simulink model "DynamicsAaa"  (R2017a)
settings: Solver=VariableStepAuto  StartTime=0.0  StopTime=200  RelTol=1e-3
(part 2 of 8)

== matlab function DynamicsAaa/torque ==
  data: q input; qd input; q_des input; torque output; q_des_dot input; q_des_ddot input
function torque = fcn(q,qd,q_des,q_des_dot,q_des_ddot)
%#codegen

%% Constant
% syms qd(1) qd(2) qd(3) qd(4) qd(5) qd(6)
% syms qdd(1) qdd(2) qdd(3) qdd(4) qdd(5) qdd(6)

g = 9.8;


m2=26.9797
m3=15.9204
m4=25.8524
m5=4.08846
m6=1.61544
m7=0.0160103

Kp = 20;
Kd = 10;
%% Triangle relative

c1 = cos(q(1));
c2 = cos(q(2));
c3 = cos(q(3));
c4 = cos(q(4));
c5 = cos(q(5));
c6 = cos(q(6));
s1 = sin(q(1));
s2 = sin(q(2));
s3 = sin(q(3));
s4 = sin(q(4));
s5 = sin(q(5));
s6 = sin(q(6));
c23 = cos(q(2)+q(3)); 
c12 = cos(q(1)+q(2)); 
s23 = sin(q(2)+q(3));
s123 = sin(q(1)+q(2)+q(3));
c123 = cos(q(1)+q(2)+q(3));
c1 = cos(q(1));
c2 = cos(q(2));
c3 = cos(q(3));
c23 = cos(q(2)+q(3)); 
c12 = cos(q(1)+q(2)); 
s1 = sin(q(1));
s2 = sin(q(2));
s3 = sin(q(3));
s23 = sin(q(2)+q(3));
s123 = sin(q(1)+q(2)+q(3));
c123 = cos(q(1)+q(2)+q(3));
%% tau
% tau0 = 0;
% 
% tau1 = -335*c2*(c3*(c4*(c5*m7*(80*c6*(-c5*(-qdd(3) + qdd(4)) - qd(5)*(c5*(-c3*s4*(qd(1) + qd(2)) + c4*s3*(qd(1) + qd(2))) - s5*(-qd(3) + qd(4))) - s5*(c4*(c3*qd(3)*(qd(1) + qd(2)) + s3*(qdd(1) + qdd(2))) + qd(4)*(-c3*c4*(qd(1) + qd(2)) - s3*s4*(qd(1) + qd(2))) - s4*(c3*(qdd(1) + qdd(2)) - qd(3)*s3*(qd(1) + qd(2))))) + c6*(80*c5*(-qdd(3) + qdd(4)) + c5*(c4*(-295*c3*(qdd(1) + qdd(2)) + c3*(c2*(-g*s1 - 270*qd(1)^2) + s2*(-c1*g + 270*qdd(1)) - (qd(1) + qd(2))*(90*qd(1) + 90*qd(2)))) - s4*(295*s3*(qdd(1) + qdd(2)) - s3*(c2*(-g*s1 - 270*qd(1)^2) + s2*(-c1*g + 270*qdd(1)) - (qd(1) + qd(2))*(90*qd(1) + 90*qd(2))))) + 80*qd(5)*(c5*(-c3*s4*(qd(1) + qd(2)) + c4*s3*(qd(1) + qd(2))) - s5*(-qd(3) + qd(4))) + 80*s5*(c4*(c3*qd(3)*(qd(1) + qd(2)) + s3*(qdd(1) + qdd(2))) + qd(4)*(-c3*c4*(qd(1) + qd(2)) - s3*s4*(qd(1) + qd(2))) - s4*(c3*(qdd(1) + qdd(2)) - qd(3)*s3*(qd(1) + qd(2)))) - s5*(-c2*(-c1*g + 270*qdd(1)) - 295*c3^2*(qd(1) + qd(2))^2 - 90*qdd(1) - 90*qdd(2) + s2*(-g*s1 - 270*qd(1)^2) - 295*s3^2*(qd(1) + qd(2))^2) - (80*c5*(-c3*s4*(qd(1) + qd(2)) + c4*s3*(qd(1) + qd(2))) - 80*s5*(-qd(3) + qd(4)))*(-c3*c4*(qd(1) + qd(2)) + qd(5) - s3*s4*(qd(1) + qd(2)))) + 80*qd(6)*(c6*(c5*(-c3*s4*(qd(1) + qd(2)) + c4*s3*(qd(1) + qd(2))) - s5*(-qd(3) + qd(4))) - s6*(-c5*(-qd(3) + qd(4)) - s5*(-c3*s4*(qd(1) + qd(2)) + c4*s3*(qd(1) + qd(2))))) + 80*s6*(c5*(c4*(c3*qd(3)*(qd(1) + qd(2)) + s3*(qdd(1) + qdd(2))) + qd(4)*(-c3*c4*(qd(1) + qd(2)) - s3*s4*(qd(1) + qd(2))) - s4*(c3*(qdd(1) + qdd(2)) - qd(3)*s3*(qd(1) + qd(2)))) + qd(5)*(-c5*(-qd(3) + qd(4)) - s5*(-c3*s4*(qd(1) + qd(2)) + c4*s3*(qd(1) + qd(2)))) - s5*(-qdd(3) + qdd(4))) - s6*(80*c5*(c4*(c3*qd(3)*(qd(1) + qd(2)) + s3*(qdd(1) + qdd(2))) + qd(4)*(-c3*c4*(qd(1) + qd(2)) - s3*s4*(qd(1) + qd(2))) - s4*(c3*(qdd(1) + qdd(2)) - qd(3)*s3*(qd(1) + qd(2)))) - c5*(-c2*(-c1*g + 270*qdd(1)) - 295*c3^2*(qd(1) + qd(2))^2 - 90*qdd(1) - 90*qdd(2) + s2*(-g*s1 - 270*qd(1)^2) - 295*s3^2*(qd(1) + qd(2))^2) + 80*qd(5)*(-c5*(-qd(3) + qd(4)) - s5*(-c3*s4*(qd(1) + qd(2)) + c4*s3*(qd(1) + qd(2)))) - 80*s5*(-qdd(3) + qdd(4)) - s5*(c4*(-295*c3*(qdd(1) + qdd(2)) + c3*(c2*(-g*s1 - 270*qd(1)^2) + s2*(-c1*g + 270*qdd(1)) - (qd(1) + qd(2))*(90*qd(1) + 90*qd(2)))) - s4*(295*s3*(qdd(1) + qdd(2)) - s3*(c2*(-g*s1 - 270*qd(1)^2) + s2*(-c1*g + 270*qdd(1)) - (qd(1) + qd(2))*(90*qd(1) + 90*qd(2))))) + (80*c5*(-qd(3) + qd(4)) + 80*s5*(-c3*s4*(qd(1) + qd(2)) + c4*s3*(qd(1) + qd(2))))*(-c3*c4*(qd(1) + qd(2)) + qd(5) - s3*s4*(qd(1) + qd(2)))) - (80*c6*(c5*(-c3*s4*(qd(1) + qd(2)) + c4*s3*(qd(1) + qd(2))) - s5*(-qd(3) + qd(4))) - 80*s6*(-c5*(-qd(3) + qd(4)) - s5*(-c3*s4*(qd(1) + qd(2)) + c4*s3*(qd(1) + qd(2)))))*(c3*c4*(qd(1) + qd(2)) - qd(5) + qd(6) + s3*s4*(qd(1) + qd(2)))) + m6*(c5*(c4*(-295*c3*(qdd(1) + qdd(2)) + c3*(c2*(-g*s1 - 270*qd(1)^2) + s2*(-c1*g + 270*qdd(1)) - (qd(1) + qd(2))*(90*qd(1) + 90*qd(2)))) - s4*(295*s3*(qdd(1) + qdd(2)) - s3*(c2*(-g*s1 - 270*qd(1)^2) + s2*(-c1*g + 270*qdd(1)) - (qd(1) + qd(2))*(90*qd(1) + 90*qd(2))))) - s5*(-c2*(-c1*g + 270*qdd(1)) - 295*c3^2*(qd(1) + qd(2))^2 - 90*qdd(1) - 90*qdd(2) + s2*(-g*s1 - 270*qd(1)^2) - 295*s3^2*(qd(1) + qd(2))^2)) - m7*s5*(80*c6*(c5*(c4*(c3*qd(3)*(qd(1) + qd(2)) + s3*(qdd(1) + qdd(2))) + qd(4)*(-c3*c4*(qd(1) + qd(2)) - s3*s4*(qd(1) + qd(2))) - s4*(c3*(qdd(1) + qdd(2)) - qd(3)*s3*(qd(1) + qd(2)))) + qd(5)*(-c5*(-qd(3) + qd(4)) - s5*(-c3*s4*(qd(1) + qd(2)) + c4*s3*(qd(1) + qd(2)))) - s5*(-qdd(3) + qdd(4))) - c6*(80*c5*(c4*(c3*qd(3)*(qd(1) + qd(2)) + s3*(qdd(1) + qdd(2))) + qd(4)*(-c3*c4*(qd(1) + qd(2)) - s3*s4*(qd(1) + qd(2))) - s4*(c3*(qdd(1) + qdd(2)) - qd(3)*s3*(qd(1) + qd(2)))) - c5*(-c2*(-c1*g + 270*qdd(1)) - 295*c3^2*(qd(1) + qd(2)) ^2 - 90*qdd(1) - 90*qdd(2) + s2*(-g*s1 - 270*qd(1)^2) - 295*s3^2*(qd(1) + qd(2)) ^2) + 80*qd(5)*(-c5*(-qd(3) + qd(4)) - s5*(-c3*s4*(qd(1) + qd(2)) + c4*s3*(qd(1) + qd(2)))) - 80*s5*(-qdd(3) + qdd(4)) - s5*(c4*(-295*c3*(qdd(1) + qdd(2)) + c3*(c2*(-g*s1 - 270*qd(1)^2) + s2*(-c1*g + 270*qdd(1)) - (qd(1) + qd(2))*(90*qd(1) + 90*qd(2)))) - s4*(295*s3*(qdd(1) + qdd(2)) - s3*(c2*(-g*s1 - 270*qd(1)^2) + s2*(-c1*g + 270*qdd(1)) - (qd(1) + qd(2))*(90*qd(1) + 90*qd(2))))) + (80*c5*(-qd(3) + qd(4)) + 80*s5*(-c3*s4*(qd(1) + qd(2)) + c4*s3*(qd(1) + qd(2))))*(-c3*c4*(qd(1) + qd(2)) + qd(5) - s3*s4*(qd(1) + qd(2)))) + 80*qd(6)*(-c6*(-c5*(-qd(3) + qd(4)) - s5*(-c3*s4*(qd(1) + qd(2)) + c4*s3*(qd(1) + qd(2)))) - s6*(c5*(-c3*s4*(qd(1) + qd(2)) + c4*s3*(qd(1) + qd(2))) - s5*(-qd(3) + qd(4)))) - 80*s6*(-c5*(-qdd(3) + qdd(4)) - qd(5)*(c5*(-c3*s4*(qd(1) + qd(2)) + c4*s3*(qd(1) + qd(2))) - s5*(-qd(3) + qd(4))) - s5*(c4*(c3*qd(3)*(qd(1) + qd(2)) + s3*(qdd(1) + qdd(2))) + qd(4)*(-c3*c4*(qd(1) + qd(2)) - s3*s4*(qd(1) + qd(2))) - s4*(c3*(qdd(1) + qdd(2)) - qd(3)*s3*(qd(1) + qd(2))))) - s6*(80*c5*(-qdd(3) + qdd(4)) + c5*(c4*(-295*c3*(qdd(1) + qdd(2)) + c3*(c2*(-g*s1 - 270*qd(1)^2) + s2*(-c1*g + 270*qdd(1)) - (qd(1) + qd(2))*(90*qd(1) + 90*qd(2)))) - s4*(295*s3*(qdd(1) + qdd(2)) - s3*(c2*(-g*s1 - 270*qd(1)^2) + s2*(-c1*g + 270*qdd(1)) - (qd(1) + qd(2))*(90*qd(1) + 90*qd(2))))) + 80*qd(5)*(c5*(-c3*s4*(qd(1) + qd(2)) + c4*s3*(qd(1) + qd(2))) - s5*(-qd(3) + qd(4))) + 80*s5*(c4*(c3*qd(3)*(qd(1) + qd(2)) + s3*(qdd(1) + qdd(2))) + qd(4)*(-c3*c4*(qd(1) + qd(2)) - s3*s4*(qd(1) + qd(2))) - s4*(c3*(qdd(1) + qdd(2)) - qd(3)*s3*(qd(1) + qd(2)))) - s5*(-c2*(-c1*g + 270*qdd(1)) - 295*c3^2*(qd(1) + qd(2)) ^2 - 90*qdd(1) - 90*qdd(2) + s2*(-g*s1 - 270*qd(1)^2) - 295*s3^2*(qd(1) + qd(2)) ^2) - (80*c5*(-c3*s4*(qd(1) + qd(2)) + c4*s3*(qd(1) + qd(2))) - 80*s5*(-qd(3) + qd(4)))*(-c3*c4*(qd(1) + qd(2)) + qd(5) - s3*s4*(qd(1) + qd(2)))) + (80*c6*(-c5*(-qd(3) + qd(4)) - s5*(-c3*s4*(qd(1) + qd(2)) + c4*s3*(qd(1) + qd(2)))) + 80*s6*(c5*(-c3*s4*(qd(1) + qd(2)) + c4*s3*(qd(1) + qd(2))) - s5*(-qd(3) + qd(4))))*(c3*c4*(qd(1) + qd(2)) - qd(5) + qd(6) + s3*s4*(qd(1) + qd(2))))) + m5*(c4*(-295*c3*(qdd(1) + qdd(2)) + c3*(c2*(-g*s1 - 270*qd(1)^2) + s2*(-c1*g + 270*qdd(1)) - (qd(1) + qd(2))*(90*qd(1) + 90*qd(2)))) + 295*c4*(c3*(qdd(1) + qdd(2)) - qd(3)*s3*(qd(1) + qd(2))) + 295*qd(4)*(-c3*s4*(qd(1) + qd(2)) + c4*s3*(qd(1) + qd(2))) - s4*(295*s3*(qdd(1) + qdd(2)) - s3*(c2*(-g*s1 - 270*qd(1)^2) + s2*(-c1*g + 270*qdd(1)) - (qd(1) + qd(2))*(90*qd(1) + 90*qd(2)))) + 295*s4*(c3*qd(3)*(qd(1) + qd(2)) + s3*(qdd(1) + qdd(2))) - (-qd(3) + qd(4))*(-295*c3*s4*(qd(1) + qd(2)) + 295*c4*s3*(qd(1) + qd(2)))) - s4*(m6*(-c5*(-c2*(-c1*g + 270*qdd(1)) - 295*c3^2*(qd(1) + qd(2)) ^2 - 90*qdd(1) - 90*qdd(2) + s2*(-g*s1 - 270*qd(1)^2) - 295*s3^2*(qd(1) + qd(2)) ^2) - s5*(c4*(-295*c3*(qdd(1) + qdd(2)) + c3*(c2*(-g*s1 - 270*qd(1)^2) + s2*(-c1*g + 270*qdd(1)) - (qd(1) + qd(2))*(90*qd(1) + 90*qd(2)))) - s4*(295*s3*(qdd(1) + qdd(2)) - s3*(c2*(-g*s1 - 270*qd(1)^2) + s2*(-c1*g + 270*qdd(1)) - (qd(1) + qd(2))*(90*qd(1) + 90*qd(2)))))) + m7*(c4*(295*s3*(qdd(1) + qdd(2)) - s3*(c2*(-g*s1 - 270*qd(1)^2) + s2*(-c1*g + 270*qdd(1)) - (qd(1) + qd(2))*(90*qd(1) + 90*qd(2)))) + s4*(-295*c3*(qdd(1) + qdd(2)) + c3*(c2*(-g*s1 - 270*qd(1)^2) + s2*(-c1*g + 270*qdd(1)) - (qd(1) + qd(2))*(90*qd(1) + 90*qd(2)))) + (-c5*(-qd(3) + qd(4)) - s5*(-c3*s4*(qd(1) + qd(2)) + c4*s3*(qd(1) + qd(2))))*(80*c5*(-qd(3) + qd(4)) + 80*s5*(-c3*s4*(qd(1) + qd(2)) + c4*s3*(qd(1) + qd(2)))) - (c5*(-c3*s4*(qd(1) + qd(2)) + c4*s3*(qd(1) + qd(2))) - s5*(-qd(3) + qd(4)))*(80*c5*(-c3*s4*(qd(1) + qd(2)) + c4*s3*(qd(1) + qd(2))) - 80*s5*(-qd(3) + qd(4))) - (-c6*(-c5*(-qd(3) + qd(4)) - s5*(-c3*s4*(qd(1) + qd(2)) + c4*s3*(qd(1) + qd(2)))) - s6*(c5*(-c3*s4*(qd(1) + qd(2)) + c4*s3*(qd(1) + qd(2))) - s5*(-qd(3) + qd(4))))*(80*c6*(-c5*(-qd(3) + qd(4)) - s5*(-c3*s4*(qd(1) + qd(2)) + c4*s3*(qd(1) + qd(2)))) + 80*s6*(c5*(-c3*s4*(qd(1) + qd(2)) + c4*s3*(qd(1) + qd(2))) - s5*(-qd(3) + qd(4)))) + (c6*(c5*(-c3*s4*(qd(1) + qd(2)) + c4*s3*(qd(1) + qd(2))) - s5*(-qd(3) + qd(4))) - s6*(-c5*(-qd(3) + qd(4)) - s5*(-c3*s4*(qd(1) + qd(2)) + c4*s3*(qd(1) + qd(2)))))*(80*c6*(c5*(-c3*s4*(qd(1) + qd(2)) + c4*s3*(qd(1) + qd(2))) - s5*(-qd(3) + qd(4))) - 80*s6*(-c5*(-qd(3) + qd(4)) - s5*(-c3*s4*(qd(1) + qd(2)) + c4*s3*(qd(1) + qd(2)))))))) + m4*(-90*c3^2*(qd(1) + qd(2)) ^2 + c3*(c2*(-g*s1 - 270*qd(1)^2) + s2*(-c1*g + 270*qdd(1)) - (qd(1) + qd(2))*(90*qd(1) + 90*qd(2))) - 90*qd(3)^2) - s3*(-c4*(m6*(-c5*(-c2*(-c1*g + 270*qdd(1)) - 295*c3^2*(qd(1) + qd(2)) ^2 - 90*qdd(1) - 90*qdd(2) + s2*(-g*s1 - 270*qd(1)^2) - 295*s3^2*(qd(1) + qd(2)) ^2) - s5*(c4*(-295*c3*(qdd(1) + qdd(2)) + c3*(c2*(-g*s1 - 270*qd(1)^2) + s2*(-c1*g + 270*qdd(1)) - (qd(1) + qd(2))*(90*qd(1) + 90*qd(2)))) - s4*(295*s3*(qdd(1) + qdd(2)) - s3*(c2*(-g*s1 - 270*qd(1)^2) + s2*(-c1*g + 270*qdd(1)) - (qd(1) + qd(2))*(90*qd(1) + 90*qd(2)))))) + m7*(c4*(295*s3*(qdd(1) + qdd(2)) - s3*(c2*(-g*s1 - 270*qd(1)^2) + s2*(-c1*g + 270*qdd(1)) - (qd(1) + qd(2))*(90*qd(1) + 90*qd(2)))) + s4*(-295*c3*(qdd(1) + qdd(2)) + c3*(c2*(-g*s1 - 270*qd(1)^2) + s2*(-c1*g + 270*qdd(1)) - (qd(1) + qd(2))*(90*qd(1) + 90*qd(2)))) + (-c5*(-qd(3) + qd(4)) - s5*(-c3*s4*(qd(1) + qd(2)) + c4*s3*(qd(1) + qd(2))))*(80*c5*(-qd(3) + qd(4)) + 80*s5*(-c3*s4*(qd(1) + qd(2)) + c4*s3*(qd(1) + qd(2)))) - (c5*(-c3*s4*(qd(1) + qd(2)) + c4*s3*(qd(1) + qd(2))) - s5*(-qd(3) + qd(4)))*(80*c5*(-c3*s4*(qd(1) + qd(2)) + c4*s3*(qd(1) + qd(2))) - 80*s5*(-qd(3) + qd(4))) - (-c6*(-c5*(-qd(3) + qd(4)) - s5*(-c3*s4*(qd(1) + qd(2)) + c4*s3*(qd(1) + qd(2)))) - s6*(c5*(-c3*s4*(qd(1) + qd(2)) + c4*s3*(qd(1) + qd(2))) - s5*(-qd(3) + qd(4))))*(80*c6*(-c5*(-qd(3) + qd(4)) - s5*(-c3*s4*(qd(1) + qd(2)) + c4*s3*(qd(1) + qd(2)))) + 80*s6*(c5*(-c3*s4*(qd(1) + qd(2)) + c4*s3*(qd(1) + qd(2))) - s5*(-qd(3) + qd(4)))) + (c6*(c5*(-c3*s4*(qd(1) + qd(2)) + c4*s3*(qd(1) + qd(2))) - s5*(-qd(3) + qd(4))) - s6*(-c5*(-qd(3) + qd(4)) - s5*(-c3*s4*(qd(1) + qd(2)) + c4*s3*(qd(1) + qd(2)))))*(80*c6*(c5*(-c3*s4*(qd(1) + qd(2)) + c4*s3*(qd(1) + qd(2))) - s5*(-qd(3) + qd(4))) - 80*s6*(-c5*(-qd(3) + qd(4)) - s5*(-c3*s4*(qd(1) + qd(2)) + c4*s3*(qd(1) + qd(2))))))) + m5*(-c4*(295*s3*(qdd(1) + qdd(2)) - s3*(c2*(-g*s1 - 270*qd(1)^2) + s2*(-c1*g + 270*qdd(1)) - (qd(1) + qd(2))*(90*qd(1) + 90*qd(2)))) + 295*c4*(c3*qd(3)*(qd(1) + qd(2)) + s3*(qdd(1) + qdd(2))) + 295*qd(4)*(-c3*c4*(qd(1) + qd(2)) - s3*s4*(qd(1) + qd(2))) - s4*(-295*c3*(qdd(1) + qdd(2)) + c3*(c2*(-g*s1 - 270*qd(1)^2) + s2*(-c1*g + 270*qdd(1)) - (qd(1) + qd(2))*(90*qd(1) + 90*qd(2)))) - 295*s4*(c3*(qdd(1) + qdd(2)) - qd(3)*s3*(qd(1) + qd(2))) + (-qd(3) + qd(4))*(295*c3*c4*(qd(1) + qd(2)) + 295*s3*s4*(qd(1) + qd(2)))) - s4*(c5*m7*(80*c6*(-c5*(-qdd(3) + qdd(4)) - qd(5)*(c5*(-c3*s4*(qd(1) + qd(2)) + c4*s3*(qd(1) + qd(2))) - s5*(-qd(3) + qd(4))) - s5*(c4*(c3*qd(3)*(qd(1) + qd(2)) + s3*(qdd(1) + qdd(2))) + qd(4)*(-c3*c4*(qd(1) + qd(2)) - s3*s4*(qd(1) + qd(2))) - s4*(c3*(qdd(1) + qdd(2)) - qd(3)*s3*(qd(1) + qd(2))))) + c6*(80*c5*(-qdd(3) + qdd(4)) + c5*(c4*(-295*c3*(qdd(1) + qdd(2)) + c3*(c2*(-g*s1 - 270*qd(1)^2) + s2*(-c1*g + 270*qdd(1)) - (qd(1) + qd(2))*(90*qd(1) + 90*qd(2)))) - s4*(295*s3*(qdd(1) + qdd(2)) - s3*(c2*(-g*s1 - 270*qd(1)^2) + s2*(-c1*g + 270*qdd(1)) - (qd(1) + qd(2))*(90*qd(1) + 90*qd(2))))) + 80*qd(5)*(c5*(-c3*s4*(qd(1) + qd(2)) + c4*s3*(qd(1) + qd(2))) - s5*(-qd(3) + qd(4))) + 80*s5*(c4*(c3*qd(3)*(qd(1) + qd(2)) + s3*(qdd(1) + qdd(2))) + qd(4)*(-c3*c4*(qd(1) + qd(2)) - s3*s4*(qd(1) + qd(2))) - s4*(c3*(qdd(1) + qdd(2)) - qd(3)*s3*(qd(1) + qd(2)))) - s5*(-c2*(-c1*g + 270*qdd(1)) - 295*c3^2*(qd(1) + qd(2)) ^2 - 90*qdd(1) - 90*qdd(2) + s2*(-g*s1 - 270*qd(1)^2) - 295*s3^2*(qd(1) + qd(2)) ^2) - (80*c5*(-c3*s4*(qd(1) + qd(2)) + c4*s3*(qd(1) + qd(2))) - 80*s5*(-qd(3) + qd(4)))*(-c3*c4*(qd(1) + qd(2)) + qd(5) - s3*s4*(qd(1) + qd(2)))) + 80*qd(6)*(c6*(c5*(-c3*s4*(qd(1) + qd(2)) + c4*s3*(qd(1) + qd(2))) - s5*(-qd(3) + qd(4))) - s6*(-c5*(-qd(3) + qd(4)) - s5*(-c3*s4*(qd(1) + qd(2)) + c4*s3*(qd(1) + qd(2))))) + 80*s6*(c5*(c4*(c3*qd(3)*(qd(1) + qd(2)) + s3*(qdd(1) + qdd(2))) + qd(4)*(-c3*c4*(qd(1) + qd(2)) - s3*s4*(qd(1) + qd(2))) - s4*(c3*(qdd(1) + qdd(2)) - qd(3)*s3*(qd(1) + qd(2)))) + qd(5)*(-c5*(-qd(3) + qd(4)) - s5*(-c3*s4*(qd(1) + qd(2)) + c4*s3*(qd(1) + qd(2)))) - s5*(-qdd(3) + qdd(4))) - s6*(80*c5*(c4*(c3*qd(3)*(qd(1) + qd(2)) + s3*(qdd(1) + qdd(2))) + qd(4)*(-c3*c4*(qd(1) + qd(2)) - s3*s4*(qd(1) + qd(2))) - s4*(c3*(qdd(1) + qdd(2)) - qd(3)*s3*(qd(1) + qd(2)))) - c5*(-c2*(-c1*g + 270*qdd(1)) - 295*c3^2*(qd(1) + qd(2)) ^2 - 90*qdd(1) - 90*qdd(2) + s2*(-g*s1 - 270*qd(1)^2) - 295*s3^2*(qd(1) + qd(2)) ^2) + 80*qd(5)*(-c5*(-qd(3) + qd(4)) - s5*(-c3*s4*(qd(1) + qd(2)) + c4*s3*(qd(1) + qd(2)))) - 80*s5*(-qdd(3) + qdd(4)) - s5*(c4*(-295*c3*(qdd(1) + qdd(2)) + c3*(c2*(-g*s1 - 270*qd(1)^2) + s2*(-c1*g + 270*qdd(1)) - (qd(1) + qd(2))*(90*qd(1) + 90*qd(2)))) - s4*(295*s3*(qdd(1) + qdd(2)) - s3*(c2*(-g*s1 - 270*qd(1)^2) + s2*(-c1*g + 270*qdd(1)) - (qd(1) + qd(2))*(90*qd(1) + 90*qd(2))))) + (80*c5*(-qd(3) + qd(4)) + 80*s5*(-c3*s4*(qd(1) + qd(2)) + c4*s3*(qd(1) + qd(2))))*(-c3*c4*(qd(1) + qd(2)) + qd(5) - s3*s4*(qd(1) + qd(2)))) - (80*c6*(c5*(-c3*s4*(qd(1) + qd(2)) + c4*s3*(qd(1) + qd(2))) - s5*(-qd(3) + qd(4))) - 80*s6*(-c5*(-qd(3) + qd(4)) - s5*(-c3*s4*(qd(1) + qd(2)) + c4*s3*(qd(1) + qd(2)))))*(c3*c4*(qd(1) + qd(2)) - qd(5) + qd(6) + s3*s4*(qd(1) + qd(2)))) + m6*(c5*(c4*(-295*c3*(qdd(1) + qdd(2)) + c3*(c2*(-g*s1 - 270*qd(1)^2) + s2*(-c1*g + 270*qdd(1)) - (qd(1) + qd(2))*(90*qd(1) + 90*qd(2)))) - s4*(295*s3*(qdd(1) + qdd(2)) - s3*(c2*(-g*s1 - 270*qd(1)^2) + s2*(-c1*g + 270*qdd(1)) - (qd(1) + qd(2))*(90*qd(1) + 90*qd(2))))) - s5*(-c2*(-c1*g + 270*qdd(1)) - 295*c3^2*(qd(1) + qd(2)) ^2 - 90*qdd(1) - 90*qdd(2) + s2*(-g*s1 - 270*qd(1)^2) - 295*s3^2*(qd(1) + qd(2)) ^2)) - m7*s5*(80*c6*(c5*(c4*(c3*qd(3)*(qd(1) + qd(2)) + s3*(qdd(1) + qdd(2))) + qd(4)*(-c3*c4*(qd(1) + qd(2)) - s3*s4*(qd(1) + qd(2))) - s4*(c3*(qdd(1) + qdd(2)) - qd(3)*s3*(qd(1) + qd(2)))) + qd(5)*(-c5*(-qd(3) + qd(4)) - s5*(-c3*s4*(qd(1) + qd(2)) + c4*s3*(qd(1) + qd(2)))) - s5*(-qdd(3) + qdd(4))) - c6*(80*c5*(c4*(c3*qd(3)*(qd(1) + qd(2)) + s3*(qdd(1) + qdd(2))) + qd(4)*(-c3*c4*(qd(1) + qd(2)) - s3*s4*(qd(1) + qd(2))) - s4*(c3*(qdd(1) + qdd(2)) - qd(3)*s3*(qd(1) + qd(2)))) - c5*(-c2*(-c1*g + 270*qdd(1)) - 295*c3^2*(qd(1) + qd(2)) ^2 - 90*qdd(1) - 90*qdd(2) + s2*(-g*s1 - 270*qd(1)^2) - 295*s3^2*(qd(1) + qd(2)) ^2) + 80*qd(5)*(-c5*(-qd(3) + qd(4)) - s5*(-c3*s4*(qd(1) + qd(2)) + c4*s3*(qd(1) + qd(2)))) - 80*s5*(-qdd(3) + qdd(4)) - s5*(c4*(-295*c3*(qdd(1) + qdd(2)) + c3*(c2*(-g*s1 - 270*qd(1)^2) + s2*(-c1*g + 270*qdd(1)) - (qd(1) + qd(2))*(90*qd(1) + 90*qd(2)))) - s4*(295*s3*(qdd(1) + qdd(2)) - s3*(c2*(-g*s1 - 270*qd(1)^2) + s2*(-c1*g + 270*qdd(1)) - (qd(1) + qd(2))*(90*qd(1) + 90*qd(2))))) + (80*c5*(-qd(3) + qd(4)) + 80*s5*(-c3*s4*(qd(1) + qd(2)) + c4*s3*(qd(1) + qd(2))))*(-c3*c4*(qd(1) + qd(2)) + qd(5) - s3*s4*(qd(1) + qd(2)))) + 80*qd(6)*(-c6*(-c5*(-qd(3) + qd(4)) - s5*(-c3*s4*(qd(1) + qd(2)) + c4*s3*(qd(1) + qd(2)))) - s6*(c5*(-c3*s4*(qd(1) + qd(2)) + c4*s3*(qd(1) + qd(2))) - s5*(-qd(3) + qd(4)))) - 80*s6*(-c5*(-qdd(3) + qdd(4)) - qd(5)*(c5*(-c3*s4*(qd(1) + qd(2)) + c4*s3*(qd(1) + qd(2))) - s5*(-qd(3) + qd(4))) - s5*(c4*(c3*qd(3)*(qd(1) + qd(2)) + s3*(qdd(1) + qdd(2))) + qd(4)*(-c3*c4*(qd(1) + qd(2)) - s3*s4*(qd(1) + qd(2))) - s4*(c3*(qdd(1) + qdd(2)) - qd(3)*s3*(qd(1) + qd(2))))) - s6*(80*c5*(-qdd(3) + qdd(4)) + c5*(c4*(-295*c3*(qdd(1) + qdd(2)) + c3*(c2*(-g*s1 - 270*qd(1)^2) + s2*(-c1*g + 270*qdd(1)) - (qd(1) + qd(2))*(90*qd(1) + 90*qd(2)))) - s4*(295*s3*(qdd(1) + qdd(2)) - s3*(c2*(-g*s1 - 270*qd(1)^2) + s2*(-c1*g + 270*qdd(1)) - (qd(1) + qd(2))*(90*qd(1) + 90*qd(2))))) + 80*qd(5)*(c5*(-c3*s4*(qd(1) + qd(2)) + c4*s3*(qd(1) + qd(2))) - s5*(-qd(3) + qd(4))) + 80*s5*(c4*(c3*qd(3)*(qd(1) + qd(2)) + s3*(qdd(1) + qdd(2))) + qd(4)*(-c3*c4*(qd(1) + qd(2)) - s3*s4*(qd(1) + qd(2))) - s4*(c3*(qdd(1) + qdd(2)) - qd(3)*s3*(qd(1) + qd(2)))) - s5*(-c2*(-c1*g + 270*qdd(1)) - 295*c3^2*(qd(1) + qd(2)) ^2 - 90*qdd(1) - 90*qdd(2) + s2*(-g*s1 - 270*qd(1)^2) - 295*s3^2*(qd(1) + qd(2)) ^2) - (80*c5*(-c3*s4*(qd(1) + qd(2)) + c4*s3*(qd(1) + qd(2))) - 80*s5*(-qd(3) + qd(4)))*(-c3*c4*(qd(1) + qd(2)) + qd(5) - s3*s4*(qd(1) + qd(2)))) + (80*c6*(-c5*(-qd(3) + qd(4)) - s5*(-c3*s4*(qd(1) + qd(2)) + c4*s3*(qd(1) + qd(2)))) + 80*s6*(c5*(-c3*s4*(qd(1) + qd(2)) + c4*s3*(qd(1) + qd(2))) - s5*(-qd(3) + qd(4))))*(c3*c4*(qd(1) + qd(2)) - qd(5) + qd(6) + s3*s4*(qd(1) + qd(2))))))) + 75*c2*(c5*m7*(80*c6*(c5*(c4*(c3*qd(3)*(qd(1) + qd(2)) + s3*(qdd(1) + qdd(2))) + qd(4)*(-c3*c4*(qd(1) + qd(2)) - s3*s4*(qd(1) + qd(2))) - s4*(c3*(qdd(1) + qdd(2)) - qd(3)*s3*(qd(1) + qd(2)))) + qd(5)*(-c5*(-qd(3) + qd(4)) - s5*(-c3*s4*(qd(1) + qd(2)) + c4*s3*(qd(1) + qd(2)))) - s5*(-qdd(3) + qdd(4))) - c6*(80*c5*(c4*(c3*qd(3)*(qd(1) + qd(2)) + s3*(qdd(1) + qdd(2))) + qd(4)*(-c3*c4*(qd(1) + qd(2)) - s3*s4*(qd(1) + qd(2))) - s4*(c3*(qdd(1) + qdd(2)) - qd(3)*s3*(qd(1) + qd(2)))) - c5*(-c2*(-c1*g + 270*qdd(1)) - 295*c3^2*(qd(1) + qd(2)) ^2 - 90*qdd(1) - 90*qdd(2) + s2*(-g*s1 - 270*qd(1)^2) - 295*s3^2*(qd(1) + qd(2)) ^2) + 80*qd(5)*(-c5*(-qd(3) + qd(4)) - s5*(-c3*s4*(qd(1) + qd(2)) + c4*s3*(qd(1) + qd(2)))) - 80*s5*(-qdd(3) + qdd(4)) - s5*(c4*(-295*c3*(qdd(1) + qdd(2)) + c3*(c2*(-g*s1 - 270*qd(1)^2) + s2*(-c1*g + 270*qdd(1)) - (qd(1) + qd(2))*(90*qd(1) + 90*qd(2)))) - s4*(295*s3*(qdd(1) + qdd(2)) - s3*(c2*(-g*s1 - 270*qd(1)^2) + s2*(-c1*g + 270*qdd(1)) - (qd(1) + qd(2))*(90*qd(1) + 90*qd(2))))) + (80*c5*(-qd(3) + qd(4)) + 80*s5*(-c3*s4*(qd(1) + qd(2)) + c4*s3*(qd(1) + qd(2))))*(-c3*c4*(qd(1) + qd(2)) + qd(5) - s3*s4*(qd(1) + qd(2)))) + 80*qd(6)*(-c6*(-c5*(-qd(3) + qd(4)) - s5*(-c3*s4*(qd(1) + qd(2)) + c4*s3*(qd(1) + qd(2)))) - s6*(c5*(-c3*s4*(qd(1) + qd(2)) + c4*s3*(qd(1) + qd(2))) - s5*(-qd(3) + qd(4)))) - 80*s6*(-c5*(-qdd(3) + qdd(4)) - qd(5)*(c5*(-c3*s4*(qd(1) + qd(2)) + c4*s3*(qd(1) + qd(2))) - s5*(-qd(3) + qd(4))) - s5*(c4*(c3*qd(3)*(qd(1) + qd(2)) + s3*(qdd(1) + qdd(2))) + qd(4)*(-c3*c4*(qd(1) + qd(2)) - s3*s4*(qd(1) + qd(2))) - s4*(c3*(qdd(1) + qdd(2)) - qd(3)*s3*(qd(1) + qd(2))))) - s6*(80*c5*(-qdd(3) + qdd(4)) + c5*(c4*(-295*c3*(qdd(1) + qdd(2)) + c3*(c2*(-g*s1 - 270*qd(1)^2) + s2*(-c1*g + 270*qdd(1)) - (qd(1) + qd(2))*(90*qd(1) + 90*qd(2)))) - s4*(295*s3*(qdd(1) + qdd(2)) - s3*(c2*(-g*s1 - 270*qd(1)^2) + s2*(-c1*g + 270*qdd(1)) - (qd(1) + qd(2))*(90*qd(1) + 90*qd(2))))) + 80*qd(5)*(c5*(-c3*s4*(qd(1) + qd(2)) + c4*s3*(qd(1) + qd(2))) - s5*(-qd(3) + qd(4))) + 80*s5*(c4*(c3*qd(3)*(qd(1) + qd(2)) + s3*(qdd(1) + qdd(2))) + qd(4)*(-c3*c4*(qd(1) + qd(2)) - s3*s4*(qd(1) + qd(2))) - s4*(c3*(qdd(1) + qdd(2)) - qd(3)*s3*(qd(1) + qd(2)))) - s5*(-c2*(-c1*g + 270*qdd(1)) - 295*c3^2*(qd(1) + qd(2)) ^2 - 90*qdd(1) - 90*qdd(2) + s2*(-g*s1 - 270*qd(1)^2) - 295*s3^2*(qd(1) + qd(2)) ^2) - (80*c5*(-c3*s4*(qd(1) + qd(2)) + c4*s3*(qd(1) + qd(2))) - 80*s5*(-qd(3) + qd(4)))*(-c3*c4*(qd(1) + qd(2)) + qd(5) - s3*s4*(qd(1) + qd(2)))) + (80*c6*(-c5*(-qd(3) + qd(4)) - s5*(-c3*s4*(qd(1) + qd(2)) + c4*s3*(qd(1) + qd(2)))) + 80*s6*(c5*(-c3*s4*(qd(1) + qd(2)) + c4*s3*(qd(1) + qd(2))) - s5*(-qd(3) + qd(4))))*(c3*c4*(qd(1) + qd(2)) - qd(5) + qd(6) + s3*s4*(qd(1) + qd(2)))) + m4*(90*c3*s3*(qd(1) + qd(2))^2 + 90*qdd(3) - s3*(c2*(-g*s1 - 270*qd(1)^2) + s2*(-c1*g + 270*qdd(1)) - (qd(1) + qd(2))*(90*qd(1) + 90*qd(2)))) + m5*(-c2*(-c1*g + 270*qdd(1)) - 295*c3^2*(qd(1) + qd(2))^2 - 90*qdd(1) - 90*qdd(2) + s2*(-g*s1 - 270*qd(1)^2) - 295*s3^2*(qd(1) + qd(2))^2 - (-c3*c4*(qd(1) + qd(2)) - s3*s4*(qd(1) + qd(2)))*(295*c3*c4*(qd(1) + qd(2)) + 295*s3*s4*(qd(1) + qd(2))) + (-295*c3*s4*(qd(1) + qd(2)) + 295*c4*s3*(qd(1) + qd(2)))*(-c3*s4*(qd(1) + qd(2)) + c4*s3*(qd(1) + qd(2)))) - m6*(-c4*(295*s3*(qdd(1) + qdd(2)) - s3*(c2*(-g*s1 - 270*qd(1)^2) + s2*(-c1*g + 270*qdd(1)) - (qd(1) + qd(2))*(90*qd(1) + 90*qd(2)))) - s4*(-295*c3*(qdd(1) + qdd(2)) + c3*(c2*(-g*s1 - 270*qd(1)^2) + s2*(-c1*g + 270*qdd(1)) - (qd(1) + qd(2))*(90*qd(1) + 90*qd(2))))) + m7*s5*(80*c6*(-c5*(-qdd(3) + qdd(4)) - qd(5)*(c5*(-c3*s4*(qd(1) + qd(2)) + c4*s3*(qd(1) + qd(2))) - s5*(-qd(3) + qd(4))) - s5*(c4*(c3*qd(3)*(qd(1) + qd(2)) + s3*(qdd(1) + qdd(2))) + qd(4)*(-c3*c4*(qd(1) + qd(2)) - s3*s4*(qd(1) + qd(2))) - s4*(c3*(qdd(1) + qdd(2)) - qd(3)*s3*(qd(1) + qd(2))))) + c6*(80*c5*(-qdd(3) + qdd(4)) + c5*(c4*(-295*c3*(qdd(1) + qdd(2)) + c3*(c2*(-g*s1 - 270*qd(1)^2) + s2*(-c1*g + 270*qdd(1)) - (qd(1) + qd(2))*(90*qd(1) + 90*qd(2)))) - s4*(295*s3*(qdd(1) + qdd(2)) - s3*(c2*(-g*s1 - 270*qd(1)^2) + s2*(-c1*g + 270*qdd(1)) - (qd(1) + qd(2))*(90*qd(1) + 90*qd(2))))) + 80*qd(5)*(c5*(-c3*s4*(qd(1) + qd(2)) + c4*s3*(qd(1) + qd(2))) - s5*(-qd(3) + qd(4))) + 80*s5*(c4*(c3*qd(3)*(qd(1) + qd(2)) + s3*(qdd(1) + qdd(2))) + qd(4)*(-c3*c4*(qd(1) + qd(2)) - s3*s4*(qd(1) + qd(2))) - s4*(c3*(qdd(1) + qdd(2)) - qd(3)*s3*(qd(1) + qd(2)))) - s5*(-c2*(-c1*g + 270*qdd(1)) - 295*c3^2*(qd(1) + qd(2)) ^2 - 90*qdd(1) - 90*qdd(2) + s2*(-g*s1 - 270*qd(1)^2) - 295*s3^2*(qd(1) + qd(2)) ^2) - (80*c5*(-c3*s4*(qd(1) + qd(2)) + c4*s3*(qd(1) + qd(2))) - 80*s5*(-qd(3) + qd(4)))*(-c3*c4*(qd(1) + qd(2)) + qd(5) - s3*s4*(qd(1) + qd(2)))) + 80*qd(6)*(c6*(c5*(-c3*s4*(qd(1) + qd(2)) + c4*s3*(qd(1) + qd(2))) - s5*(-qd(3) + qd(4))) - s6*(-c5*(-qd(3) + qd(4)) - s5*(-c3*s4*(qd(1) + qd(2)) + c4*s3*(qd(1) + qd(2))))) + 80*s6*(c5*(c4*(c3*qd(3)*(qd(1) + qd(2)) + s3*(qdd(1) + qdd(2))) + qd(4)*(-c3*c4*(qd(1) + qd(2)) - s3*s4*(qd(1) + qd(2))) - s4*(c3*(qdd(1) + qdd(2)) - qd(3)*s3*(qd(1) + qd(2)))) + qd(5)*(-c5*(-qd(3) + qd(4)) - s5*(-c3*s4*(qd(1) + qd(2)) + c4*s3*(qd(1) + qd(2)))) - s5*(-qdd(3) + qdd(4))) - s6*(80*c5*(c4*(c3*qd(3)*(qd(1) + qd(2)) + s3*(qdd(1) + qdd(2))) + qd(4)*(-c3*c4*(qd(1) + qd(2)) - s3*s4*(qd(1) + qd(2))) - s4*(c3*(qdd(1) + qdd(2)) - qd(3)*s3*(qd(1) + qd(2)))) - c5*(-c2*(-c1*g + 270*qdd(1)) - 295*c3^2*(qd(1) + qd(2)) ^2 - 90*qdd(1) - 90*qdd(2) + s2*(-g*s1 - 270*qd(1)^2) - 295*s3^2*(qd(1) + qd(2)) ^2) + 80*qd(5)*(-c5*(-qd(3) + qd(4)) - s5*(-c3*s4*(qd(1) + qd(2)) + c4*s3*(qd(1) + qd(2)))) - 80*s5*(-qdd(3) + qdd(4)) - s5*(c4*(-295*c3*(qdd(1) + qdd(2)) + c3*(c2*(-g*s1 - 270*qd(1)^2) + s2*(-c1*g + 270*qdd(1)) - (qd(1) + qd(2))*(90*qd(1) + 90*qd(2)))) - s4*(295*s3*(qdd(1) + qdd(2)) - s3*(c2*(-g*s1 - 270*qd(1)^2) + s2*(-c1*g + 270*qdd(1)) - (qd(1) + qd(2))*(90*qd(1) + 90*qd(2))))) + (80*c5*(-qd(3) + qd(4)) + 80*s5*(-c3*s4*(qd(1) + qd(2)) + c4*s3*(qd(1) + qd(2))))*(-c3*c4*(qd(1) + qd(2)) + qd(5) - s3*s4*(qd(1) + qd(2)))) - (80*c6*(c5*(-c3*s4*(qd(1) + qd(2)) + c4*s3*(qd(1) + qd(2))) - s5*(-qd(3) + qd(4))) - 80*s6*(-c5*(-qd(3) + qd(4)) - s5*(-c3*s4*(qd(1) + qd(2)) + c4*s3*(qd(1) + qd(2)))))*(c3*c4*(qd(1) + qd(2)) - qd(5) + qd(6) + s3*s4*(qd(1) + qd(2))))) - 0.0247925*c3*qd(3)*(qd(1) + qd(2)) - c3*(qd(1) + qd(2))*(-0.00947011*c3*(qd(1) + qd(2)) - 0.0247925*qd(3) + 0.775113*s3*(qd(1) + qd(2))) - 0.00744338*c3*(qdd(1) + qdd(2)) + c3*(-0.020170031*c4*(c3*(qdd(1) + qdd(2)) - qd(3)*s3*(qd(1) + qd(2))) - 0.00163355*c4*(c3*qd(3)*(qd(1) + qd(2)) + s3*(qdd(1) + qdd(2))) - c4*(3.29301e-6*c4*(c3*(qdd(1) + qdd(2)) - qd(3)*s3*(qd(1) + qd(2))) - 295*c5*m7*(80*c6*(-c5*(-qdd(3) + qdd(4)) - qd(5)*(c5*(-c3*s4*(qd(1) + qd(2)) + c4*s3*(qd(1) + qd(2))) - s5*(-qd(3) + qd(4))) - s5*(c4*(c3*qd(3)*(qd(1) + qd(2)) + s3*(qdd(1) + qdd(2))) + qd(4)*(-c3*c4*(qd(1) + qd(2)) - s3*s4*(qd(1) + qd(2))) - s4*(c3*(qdd(1) + qdd(2)) - qd(3)*s3*(qd(1) + qd(2))))) + c6*(80*c5*(-qdd(3) + qdd(4)) + c5*(c4*(-295*c3*(qdd(1) + qdd(2)) + c3*(c2*(-g*s1 - 270*qd(1)^2) + s2*(-c1*g + 270*qdd(1)) - (qd(1) + qd(2))*(90*qd(1) + 90*qd(2)))) - s4*(295*s3*(qdd(1) + qdd(2)) - s3*(c2*(-g*s1 - 270*qd(1)^2) + s2*(-c1*g + 270*qdd(1)) - (qd(1) + qd(2))*(90*qd(1) + 90*qd(2))))) + 80*qd(5)*(c5*(-c3*s4*(qd(1) + qd(2)) + c4*s3*(qd(1) + qd(2))) - s5*(-qd(3) + qd(4))) + 80*s5*(c4*(c3*qd(3)*(qd(1) + qd(2)) + s3*(qdd(1) + qdd(2))) + qd(4)*(-c3*c4*(qd(1) + qd(2)) - s3*s4*(qd(1) + qd(2))) - s4*(c3*(qdd(1) + qdd(2)) - qd(3)*s3*(qd(1) + qd(2)))) - s5*(-c2*(-c1*g + 270*qdd(1)) - 295*c3^2*(qd(1) + qd(2)) ^2 - 90*qdd(1) - 90*qdd(2) + s2*(-g*s1 - 270*qd(1)^2) - 295*s3^2*(qd(1) + qd(2)) ^2) - (80*c5*(-c3*s4*(qd(1) + qd(2)) + c4*s3*(qd(1) + qd(2))) - 80*s5*(-qd(3) + qd(4)))*(-c3*c4*(qd(1) + qd(2)) + qd(5) - s3*s4*(qd(1) + qd(2)))) + 80*qd(6)*(c6*(c5*(-c3*s4*(qd(1) + qd(2)) + c4*s3*(qd(1) + qd(2))) - s5*(-qd(3) + qd(4))) - s6*(-c5*(-qd(3) + qd(4)) - s5*(-c3*s4*(qd(1) + qd(2)) + c4*s3*(qd(1) + qd(2))))) + 80*s6*(c5*(c4*(c3*qd(3)*(qd(1) + qd(2)) + s3*(qdd(1) + qdd(2))) + qd(4)*(-c3*c4*(qd(1) + qd(2)) - s3*s4*(qd(1) + qd(2))) - s4*(c3*(qdd(1) + qdd(2)) - qd(3)*s3*(qd(1) + qd(2)))) + qd(5)*(-c5*(-qd(3) + qd(4)) - s5*(-c3*s4*(qd(1) + qd(2)) + c4*s3*(qd(1) + qd(2)))) - s5*(-qdd(3) + qdd(4))) - s6*(80*c5*(c4*(c3*qd(3)*(qd(1) + qd(2)) + s3*(qdd(1) + qdd(2))) + qd(4)*(-c3*c4*(qd(1) + qd(2)) - s3*s4*(qd(1) + qd(2))) - s4*(c3*(qdd(1) + qdd(2)) - qd(3)*s3*(qd(1) + qd(2)))) - c5*(-c2*(-c1*g + 270*qdd(1)) - 295*c3^2*(qd(1) + qd(2)) ^2- 90*qdd(1) - 90*qdd(2) + s2*(-g*s1 - 270*qd(1)^2) - 295*s3^2*(qd(1) + qd(2)) ^2) + 80*qd(5)*(-c5*(-qd(3) + qd(4)) - s5*(-c3*s4*(qd(1) + qd(2)) + c4*s3*(qd(1) + qd(2)))) - 80*s5*(-qdd(3) + qdd(4)) - s5*(c4*(-295*c3*(qdd(1) + qdd(2)) + c3*(c2*(-g*s1 - 270*qd(1)^2) + s2*(-c1*g + 270*qdd(1)) - (qd(1) + qd(2))*(90*qd(1) + 90*qd(2)))) - s4*(295*s3*(qdd(1) + qdd(2)) - s3*(c2*(-g*s1 - 270*qd(1)^2) + s2*(-c1*g + 270*qdd(1)) - (qd(1) + qd(2))*(90*qd(1) + 90*qd(2))))) + (80*c5*(-qd(3) + qd(4)) + 80*s5*(-c3*s4*(qd(1) + qd(2)) + c4*s3*(qd(1) + qd(2))))*(-c3*c4*(qd(1) + qd(2)) + qd(5) - s3*s4*(qd(1) + qd(2)))) - (80*c6*(c5*(-c3*s4*(qd(1) + qd(2)) + c4*s3*(qd(1) + qd(2))) - s5*(-qd(3) + qd(4))) - 80*s6*(-c5*(-qd(3) + qd(4)) - s5*(-c3*s4*(qd(1) + qd(2)) + c4*s3*(qd(1) + qd(2)))))*(c3*c4*(qd(1) + qd(2)) - qd(5) + qd(6) + s3*s4*(qd(1) + qd(2)))) - 0.00355535*c5*(-qdd(3) + qdd(4)) - 0.000409305*c5*(c4*(c3*qd(3)*(qd(1) + qd(2)) + s3*(qdd(1) + qdd(2))) + qd(4)*(-c3*c4*(qd(1) + qd(2)) - s3*s4*(qd(1) + qd(2))) - s4*(c3*(qdd(1) + qdd(2)) - qd(3)*s3*(qd(1) + qd(2)))) - 295*m6*(c5*(c4*(-295*c3*(qdd(1) + qdd(2)) + c3*(c2*(-g*s1 - 270*qd(1)^2) + s2*(-c1*g + 270*qdd(1)) - (qd(1) + qd(2))*(90*qd(1) + 90*qd(2)))) - s4*(295*s3*(qdd(1) + qdd(2)) - s3*(c2*(-g*s1 - 270*qd(1)^2) + s2*(-c1*g + 270*qdd(1)) - (qd(1) + qd(2))*(90*qd(1) + 90*qd(2))))) - s5*(-c2*(-c1*g + 270*qdd(1)) - 295*c3^2*(qd(1) + qd(2)) ^2 - 90*qdd(1) - 90*qdd(2) + s2*(-g*s1 - 270*qd(1)^2) - 295*s3^2*(qd(1) + qd(2)) ^2)) + 295*m7*s5*(80*c6*(c5*(c4*(c3*qd(3)*(qd(1) + qd(2)) + s3*(qdd(1) + qdd(2))) + qd(4)*(-c3*c4*(qd(1) + qd(2)) - s3*s4*(qd(1) + qd(2))) - s4*(c3*(qdd(1) + qdd(2)) - qd(3)*s3*(qd(1) + qd(2)))) + qd(5)*(-c5*(-qd(3) + qd(4)) - s5*(-c3*s4*(qd(1) + qd(2)) + c4*s3*(qd(1) + qd(2)))) - s5*(-qdd(3) + qdd(4))) - c6*(80*c5*(c4*(c3*qd(3)*(qd(1) + qd(2)) + s3*(qdd(1) + qdd(2))) + qd(4)*(-c3*c4*(qd(1) + qd(2)) - s3*s4*(qd(1) + qd(2))) - s4*(c3*(qdd(1) + qdd(2)) - qd(3)*s3*(qd(1) + qd(2)))) - c5*(-c2*(-c1*g + 270*qdd(1)) - 295*c3^2*(qd(1) + qd(2)) ^2 - 90*qdd(1) - 90*qdd(2) + s2*(-g*s1 - 270*qd(1)^2) - 295*s3^2*(qd(1) + qd(2)) ^2) + 80*qd(5)*(-c5*(-qd(3) + qd(4)) - s5*(-c3*s4*(qd(1) + qd(2)) + c4*s3*(qd(1) + qd(2)))) - 80*s5*(-qdd(3) + qdd(4)) - s5*(c4*(-295*c3*(qdd(1) + qdd(2)) + c3*(c2*(-g*s1 - 270*qd(1)^2) + s2*(-c1*g + 270*qdd(1)) - (qd(1) + qd(2))*(90*qd(1) + 90*qd(2)))) - s4*(295*s3*(qdd(1) + qdd(2)) - s3*(c2*(-g*s1 - 270*qd(1)^2) + s2*(-c1*g + 270*qdd(1)) - (qd(1) + qd(2))*(90*qd(1) + 90*qd(2))))) + (80*c5*(-qd(3) + qd(4)) + 80*s5*(-c3*s4*(qd(1) + qd(2)) + c4*s3*(qd(1) + qd(2))))*(-c3*c4*(qd(1) + qd(2)) + qd(5) - s3*s4*(qd(1) + qd(2)))) + 80*qd(6)*(-c6*(-c5*(-qd(3) + qd(4)) - s5*(-c3*s4*(qd(1) + qd(2)) + c4*s3*(qd(1) + qd(2)))) - s6*(c5*(-c3*s4*(qd(1) + qd(2)) + c4*s3*(qd(1) + qd(2))) - s5*(-qd(3) + qd(4)))) - 80*s6*(-c5*(-qdd(3) + qdd(4)) - qd(5)*(c5*(-c3*s4*(qd(1) + qd(2)) + c4*s3*(qd(1) + qd(2))) - s5*(-qd(3) + qd(4))) - s5*(c4*(c3*qd(3)*(qd(1) + qd(2)) + s3*(qdd(1) + qdd(2))) + qd(4)*(-c3*c4*(qd(1) + qd(2)) - s3*s4*(qd(1) + qd(2))) - s4*(c3*(qdd(1) + qdd(2)) - qd(3)*s3*(qd(1) + qd(2))))) - s6*(80*c5*(-qdd(3) + qdd(4)) + c5*(c4*(-295*c3*(qdd(1) + qdd(2)) + c3*(c2*(-g*s1 - 270*qd(1)^2) + s2*(-c1*g + 270*qdd(1)) - (qd(1) + qd(2))*(90*qd(1) + 90*qd(2)))) - s4*(295*s3*(qdd(1) + qdd(2)) - s3*(c2*(-g*s1 - 270*qd(1)^2) + s2*(-c1*g + 270*qdd(1)) - (qd(1) + qd(2))*(90*qd(1) + 90*qd(2))))) + 80*qd(5)*(c5*(-c3*s4*(qd(1) + qd(2)) + c4*s3*(qd(1) + qd(2))) - s5*(-qd(3) + qd(4))) + 80*s5*(c4*(c3*qd(3)*(qd(1) + qd(2)) + s3*(qdd(1) + qdd(2))) + qd(4)*(-c3*c4*(qd(1) + qd(2)) - s3*s4*(qd(1) + qd(2))) - s4*(c3*(qdd(1) + qdd(2)) - qd(3)*s3*(qd(1) + qd(2)))) - s5*(-c2*(-c1*g + 270*qdd(1)) - 295*c3^2*(qd(1) + qd(2)) ^2 - 90*qdd(1) - 90*qdd(2) + s2*(-g*s1 - 270*qd(1)^2) - 295*s3^2*(qd(1) + qd(2)) ^2) - (80*c5*(-c3*s4*(qd(1) + qd(2)) + c4*s3*(qd(1) + qd(2))) - 80*s5*(-qd(3) + qd(4)))*(-c3*c4*(qd(1) + qd(2)) + qd(5) - s3*s4*(qd(1) + qd(2)))) + (80*c6*(-c5*(-qd(3) + qd(4)) - s5*(-c3*s4*(qd(1) + qd(2)) + c4*s3*(qd(1) + qd(2)))) + 80*s6*(c5*(-c3*s4*(qd(1) + qd(2)) + c4*s3*(qd(1) + qd(2))) - s5*(-qd(3) + qd(4))))*(c3*c4*(qd(1) + qd(2)) - qd(5) + qd(6) + s3*s4*(qd(1) + qd(2)))) + 3.29301e-6*qd(4)*(-c3*s4*(qd(1) + qd(2)) + c4*s3*(qd(1) + qd(2))) - 0.000409305*qd(5)*(-c5*(-qd(3) + qd(4)) - s5*(-c3*s4*(qd(1) + qd(2)) + c4*s3*(qd(1) + qd(2)))) - 0.00355535*qd(5)*(c5*(-c3*s4*(qd(1) + qd(2)) + c4*s3*(qd(1) + qd(2))) - s5*(-qd(3) + qd(4))) - 3.29301e-6*qdd(5) + 3.29301e-6*qdd(6) + 3.29301e-6*s4*(c3*qd(3)*(qd(1) + qd(2)) + s3*(qdd(1) + qdd(2))) + 0.000409305*s5*(-qdd(3) + qdd(4)) - 0.00355535*s5*(c4*(c3*qd(3)*(qd(1) + qd(2)) + s3*(qdd(1) + qdd(2))) + qd(4)*(-c3*c4*(qd(1) + qd(2)) - s3*s4*(qd(1) + qd(2))) - s4*(c3*(qdd(1) + qdd(2)) - qd(3)*s3*(qd(1) + qd(2)))) - (c5*(-c3*s4*(qd(1) + qd(2)) + c4*s3*(qd(1) + qd(2))) - s5*(-qd(3) + qd(4)))*(-0.00358942*c3*c4*(qd(1) + qd(2)) + 0.00358942*qd(5) - 0.00358942*s3*s4*(qd(1) + qd(2))) - (-c6*(-c5*(-qd(3) + qd(4)) - s5*(-c3*s4*(qd(1) + qd(2)) + c4*s3*(qd(1) + qd(2)))) - s6*(c5*(-c3*s4*(qd(1) + qd(2)) + c4*s3*(qd(1) + qd(2))) - s5*(-qd(3) + qd(4))))*(6.20477e-6*c6*(c5*(-c3*s4*(qd(1) + qd(2)) + c4*s3*(qd(1) + qd(2))) - s5*(-qd(3) + qd(4))) - 6.20477e-6*s6*(-c5*(-qd(3) + qd(4)) - s5*(-c3*s4*(qd(1) + qd(2)) + c4*s3*(qd(1) + qd(2))))) + (-3.01352e-6*c6*(-c5*(-qd(3) + qd(4)) - s5*(-c3*s4*(qd(1) + qd(2)) + c4*s3*(qd(1) + qd(2)))) - 3.01352e-6*s6*(c5*(-c3*s4*(qd(1) + qd(2)) + c4*s3*(qd(1) + qd(2))) - s5*(-qd(3) + qd(4))))*(c6*(c5*(-c3*s4*(qd(1) + qd(2)) + c4*s3*(qd(1) + qd(2))) - s5*(-qd(3) + qd(4))) - s6*(-c5*(-qd(3) + qd(4)) - s5*(-c3*s4*(qd(1) + qd(2)) + c4*s3*(qd(1) + qd(2))))) + (-c3*c4*(qd(1) + qd(2)) + qd(5) - s3*s4*(qd(1) + qd(2)))*(0.000409305*c5*(-qd(3) + qd(4)) + 0.00151607*c5*(-c3*s4*(qd(1) + qd(2)) + c4*s3*(qd(1) + qd(2))) - 0.00151607*s5*(-qd(3) + qd(4)) + 0.000409305*s5*(-c3*s4*(qd(1) + qd(2)) + c4*s3*(qd(1) + qd(2))))) - 90*c5*m7*(80*c6*(c5*(c4*(c3*qd(3)*(qd(1) + qd(2)) + s3*(qdd(1) + qdd(2))) + qd(4)*(-c3*c4*(qd(1) + qd(2)) - s3*s4*(qd(1) + qd(2))) - s4*(c3*(qdd(1) + qdd(2)) - qd(3)*s3*(qd(1) + qd(2)))) + qd(5)*(-c5*(-qd(3) + qd(4)) - s5*(-c3*s4*(qd(1) + qd(2)) + c4*s3*(qd(1) + qd(2)))) - s5*(-qdd(3) + qdd(4))) - c6*(80*c5*(c4*(c3*qd(3)*(qd(1) + qd(2)) + s3*(qdd(1) + qdd(2))) + qd(4)*(-c3*c4*(qd(1) + qd(2)) - s3*s4*(qd(1) + qd(2))) - s4*(c3*(qdd(1) + qdd(2)) - qd(3)*s3*(qd(1) + qd(2)))) - c5*(-c2*(-c1*g + 270*qdd(1)) - 295*c3^2*(qd(1) + qd(2)) ^2 - 90*qdd(1) - 90*qdd(2) + s2*(-g*s1 - 270*qd(1)^2) - 295*s3^2*(qd(1) + qd(2))^2) + 80*qd(5)*(-c5*(-qd(3) + qd(4)) - s5*(-c3*s4*(qd(1) + qd(2)) + c4*s3*(qd(1) + qd(2)))) - 80*s5*(-qdd(3) + qdd(4)) - s5*(c4*(-295*c3*(qdd(1) + qdd(2)) + c3*(c2*(-g*s1 - 270*qd(1)^2) + s2*(-c1*g + 270*qdd(1)) - (qd(1) + qd(2))*(90*qd(1) + 90*qd(2)))) - s4*(295*s3*(qdd(1) + qdd(2)) - s3*(c2*(-g*s1 - 270*qd(1)^2) + s2*(-c1*g + 270*qdd(1)) - (qd(1) + qd(2))*(90*qd(1) + 90*qd(2))))) + (80*c5*(-qd(3) + qd(4)) + 80*s5*(-c3*s4*(qd(1) + qd(2)) + c4*s3*(qd(1) + qd(2))))*(-c3*c4*(qd(1) + qd(2)) + qd(5) - s3*s4*(qd(1) + qd(2)))) + 80*qd(6)*(-c6*(-c5*(-qd(3) + qd(4)) - s5*(-c3*s4*(qd(1) + qd(2)) + c4*s3*(qd(1) + qd(2)))) - s6*(c5*(-c3*s4*(qd(1) + qd(2)) + c4*s3*(qd(1) + qd(2))) - s5*(-qd(3) + qd(4)))) - 80*s6*(-c5*(-qdd(3) + qdd(4)) - qd(5)*(c5*(-c3*s4*(qd(1) + qd(2)) + c4*s3*(qd(1) + qd(2))) - s5*(-qd(3) + qd(4))) - s5*(c4*(c3*qd(3)*(qd(1) + qd(2)) + s3*(qdd(1) + qdd(2))) + qd(4)*(-c3*c4*(qd(1) + qd(2)) - s3*s4*(qd(1) + qd(2))) - s4*(c3*(qdd(1) + qdd(2)) - qd(3)*s3*(qd(1) + qd(2))))) - s6*(80*c5*(-qdd(3) + qdd(4)) + c5*(c4*(-295*c3*(qdd(1) + qdd(2)) + c3*(c2*(-g*s1 - 270*qd(1)^2) + s2*(-c1*g + 270*qdd(1)) - (qd(1) + qd(2))*(90*qd(1) + 90*qd(2)))) - s4*(295*s3*(qdd(1) + qdd(2)) - s3*(c2*(-g*s1 - 270*qd(1)^2) + s2*(-c1*g + 270*qdd(1)) - (qd(1) + qd(2))*(90*qd(1) + 90*qd(2))))) + 80*qd(5)*(c5*(-c3*s4*(qd(1) + qd(2)) + c4*s3*(qd(1) + qd(2))) - s5*(-qd(3) + qd(4))) + 80*s5*(c4*(c3*qd(3)*(qd(1) + qd(2)) + s3*(qdd(1) + qdd(2))) + qd(4)*(-c3*c4*(qd(1) + qd(2)) - s3*s4*(qd(1) + qd(2))) - s4*(c3*(qdd(1) + qdd(2)) - qd(3)*s3*(qd(1) + qd(2)))) - s5*(-c2*(-c1*g + 270*qdd(1)) - 295*c3^2*(qd(1) + qd(2)) ^2 - 90*qdd(1) - 90*qdd(2) + s2*(-g*s1 - 270*qd(1)^2) - 295*s3^2*(qd(1) + qd(2)) ^2) - (80*c5*(-c3*s4*(qd(1) + qd(2)) + c4*s3*(qd(1) + qd(2))) - 80*s5*(-qd(3) + qd(4)))*(-c3*c4*(qd(1) + qd(2)) + qd(5) - s3*s4*(qd(1) + qd(2)))) + (80*c6*(-c5*(-qd(3) + qd(4)) - s5*(-c3*s4*(qd(1) + qd(2)) + c4*s3*(qd(1) + qd(2)))) + 80*s6*(c5*(-c3*s4*(qd(1) + qd(2)) + c4*s3*(qd(1) + qd(2))) - s5*(-qd(3) + qd(4))))*(c3*c4*(qd(1) + qd(2)) - qd(5) + qd(6) + s3*s4*(qd(1) + qd(2)))) - 90*m5*(-c2*(-c1*g + 270*qdd(1)) - 295*c3^2*(qd(1) + qd(2)) ^2 - 90*qdd(1) - 90*qdd(2) + s2*(-g*s1 - 270*qd(1)^2) - 295*s3^2*(qd(1) + qd(2)) ^2 - (-c3*c4*(qd(1) + qd(2)) - s3*s4*(qd(1) + qd(2)))*(295*c3*c4*(qd(1) + qd(2)) + 295*s3*s4*(qd(1) + qd(2))) + (-295*c3*s4*(qd(1) + qd(2)) + 295*c4*s3*(qd(1) + qd(2)))*(-c3*s4*(qd(1) + qd(2)) + c4*s3*(qd(1) + qd(2)))) + 90*m6*(-c4*(295*s3*(qdd(1) + qdd(2)) - s3*(c2*(-g*s1 - 270*qd(1)^2) + s2*(-c1*g + 270*qdd(1)) - (qd(1) + qd(2))*(90*qd(1) + 90*qd(2)))) - s4*(-295*c3*(qdd(1) + qdd(2)) + c3*(c2*(-g*s1 - 270*qd(1)^2) + s2*(-c1*g + 270*qdd(1)) - (qd(1) + qd(2))*(90*qd(1) + 90*qd(2))))) - 90*m7*s5*(80*c6*(-c5*(-qdd(3) + qdd(4)) - qd(5)*(c5*(-c3*s4*(qd(1) + qd(2)) + c4*s3*(qd(1) + qd(2))) - s5*(-qd(3) + qd(4))) - s5*(c4*(c3*qd(3)*(qd(1) + qd(2)) + s3*(qdd(1) + qdd(2))) + qd(4)*(-c3*c4*(qd(1) + qd(2)) - s3*s4*(qd(1) + qd(2))) - s4*(c3*(qdd(1) + qdd(2)) - qd(3)*s3*(qd(1) + qd(2))))) + c6*(80*c5*(-qdd(3) + qdd(4)) + c5*(c4*(-295*c3*(qdd(1) + qdd(2)) + c3*(c2*(-g*s1 - 270*qd(1)^2) + s2*(-c1*g + 270*qdd(1)) - (qd(1) + qd(2))*(90*qd(1) + 90*qd(2)))) - s4*(295*s3*(qdd(1) + qdd(2)) - s3*(c2*(-g*s1 - 270*qd(1)^2) + s2*(-c1*g + 270*qdd(1)) - (qd(1) + qd(2))*(90*qd(1) + 90*qd(2))))) + 80*qd(5)*(c5*(-c3*s4*(qd(1) + qd(2)) + c4*s3*(qd(1) + qd(2))) - s5*(-qd(3) + qd(4))) + 80*s5*(c4*(c3*qd(3)*(qd(1) + qd(2)) + s3*(qdd(1) + qdd(2))) + qd(4)*(-c3*c4*(qd(1) + qd(2)) - s3*s4*(qd(1) + qd(2))) - s4*(c3*(qdd(1) + qdd(2)) - qd(3)*s3*(qd(1) + qd(2)))) - s5*(-c2*(-c1*g + 270*qdd(1)) - 295*c3^2*(qd(1) + qd(2))^2 - 90*qdd(1) - 90*qdd(2) + s2*(-g*s1 - 270*qd(1)^2) - 295*s3^2*(qd(1) + qd(2)) ^2) - (80*c5*(-c3*s4*(qd(1) + qd(2)) + c4*s3*(qd(1) + qd(2))) - 80*s5*(-qd(3) + qd(4)))*(-c3*c4*(qd(1) + qd(2)) + qd(5) - s3*s4*(qd(1) + qd(2)))) + 80*qd(6)*(c6*(c5*(-c3*s4*(qd(1) + qd(2)) + c4*s3*(qd(1) + qd(2))) - s5*(-qd(3) + qd(4))) - s6*(-c5*(-qd(3) + qd(4)) - s5*(-c3*s4*(qd(1) + qd(2)) + c4*s3*(qd(1) + qd(2))))) + 80*s6*(c5*(c4*(c3*qd(3)*(qd(1) + qd(2)) + s3*(qdd(1) + qdd(2))) + qd(4)*(-c3*c4*(qd(1) + qd(2)) - s3*s4*(qd(1) + qd(2))) - s4*(c3*(qdd(1) + qdd(2)) - qd(3)*s3*(qd(1) + qd(2)))) + qd(5)*(-c5*(-qd(3) + qd(4)) - s5*(-c3*s4*(qd(1) + qd(2)) + c4*s3*(qd(1) + qd(2)))) - s5*(-qdd(3) + qdd(4))) - s6*(80*c5*(c4*(c3*qd(3)*(qd(1) + qd(2)) + s3*(qdd(1) + qdd(2))) + qd(4)*(-c3*c4*(qd(1) + qd(2)) - s3*s4*(qd(1) + qd(2))) - s4*(c3*(qdd(1) + qdd(2)) - qd(3)*s3*(qd(1) + qd(2)))) - c5*(-c2*(-c1*g + 270*qdd(1)) - 295*c3^2*(qd(1) + qd(2)) ^2 - 90*qdd(1) - 90*qdd(2) + s2*(-g*s1 - 270*qd(1)^2) - 295*s3^2*(qd(1) + qd(2)) ^2) + 80*qd(5)*(-c5*(-qd(3) + qd(4)) - s5*(-c3*s4*(qd(1) + qd(2)) + c4*s3*(qd(1) + qd(2)))) - 80*s5*(-qdd(3) + qdd(4)) - s5*(c4*(-295*c3*(qdd(1) + qdd(2)) + c3*(c2*(-g*s1 - 270*qd(1)^2) + s2*(-c1*g + 270*qdd(1)) - (qd(1) + qd(2))*(90*qd(1) + 90*qd(2)))) - s4*(295*s3*(qdd(1) + qdd(2)) - s3*(c2*(-g*s1 - 270*qd(1)^2) + s2*(-c1*g + 270*qdd(1)) - (qd(1) + qd(2))*(90*qd(1) + 90*qd(2))))) + (80*c5*(-qd(3) + qd(4)) + 80*s5*(-c3*s4*(qd(1) + qd(2)) + c4*s3*(qd(1) + qd(2))))*(-c3*c4*(qd(1) + qd(2)) + qd(5) - s3*s4*(qd(1) + qd(2)))) - (80*c6*(c5*(-c3*s4*(qd(1) + qd(2)) + c4*s3*(qd(1) + qd(2))) - s5*(-qd(3) + qd(4))) - 80*s6*(-c5*(-qd(3) + qd(4)) - s5*(-c3*s4*(qd(1) + qd(2)) + c4*s3*(qd(1) + qd(2)))))*(c3*c4*(qd(1) + qd(2)) - qd(5) + qd(6) + s3*s4*(qd(1) + qd(2)))) - 0.00163355*qd(4)*(-c3*c4*(qd(1) + qd(2)) - s3*s4*(qd(1) + qd(2))) - 0.020170031*qd(4)*(-c3*s4*(qd(1) + qd(2)) + c4*s3*(qd(1) + qd(2))) + 2.69102e-6*qdd(3) - 2.69102e-6*qdd(4) + 0.00163355*s4*(c3*(qdd(1) + qdd(2)) - qd(3)*s3*(qd(1) + qd(2))) - 0.020170031*s4*(c3*qd(3)*(qd(1) + qd(2)) + s3*(qdd(1) + qdd(2))) - s4*(0.000409305*c5*(-qdd(3) + qdd(4)) + 0.00151607*c5*(c4*(c3*qd(3)*(qd(1) + qd(2)) + s3*(qdd(1) + qdd(2))) + qd(4)*(-c3*c4*(qd(1) + qd(2)) - s3*s4*(qd(1) + qd(2))) - s4*(c3*(qdd(1) + qdd(2)) - qd(3)*s3*(qd(1) + qd(2)))) + c5*(6.20477e-6*c6*(c5*(c4*(c3*qd(3)*(qd(1) + qd(2)) + s3*(qdd(1) + qdd(2))) + qd(4)*(-c3*c4*(qd(1) + qd(2)) - s3*s4*(qd(1) + qd(2))) - s4*(c3*(qdd(1) + qdd(2)) - qd(3)*s3*(qd(1) + qd(2)))) + qd(5)*(-c5*(-qd(3) + qd(4)) - s5*(-c3*s4*(qd(1) + qd(2)) + c4*s3*(qd(1) + qd(2)))) - s5*(-qdd(3) + qdd(4))) + 6.20477e-6*qd(6)*(-c6*(-c5*(-qd(3) + qd(4)) - s5*(-c3*s4*(qd(1) + qd(2)) + c4*s3*(qd(1) + qd(2)))) - s6*(c5*(-c3*s4*(qd(1) + qd(2)) + c4*s3*(qd(1) + qd(2))) - s5*(-qd(3) + qd(4)))) - 6.20477e-6*s6*(-c5*(-qdd(3) + qdd(4)) - qd(5)*(c5*(-c3*s4*(qd(1) + qd(2)) + c4*s3*(qd(1) + qd(2))) - s5*(-qd(3) + qd(4))) - s5*(c4*(c3*qd(3)*(qd(1) + qd(2)) + s3*(qdd(1) + qdd(2))) + qd(4)*(-c3*c4*(qd(1) + qd(2)) - s3*s4*(qd(1) + qd(2))) - s4*(c3*(qdd(1) + qdd(2)) - qd(3)*s3*(qd(1) + qd(2))))) + (-c6*(-c5*(-qd(3) + qd(4)) - s5*(-c3*s4*(qd(1) + qd(2)) + c4*s3*(qd(1) + qd(2)))) - s6*(c5*(-c3*s4*(qd(1) + qd(2)) + c4*s3*(qd(1) + qd(2))) - s5*(-qd(3) + qd(4))))*(3.29301e-6*c3*c4*(qd(1) + qd(2)) - 3.29301e-6*qd(5) + 3.29301e-6*qd(6) + 3.29301e-6*s3*s4*(qd(1) + qd(2))) - (-3.01352e-6*c6*(-c5*(-qd(3) + qd(4)) - s5*(-c3*s4*(qd(1) + qd(2)) + c4*s3*(qd(1) + qd(2)))) - 3.01352e-6*s6*(c5*(-c3*s4*(qd(1) + qd(2)) + c4*s3*(qd(1) + qd(2))) - s5*(-qd(3) + qd(4))))*(c3*c4*(qd(1) + qd(2)) - qd(5) + qd(6) + s3*s4*(qd(1) + qd(2)))) + 295*m6*(-c5*(-c2*(-c1*g + 270*qdd(1)) - 295*c3^2*(qd(1) + qd(2)) ^2 - 90*qdd(1) - 90*qdd(2) + s2*(-g*s1 - 270*qd(1)^2) - 295*s3^2*(qd(1) + qd(2))^2) - s5*(c4*(-295*c3*(qdd(1) + qdd(2)) + c3*(c2*(-g*s1 - 270*qd(1)^2) + s2*(-c1*g + 270*qdd(1)) - (qd(1) + qd(2))*(90*qd(1) + 90*qd(2)))) - s4*(295*s3*(qdd(1) + qdd(2)) - s3*(c2*(-g*s1 - 270*qd(1)^2) + s2*(-c1*g + 270*qdd(1)) - (qd(1) + qd(2))*(90*qd(1) + 90*qd(2)))))) + 295*m7*(c4*(295*s3*(qdd(1) + qdd(2)) - s3*(c2*(-g*s1 - 270*qd(1)^2) + s2*(-c1*g + 270*qdd(1)) - (qd(1) + qd(2))*(90*qd(1) + 90*qd(2)))) + s4*(-295*c3*(qdd(1) + qdd(2)) + c3*(c2*(-g*s1 - 270*qd(1)^2) + s2*(-c1*g + 270*qdd(1)) - (qd(1) + qd(2))*(90*qd(1) + 90*qd(2)))) + (-c5*(-qd(3) + qd(4)) - s5*(-c3*s4*(qd(1) + qd(2)) + c4*s3*(qd(1) + qd(2))))*(80*c5*(-qd(3) + qd(4)) + 80*s5*(-c3*s4*(qd(1) + qd(2)) + c4*s3*(qd(1) + qd(2)))) - (c5*(-c3*s4*(qd(1) + qd(2)) + c4*s3*(qd(1) + qd(2))) - s5*(-qd(3) + qd(4)))*(80*c5*(-c3*s4*(qd(1) + qd(2)) + c4*s3*(qd(1) + qd(2))) - 80*s5*(-qd(3) + qd(4))) - (-c6*(-c5*(-qd(3) + qd(4)) - s5*(-c3*s4*(qd(1) + qd(2)) + c4*s3*(qd(1) + qd(2)))) - s6*(c5*(-c3*s4*(qd(1) + qd(2)) + c4*s3*(qd(1) + qd(2))) - s5*(-qd(3) + qd(4))))*(80*c6*(-c5*(-qd(3) + qd(4)) - s5*(-c3*s4*(qd(1) + qd(2)) + c4*s3*(qd(1) + qd(2)))) + 80*s6*(c5*(-c3*s4*(qd(1) + qd(2)) + c4*s3*(qd(1) + qd(2))) - s5*(-qd(3) + qd(4)))) + (c6*(c5*(-c3*s4*(qd(1) + qd(2)) + c4*s3*(qd(1) + qd(2))) - s5*(-qd(3) + qd(4))) - s6*(-c5*(-qd(3) + qd(4)) - s5*(-c3*s4*(qd(1) + qd(2)) + c4*s3*(qd(1) + qd(2)))))*(80*c6*(c5*(-c3*s4*(qd(1) + qd(2)) + c4*s3*(qd(1) + qd(2))) - s5*(-qd(3) + qd(4))) - 80*s6*(-c5*(-qd(3) + qd(4)) - s5*(-c3*s4*(qd(1) + qd(2)) + c4*s3*(qd(1) + qd(2)))))) + 0.00151607*qd(5)*(-c5*(-qd(3) + qd(4)) - s5*(-c3*s4*(qd(1) + qd(2)) + c4*s3*(qd(1) + qd(2)))) + 0.000409305*qd(5)*(c5*(-c3*s4*(qd(1) + qd(2)) + c4*s3*(qd(1) + qd(2))) - s5*(-qd(3) + qd(4))) - 0.00151607*s5*(-qdd(3) + qdd(4)) + 0.000409305*s5*(c4*(c3*qd(3)*(qd(1) + qd(2)) + s3*(qdd(1) + qdd(2))) + qd(4)*(-c3*c4*(qd(1) + qd(2)) - s3*s4*(qd(1) + qd(2))) - s4*(c3*(qdd(1) + qdd(2)) - qd(3)*s3*(qd(1) + qd(2)))) - s5*(-3.01352e-6*c6*(-c5*(-qdd(3) + qdd(4)) - qd(5)*(c5*(-c3*s4*(qd(1) + qd(2)) + c4*s3*(qd(1) + qd(2))) - s5*(-qd(3) + qd(4))) - s5*(c4*(c3*qd(3)*(qd(1) + qd(2)) + s3*(qdd(1) + qdd(2))) + qd(4)*(-c3*c4*(qd(1) + qd(2)) - s3*s4*(qd(1) + qd(2))) - s4*(c3*(qdd(1) + qdd(2)) - qd(3)*s3*(qd(1) + qd(2))))) - 3.01352e-6*qd(6)*(c6*(c5*(-c3*s4*(qd(1) + qd(2)) + c4*s3*(qd(1) + qd(2))) - s5*(-qd(3) + qd(4))) - s6*(-c5*(-qd(3) + qd(4)) - s5*(-c3*s4*(qd(1) + qd(2)) + c4*s3*(qd(1) + qd(2))))) - 3.01352e-6*s6*(c5*(c4*(c3*qd(3)*(qd(1) + qd(2)) + s3*(qdd(1) + qdd(2))) + qd(4)*(-c3*c4*(qd(1) + qd(2)) - s3*s4*(qd(1) + qd(2))) - s4*(c3*(qdd(1) + qdd(2)) - qd(3)*s3*(qd(1) + qd(2)))) + qd(5)*(-c5*(-qd(3) + qd(4)) - s5*(-c3*s4*(qd(1) + qd(2)) + c4*s3*(qd(1) + qd(2)))) - s5*(-qdd(3) + qdd(4))) + (6.20477e-6*c6*(c5*(-c3*s4*(qd(1) + qd(2)) + c4*s3*(qd(1) + qd(2))) - s5*(-qd(3) + qd(4))) - 6.20477e-6*s6*(-c5*(-qd(3) + qd(4)) - s5*(-c3*s4*(qd(1) + qd(2)) + c4*s3*(qd(1) + qd(2)))))*(c3*c4*(qd(1) + qd(2)) - qd(5) + qd(6) + s3*s4*(qd(1) + qd(2))) - (c6*(c5*(-c3*s4*(qd(1) + qd(2)) + c4*s3*(qd(1) + qd(2))) - s5*(-qd(3) + qd(4))) - s6*(-c5*(-qd(3) + qd(4)) - s5*(-c3*s4*(qd(1) + qd(2)) + c4*s3*(qd(1) + qd(2)))))*(3.29301e-6*c3*c4*(qd(1) + qd(2)) - 3.29301e-6*qd(5) + 3.29301e-6*qd(6) + 3.29301e-6*s3*s4*(qd(1) + qd(2)))) + (-c5*(-qd(3) + qd(4)) - s5*(-c3*s4*(qd(1) + qd(2)) + c4*s3*(qd(1) + qd(2))))*(-0.00358942*c3*c4*(qd(1) + qd(2)) + 0.00358942*qd(5) - 0.00358942*s3*s4*(qd(1) + qd(2))) - (-c3*c4*(qd(1) + qd(2)) + qd(5) - s3*s4*(qd(1) + qd(2)))*(-0.00355535*c5*(-qd(3) + qd(4)) - 0.000409305*c5*(-c3*s4*(qd(1) + qd(2)) + c4*s3*(qd(1) + qd(2))) + 0.000409305*s5*(-qd(3) + qd(4)) - 0.00355535*s5*(-c3*s4*(qd(1) + qd(2)) + c4*s3*(qd(1) + qd(2))))) + (-qd(3) + qd(4))*(0.00163355*c3*c4*(qd(1) + qd(2)) - 0.00950111*c3*s4*(qd(1) + qd(2)) + 0.00950111*c4*s3*(qd(1) + qd(2)) + 8.41256e-6*qd(3) - 8.41256e-6*qd(4) + 0.00163355*s3*s4*(qd(1) + qd(2))) - (-c3*s4*(qd(1) + qd(2)) + c4*s3*(qd(1) + qd(2)))*(2.69102e-6*c3*c4*(qd(1) + qd(2)) + 8.41256e-6*c3*s4*(qd(1) + qd(2)) - 8.41256e-6*c4*s3*(qd(1) + qd(2)) - 0.024130024*qd(3) + 0.024130024*qd(4) + 2.69102e-6*s3*s4*(qd(1) + qd(2)))) + 270*c5*m7*(80*c6*(c5*(c4*(c3*qd(3)*(qd(1) + qd(2)) + s3*(qdd(1) + qdd(2))) + qd(4)*(-c3*c4*(qd(1) + qd(2)) - s3*s4*(qd(1) + qd(2))) - s4*(c3*(qdd(1) + qdd(2)) - qd(3)*s3*(qd(1) + qd(2)))) + qd(5)*(-c5*(-qd(3) + qd(4)) - s5*(-c3*s4*(qd(1) + qd(2)) + c4*s3*(qd(1) + qd(2)))) - s5*(-qdd(3) + qdd(4))) - c6*(80*c5*(c4*(c3*qd(3)*(qd(1) + qd(2)) + s3*(qdd(1) + qdd(2))) + qd(4)*(-c3*c4*(qd(1) + qd(2)) - s3*s4*(qd(1) + qd(2))) - s4*(c3*(qdd(1) + qdd(2)) - qd(3)*s3*(qd(1) + qd(2)))) - c5*(-c2*(-c1*g + 270*qdd(1)) - 295*c3^2*(qd(1) + qd(2)^2- 90*qdd(1) - 90*qdd(2) + s2*(-g*s1 - 270*qd(1)^2) - 295*s3^2*(qd(1) + qd(2)) ^2) + 80*qd(5)*(-c5*(-qd(3) + qd(4)) - s5*(-c3*s4*(qd(1) + qd(2)) + c4*s3*(qd(1) + qd(2)))) - 80*s5*(-qdd(3) + qdd(4)) - s5*(c4*(-295*c3*(qdd(1) + qdd(2)) + c3*(c2*(-g*s1 - 270*qd(1)^2) + s2*(-c1*g + 270*qdd(1)) - (qd(1) + qd(2))*(90*qd(1) + 90*qd(2)))) - s4*(295*s3*(qdd(1) + qdd(2)) - s3*(c2*(-g*s1 - 270*qd(1)^2) + s2*(-c1*g + 270*qdd(1)) - (qd(1) + qd(2))*(90*qd(1) + 90*qd(2))))) + (80*c5*(-qd(3) + qd(4)) + 80*s5*(-c3*s4*(qd(1) + qd(2)) + c4*s3*(qd(1) + qd(2))))*(-c3*c4*(qd(1) + qd(2)) + qd(5) - s3*s4*(qd(1) + qd(2)))) + 80*qd(6)*(-c6*(-c5*(-qd(3) + qd(4)) - s5*(-c3*s4*(qd(1) + qd(2)) + c4*s3*(qd(1) + qd(2)))) - s6*(c5*(-c3*s4*(qd(1) + qd(2)) + c4*s3*(qd(1) + qd(2))) - s5*(-qd(3) + qd(4)))) - 80*s6*(-c5*(-qdd(3) + qdd(4)) - qd(5)*(c5*(-c3*s4*(qd(1) + qd(2)) + c4*s3*(qd(1) + qd(2))) - s5*(-qd(3) + qd(4))) - s5*(c4*(c3*qd(3)*(qd(1) + qd(2)) + s3*(qdd(1) + qdd(2))) + qd(4)*(-c3*c4*(qd(1) + qd(2)) - s3*s4*(qd(1) + qd(2))) - s4*(c3*(qdd(1) + qdd(2)) - qd(3)*s3*(qd(1) + qd(2))))) - s6*(80*c5*(-qdd(3) + qdd(4)) + c5*(c4*(-295*c3*(qdd(1) + qdd(2)) + c3*(c2*(-g*s1 - 270*qd(1)^2) + s2*(-c1*g + 270*qdd(1)) - (qd(1) + qd(2))*(90*qd(1) + 90*qd(2)))) - s4*(295*s3*(qdd(1) + qdd(2)) - s3*(c2*(-g*s1 - 270*qd(1)^2) + s2*(-c1*g + 270*qdd(1)) - (qd(1) + qd(2))*(90*qd(1) + 90*qd(2))))) + 80*qd(5)*(c5*(-c3*s4*(qd(1) + qd(2)) + c4*s3*(qd(1) + qd(2))) - s5*(-qd(3) + qd(4))) + 80*s5*(c4*(c3*qd(3)*(qd(1) + qd(2)) + s3*(qdd(1) + qdd(2))) + qd(4)*(-c3*c4*(qd(1) + qd(2)) - s3*s4*(qd(1) + qd(2))) - s4*(c3*(qdd(1) + qdd(2)) - qd(3)*s3*(qd(1) + qd(2)))) - s5*(-c2*(-c1*g + 270*qdd(1)) - 295*c3^2*(qd(1) + qd(2)) ^2- 90*qdd(1) - 90*qdd(2) + s2*(-g*s1 - 270*qd(1)^2) - 295*s3^2*(qd(1) + qd(2)) ^2) - (80*c5*(-c3*s4*(qd(1) + qd(2)) + c4*s3*(qd(1) + qd(2))) - 80*s5*(-qd(3) + qd(4)))*(-c3*c4*(qd(1) + qd(2)) + qd(5) - s3*s4*(qd(1) + qd(2)))) + (80*c6*(-c5*(-qd(3) + qd(4)) - s5*(-c3*s4*(qd(1) + qd(2)) + c4*s3*(qd(1) + qd(2)))) + 80*s6*(c5*(-c3*s4*(qd(1) + qd(2)) + c4*s3*(qd(1) + qd(2))) - s5*(-qd(3) + qd(4))))*(c3*c4*(qd(1) + qd(2)) - qd(5) + qd(6) + s3*s4*(qd(1) + qd(2)))) - 335*m3*(c2*(-g*s1 - 270*qd(1)^2) + s2*(-c1*g + 270*qdd(1)) - (qd(1) + qd(2))*(270*qd(1) + 270*qd(2))) + 75*m3*(c2*(-c1*g + 270*qdd(1)) + 270*qdd(1) + 270*qdd(2) - s2*(-g*s1 - 270*qd(1)^2)) + 270*m4*(90*c3*s3*(qd(1) + qd(2)) ^2 + 90*qdd(3) - s3*(c2*(-g*s1 - 270*qd(1)^2) + s2*(-c1*g + 270*qdd(1)) - (qd(1) + qd(2))*(90*qd(1) + 90*qd(2)))) + 270*m5*(-c2*(-c1*g + 270*qdd(1)) - 295*c3^2*(qd(1) + qd(2)) ^2 - 90*qdd(1) - 90*qdd(2) + s2*(-g*s1 - 270*qd(1)^2) - 295*s3^2*(qd(1) + qd(2)) ^2 - (-c3*c4*(qd(1) + qd(2)) - s3*s4*(qd(1) + qd(2)))*(295*c3*c4*(qd(1) + qd(2)) + 295*s3*s4*(qd(1) + qd(2))) + (-295*c3*s4*(qd(1) + qd(2)) + 295*c4*s3*(qd(1) + qd(2)))*(-c3*s4*(qd(1) + qd(2)) + c4*s3*(qd(1) + qd(2)))) - 270*m6*(-c4*(295*s3*(qdd(1) + qdd(2)) - s3*(c2*(-g*s1 - 270*qd(1)^2) + s2*(-c1*g + 270*qdd(1)) - (qd(1) + qd(2))*(90*qd(1) + 90*qd(2)))) - s4*(-295*c3*(qdd(1) + qdd(2)) + c3*(c2*(-g*s1 - 270*qd(1)^2) + s2*(-c1*g + 270*qdd(1)) - (qd(1) + qd(2))*(90*qd(1) + 90*qd(2))))) + 270*m7*s5*(80*c6*(-c5*(-qdd(3) + qdd(4)) - qd(5)*(c5*(-c3*s4*(qd(1) + qd(2)) + c4*s3*(qd(1) + qd(2))) - s5*(-qd(3) + qd(4))) - s5*(c4*(c3*qd(3)*(qd(1) + qd(2)) + s3*(qdd(1) + qdd(2))) + qd(4)*(-c3*c4*(qd(1) + qd(2)) - s3*s4*(qd(1) + qd(2))) - s4*(c3*(qdd(1) + qdd(2)) - qd(3)*s3*(qd(1) + qd(2))))) + c6*(80*c5*(-qdd(3) + qdd(4)) + c5*(c4*(-295*c3*(qdd(1) + qdd(2)) + c3*(c2*(-g*s1 - 270*qd(1)^2) + s2*(-c1*g + 270*qdd(1)) - (qd(1) + qd(2))*(90*qd(1) + 90*qd(2)))) - s4*(295*s3*(qdd(1) + qdd(2)) - s3*(c2*(-g*s1 - 270*qd(1)^2) + s2*(-c1*g + 270*qdd(1)) - (qd(1) + qd(2))*(90*qd(1) + 90*qd(2))))) + 80*qd(5)*(c5*(-c3*s4*(qd(1) + qd(2)) + c4*s3*(qd(1) + qd(2))) - s5*(-qd(3) + qd(4))) + 80*s5*(c4*(c3*qd(3)*(qd(1) + qd(2)) + s3*(qdd(1) + qdd(2))) + qd(4)*(-c3*c4*(qd(1) + qd(2)) - s3*s4*(qd(1) + qd(2))) - s4*(c3*(qdd(1) + qdd(2)) - qd(3)*s3*(qd(1) + qd(2)))) - s5*(-c2*(-c1*g + 270*qdd(1)) - 295*c3^2*(qd(1) + qd(2)) ^2 - 90*qdd(1) - 90*qdd(2) + s2*(-g*s1 - 270*qd(1)^2) - 295*s3^2*(qd(1) + qd(2)) ^2) - (80*c5*(-c3*s4*(qd(1) + qd(2)) + c4*s3*(qd(1) + qd(2))) - 80*s5*(-qd(3) + qd(4)))*(-c3*c4*(qd(1) + qd(2)) + qd(5) - s3*s4*(qd(1) + qd(2)))) + 80*qd(6)*(c6*(c5*(-c3*s4*(qd(1) + qd(2)) + c4*s3*(qd(1) + qd(2))) - s5*(-qd(3) + qd(4))) - s6*(-c5*(-qd(3) + qd(4)) - s5*(-c3*s4*(qd(1) + qd(2)) + c4*s3*(qd(1) + qd(2))))) + 80*s6*(c5*(c4*(c3*qd(3)*(qd(1) + qd(2)) + s3*(qdd(1) + qdd(2))) + qd(4)*(-c3*c4*(qd(1) + qd(2)) - s3*s4*(qd(1) + qd(2))) - s4*(c3*(qdd(1) + qdd(2)) - qd(3)*s3*(qd(1) + qd(2)))) + qd(5)*(-c5*(-qd(3) + qd(4)) - s5*(-c3*s4*(qd(1) + qd(2)) + c4*s3*(qd(1) + qd(2)))) - s5*(-qdd(3) + qdd(4))) - s6*(80*c5*(c4*(c3*qd(3)*(qd(1) + qd(2)) + s3*(qdd(1) + qdd(2))) + qd(4)*(-c3*c4*(qd(1) + qd(2)) - s3*s4*(qd(1) + qd(2))) - s4*(c3*(qdd(1) + qdd(2)) - qd(3)*s3*(qd(1) + qd(2)))) - c5*(-c2*(-c1*g + 270*qdd(1)) - 295*c3^2*(qd(1) + qd(2)) ^2 - 90*qdd(1) - 90*qdd(2) + s2*(-g*s1 - 270*qd(1)^2) - 295*s3^2*(qd(1) + qd(2)) ^2) + 80*qd(5)*(-c5*(-qd(3) + qd(4)) - s5*(-c3*s4*(qd(1) + qd(2)) + c4*s3*(qd(1) + qd(2)))) - 80*s5*(-qdd(3) + qdd(4)) - s5*(c4*(-295*c3*(qdd(1) + qdd(2)) + c3*(c2*(-g*s1 - 270*qd(1)^2) + s2*(-c1*g + 270*qdd(1)) - (qd(1) + qd(2))*(90*qd(1) + 90*qd(2)))) - s4*(295*s3*(qdd(1) + qdd(2)) - s3*(c2*(-g*s1 - 270*qd(1)^2) + s2*(-c1*g + 270*qdd(1)) - (qd(1) + qd(2))*(90*qd(1) + 90*qd(2))))) + (80*c5*(-qd(3) + qd(4)) + 80*s5*(-c3*s4*(qd(1) + qd(2)) + c4*s3*(qd(1) + qd(2))))*(-c3*c4*(qd(1) + qd(2)) + qd(5) - s3*s4*(qd(1) + qd(2)))) - (80*c6*(c5*(-c3*s4*(qd(1) + qd(2)) + c4*s3*(qd(1) + qd(2))) - s5*(-qd(3) + qd(4))) - 80*s6*(-c5*(-qd(3) + qd(4)) - s5*(-c3*s4*(qd(1) + qd(2)) + c4*s3*(qd(1) + qd(2)))))*(c3*c4*(qd(1) + qd(2)) - qd(5) + qd(6) + s3*s4*(qd(1) + qd(2)))) + 0.00744338*qd(3)*s3*(qd(1) + qd(2)) + 0.0436346*qdd(1) + 0.0436346*qdd(2) + 0.207558*qdd(3) + 75*s2*(c3*(c4*(c5*m7*(80*c6*(-c5*(-qdd(3) + qdd(4)) - qd(5)*(c5*(-c3*s4*(qd(1) + qd(2)) + c4*s3*(qd(1) + qd(2))) - s5*(-qd(3) + qd(4))) - s5*(c4*(c3*qd(3)*(qd(1) + qd(2)) + s3*(qdd(1) + qdd(2))) + qd(4)*(-c3*c4*(qd(1) + qd(2)) - s3*s4*(qd(1) + qd(2))) - s4*(c3*(qdd(1) + qdd(2)) - qd(3)*s3*(qd(1) + qd(2))))) + c6*(80*c5*(-qdd(3) + qdd(4)) + c5*(c4*(-295*c3*(qdd(1) + qdd(2)) + c3*(c2*(-g*s1 - 270*qd(1)^2) + s2*(-c1*g + 270*qdd(1)) - (qd(1) + qd(2))*(90*qd(1) + 90*qd(2)))) - s4*(295*s3*(qdd(1) + qdd(2)) - s3*(c2*(-g*s1 - 270*qd(1)^2) + s2*(-c1*g + 270*qdd(1)) - (qd(1) + qd(2))*(90*qd(1) + 90*qd(2))))) + 80*qd(5)*(c5*(-c3*s4*(qd(1) + qd(2)) + c4*s3*(qd(1) + qd(2))) - s5*(-qd(3) + qd(4))) + 80*s5*(c4*(c3*qd(3)*(qd(1) + qd(2)) + s3*(qdd(1) + qdd(2))) + qd(4)*(-c3*c4*(qd(1) + qd(2)) - s3*s4*(qd(1) + qd(2))) - s4*(c3*(qdd(1) + qdd(2)) - qd(3)*s3*(qd(1) + qd(2)))) - s5*(-c2*(-c1*g + 270*qdd(1)) - 295*c3^2*(qd(1) + qd(2)) ^2 - 90*qdd(1) - 90*qdd(2) + s2*(-g*s1 - 270*qd(1)^2) - 295*s3^2*(qd(1) + qd(2)) ^2) - (80*c5*(-c3*s4*(qd(1) + qd(2)) + c4*s3*(qd(1) + qd(2))) - 80*s5*(-qd(3) + qd(4)))*(-c3*c4*(qd(1) + qd(2)) + qd(5) - s3*s4*(qd(1) + qd(2)))) + 80*qd(6)*(c6*(c5*(-c3*s4*(qd(1) + qd(2)) + c4*s3*(qd(1) + qd(2))) - s5*(-qd(3) + qd(4))) - s6*(-c5*(-qd(3) + qd(4)) - s5*(-c3*s4*(qd(1) + qd(2)) + c4*s3*(qd(1) + qd(2))))) + 80*s6*(c5*(c4*(c3*qd(3)*(qd(1) + qd(2)) + s3*(qdd(1) + qdd(2))) + qd(4)*(-c3*c4*(qd(1) + qd(2)) - s3*s4*(qd(1) + qd(2))) - s4*(c3*(qdd(1) + qdd(2)) - qd(3)*s3*(qd(1) + qd(2)))) + qd(5)*(-c5*(-qd(3) + qd(4)) - s5*(-c3*s4*(qd(1) + qd(2)) + c4*s3*(qd(1) + qd(2)))) - s5*(-qdd(3) + qdd(4))) - s6*(80*c5*(c4*(c3*qd(3)*(qd(1) + qd(2)) + s3*(qdd(1) + qdd(2))) + qd(4)*(-c3*c4*(qd(1) + qd(2)) - s3*s4*(qd(1) + qd(2))) - s4*(c3*(qdd(1) + qdd(2)) - qd(3)*s3*(qd(1) + qd(2)))) - c5*(-c2*(-c1*g + 270*qdd(1)) - 295*c3^2*(qd(1) + qd(2)) ^2 - 90*qdd(1) - 90*qdd(2) + s2*(-g*s1 - 270*qd(1)^2) - 295*s3^2*(qd(1) + qd(2)) ^2) + 80*qd(5)*(-c5*(-qd(3) + qd(4)) - s5*(-c3*s4*(qd(1) + qd(2)) + c4*s3*(qd(1) + qd(2)))) - 80*s5*(-qdd(3) + qdd(4)) - s5*(c4*(-295*c3*(qdd(1) + qdd(2)) + c3*(c2*(-g*s1 - 270*qd(1)^2) + s2*(-c1*g + 270*qdd(1)) - (qd(1) + qd(2))*(90*qd(1) + 90*qd(2)))) - s4*(295*s3*(qdd(1) + qdd(2)) - s3*(c2*(-g*s1 - 270*qd(1)^2) + s2*(-c1*g + 270*qdd(1)) - (qd(1) + qd(2))*(90*qd(1) + 90*qd(2))))) + (80*c5*(-qd(3) + qd(4)) + 80*s5*(-c3*s4*(qd(1) + qd(2)) + c4*s3*(qd(1) + qd(2))))*(-c3*c4*(qd(1) + qd(2)) + qd(5) - s3*s4*(qd(1) + qd(2)))) - (80*c6*(c5*(-c3*s4*(qd(1) + qd(2)) + c4*s3*(qd(1) + qd(2))) - s5*(-qd(3) + qd(4))) - 80*s6*(-c5*(-qd(3) + qd(4)) - s5*(-c3*s4*(qd(1) + qd(2)) + c4*s3*(qd(1) + qd(2)))))*(c3*c4*(qd(1) + qd(2)) - qd(5) + qd(6) + s3*s4*(qd(1) + qd(2)))) + m6*(c5*(c4*(-295*c3*(qdd(1) + qdd(2)) + c3*(c2*(-g*s1 - 270*qd(1)^2) + s2*(-c1*g + 270*qdd(1)) - (qd(1) + qd(2))*(90*qd(1) + 90*qd(2)))) - s4*(295*s3*(qdd(1) + qdd(2)) - s3*(c2*(-g*s1 - 270*qd(1)^2) + s2*(-c1*g + 270*qdd(1)) - (qd(1) + qd(2))*(90*qd(1) + 90*qd(2))))) - s5*(-c2*(-c1*g + 270*qdd(1)) - 295*c3^2*(qd(1) + qd(2)) ^2 - 90*qdd(1) - 90*qdd(2) + s2*(-g*s1 - 270*qd(1)^2) - 295*s3^2*(qd(1) + qd(2)) ^2)) - m7*s5*(80*c6*(c5*(c4*(c3*qd(3)*(qd(1) + qd(2)) + s3*(qdd(1) + qdd(2))) + qd(4)*(-c3*c4*(qd(1) + qd(2)) - s3*s4*(qd(1) + qd(2))) - s4*(c3*(qdd(1) + qdd(2)) - qd(3)*s3*(qd(1) + qd(2)))) + qd(5)*(-c5*(-qd(3) + qd(4)) - s5*(-c3*s4*(qd(1) + qd(2)) + c4*s3*(qd(1) + qd(2)))) - s5*(-qdd(3) + qdd(4))) - c6*(80*c5*(c4*(c3*qd(3)*(qd(1) + qd(2)) + s3*(qdd(1) + qdd(2))) + qd(4)*(-c3*c4*(qd(1) + qd(2)) - s3*s4*(qd(1) + qd(2))) - s4*(c3*(qdd(1) + qdd(2)) - qd(3)*s3*(qd(1) + qd(2)))) - c5*(-c2*(-c1*g + 270*qdd(1)) - 295*c3^2*(qd(1) + qd(2)) ^2 - 90*qdd(1) - 90*qdd(2) + s2*(-g*s1 - 270*qd(1)^2) - 295*s3^2*(qd(1) + qd(2)) ^2) + 80*qd(5)*(-c5*(-qd(3) + qd(4)) - s5*(-c3*s4*(qd(1) + qd(2)) + c4*s3*(qd(1) + qd(2)))) - 80*s5*(-qdd(3) + qdd(4)) - s5*(c4*(-295*c3*(qdd(1) + qdd(2)) + c3*(c2*(-g*s1 - 270*qd(1)^2) + s2*(-c1*g + 270*qdd(1)) - (qd(1) + qd(2))*(90*qd(1) + 90*qd(2)))) - s4*(295*s3*(qdd(1) + qdd(2)) - s3*(c2*(-g*s1 - 270*qd(1)^2) + s2*(-c1*g + 270*qdd(1)) - (qd(1) + qd(2))*(90*qd(1) + 90*qd(2))))) + (80*c5*(-qd(3) + qd(4)) + 80*s5*(-c3*s4*(qd(1) + qd(2)) + c4*s3*(qd(1) + qd(2))))*(-c3*c4*(qd(1) + qd(2)) + qd(5) - s3*s4*(qd(1) + qd(2)))) + 80*qd(6)*(-c6*(-c5*(-qd(3) + qd(4)) - s5*(-c3*s4*(qd(1) + qd(2)) + c4*s3*(qd(1) + qd(2)))) - s6*(c5*(-c3*s4*(qd(1) + qd(2)) + c4*s3*(qd(1) + qd(2))) - s5*(-qd(3) + qd(4)))) - 80*s6*(-c5*(-qdd(3) + qdd(4)) - qd(5)*(c5*(-c3*s4*(qd(1) + qd(2)) + c4*s3*(qd(1) + qd(2))) - s5*(-qd(3) + qd(4))) - s5*(c4*(c3*qd(3)*(qd(1) + qd(2)) + s3*(qdd(1) + qdd(2))) + qd(4)*(-c3*c4*(qd(1) + qd(2)) - s3*s4*(qd(1) + qd(2))) - s4*(c3*(qdd(1) + qdd(2)) - qd(3)*s3*(qd(1) + qd(2))))) - s6*(80*c5*(-qdd(3) + qdd(4)) + c5*(c4*(-295*c3*(qdd(1) + qdd(2)) + c3*(c2*(-g*s1 - 270*qd(1)^2) + s2*(-c1*g + 270*qdd(1)) - (qd(1) + qd(2))*(90*qd(1) + 90*qd(2)))) - s4*(295*s3*(qdd(1) + qdd(2)) - s3*(c2*(-g*s1 - 270*qd(1)^2) + s2*(-c1*g + 270*qdd(1)) - (qd(1) + qd(2))*(90*qd(1) + 90*qd(2))))) + 80*qd(5)*(c5*(-c3*s4*(qd(1) + qd(2)) + c4*s3*(qd(1) + qd(2))) - s5*(-qd(3) + qd(4))) + 80*s5*(c4*(c3*qd(3)*(qd(1) + qd(2)) + s3*(qdd(1) + qdd(2))) + qd(4)*(-c3*c4*(qd(1) + qd(2)) - s3*s4*(qd(1) + qd(2))) - s4*(c3*(qdd(1) + qdd(2)) - qd(3)*s3*(qd(1) + qd(2)))) - s5*(-c2*(-c1*g + 270*qdd(1)) - 295*c3^2*(qd(1) + qd(2)) ^2 - 90*qdd(1) - 90*qdd(2) + s2*(-g*s1 - 270*qd(1)^2) - 295*s3^2*(qd(1) + qd(2)) ^2) - (80*c5*(-c3*s4*(qd(1) + qd(2)) + c4*s3*(qd(1) + qd(2))) - 80*s5*(-qd(3) + qd(4)))*(-c3*c4*(qd(1) + qd(2)) + qd(5) - s3*s4*(qd(1) + qd(2)))) + (80*c6*(-c5*(-qd(3) + qd(4)) - s5*(-c3*s4*(qd(1) + qd(2)) + c4*s3*(qd(1) + qd(2)))) + 80*s6*(c5*(-c3*s4*(qd(1) + qd(2)) + c4*s3*(qd(1) + qd(2))) - s5*(-qd(3) + qd(4))))*(c3*c4*(qd(1) + qd(2)) - qd(5) + qd(6) + s3*s4*(qd(1) + qd(2))))) + m5*(c4*(-295*c3*(qdd(1) + qdd(2)) + c3*(c2*(-g*s1 - 270*qd(1)^2) + s2*(-c1*g + 270*qdd(1)) - (qd(1) + qd(2))*(90*qd(1) + 90*qd(2)))) + 295*c4*(c3*(qdd(1) + qdd(2)) - qd(3)*s3*(qd(1) + qd(2))) + 295*qd(4)*(-c3*s4*(qd(1) + qd(2)) + c4*s3*(qd(1) + qd(2))) - s4*(295*s3*(qdd(1) + qdd(2)) - s3*(c2*(-g*s1 - 270*qd(1)^2) + s2*(-c1*g + 270*qdd(1)) - (qd(1) + qd(2))*(90*qd(1) + 90*qd(2)))) + 295*s4*(c3*qd(3)*(qd(1) + qd(2)) + s3*(qdd(1) + qdd(2))) - (-qd(3) + qd(4))*(-295*c3*s4*(qd(1) + qd(2)) + 295*c4*s3*(qd(1) + qd(2)))) - s4*(m6*(-c5*(-c2*(-c1*g + 270*qdd(1)) - 295*c3^2*(qd(1) + qd(2)) ^2 - 90*qdd(1) - 90*qdd(2) + s2*(-g*s1 - 270*qd(1)^2) - 295*s3^2*(qd(1) + qd(2)) ^2) - s5*(c4*(-295*c3*(qdd(1) + qdd(2)) + c3*(c2*(-g*s1 - 270*qd(1)^2) + s2*(-c1*g + 270*qdd(1)) - (qd(1) + qd(2))*(90*qd(1) + 90*qd(2)))) - s4*(295*s3*(qdd(1) + qdd(2)) - s3*(c2*(-g*s1 - 270*qd(1)^2) + s2*(-c1*g + 270*qdd(1)) - (qd(1) + qd(2))*(90*qd(1) + 90*qd(2)))))) + m7*(c4*(295*s3*(qdd(1) + qdd(2)) - s3*(c2*(-g*s1 - 270*qd(1)^2) + s2*(-c1*g + 270*qdd(1)) - (qd(1) + qd(2))*(90*qd(1) + 90*qd(2)))) + s4*(-295*c3*(qdd(1) + qdd(2)) + c3*(c2*(-g*s1 - 270*qd(1)^2) + s2*(-c1*g + 270*qdd(1)) - (qd(1) + qd(2))*(90*qd(1) + 90*qd(2)))) + (-c5*(-qd(3) + qd(4)) - s5*(-c3*s4*(qd(1) + qd(2)) + c4*s3*(qd(1) + qd(2))))*(80*c5*(-qd(3) + qd(4)) + 80*s5*(-c3*s4*(qd(1) + qd(2)) + c4*s3*(qd(1) + qd(2)))) - (c5*(-c3*s4*(qd(1) + qd(2)) + c4*s3*(qd(1) + qd(2))) - s5*(-qd(3) + qd(4)))*(80*c5*(-c3*s4*(qd(1) + qd(2)) + c4*s3*(qd(1) + qd(2))) - 80*s5*(-qd(3) + qd(4))) - (-c6*(-c5*(-qd(3) + qd(4)) - s5*(-c3*s4*(qd(1) + qd(2)) + c4*s3*(qd(1) + qd(2)))) - s6*(c5*(-c3*s4*(qd(1) + qd(2)) + c4*s3*(qd(1) + qd(2))) - s5*(-qd(3) + qd(4))))*(80*c6*(-c5*(-qd(3) + qd(4)) - s5*(-c3*s4*(qd(1) + qd(2)) + c4*s3*(qd(1) + qd(2)))) + 80*s6*(c5*(-c3*s4*(qd(1) + qd(2)) + c4*s3*(qd(1) + qd(2))) - s5*(-qd(3) + qd(4)))) + (c6*(c5*(-c3*s4*(qd(1) + qd(2)) + c4*s3*(qd(1) + qd(2))) - s5*(-qd(3) + qd(4))) - s6*(-c5*(-qd(3) + qd(4)) - s5*(-c3*s4*(qd(1) + qd(2)) + c4*s3*(qd(1) + qd(2)))))*(80*c6*(c5*(-c3*s4*(qd(1) + qd(2)) + c4*s3*(qd(1) + qd(2))) - s5*(-qd(3) + qd(4))) - 80*s6*(-c5*(-qd(3) + qd(4)) - s5*(-c3*s4*(qd(1) + qd(2)) + c4*s3*(qd(1) + qd(2)))))))) + m4*(-90*c3^2*(qd(1) + qd(2)) ^2 + c3*(c2*(-g*s1 - 270*qd(1)^2) + s2*(-c1*g + 270*qdd(1)) - (qd(1) + qd(2))*(90*qd(1) + 90*qd(2))) - 90*qd(3)^2) - s3*(-c4*(m6*(-c5*(-c2*(-c1*g + 270*qdd(1)) - 295*c3^2*(qd(1) + qd(2)) ^2 - 90*qdd(1) - 90*qdd(2) + s2*(-g*s1 - 270*qd(1)^2) - 295*s3^2*(qd(1) + qd(2)) ^2) - s5*(c4*(-295*c3*(qdd(1) + qdd(2)) + c3*(c2*(-g*s1 - 270*qd(1)^2) + s2*(-c1*g + 270*qdd(1)) - (qd(1) + qd(2))*(90*qd(1) + 90*qd(2)))) - s4*(295*s3*(qdd(1) + qdd(2)) - s3*(c2*(-g*s1 - 270*qd(1)^2) + s2*(-c1*g + 270*qdd(1)) - (qd(1) + qd(2))*(90*qd(1) + 90*qd(2)))))) + m7*(c4*(295*s3*(qdd(1) + qdd(2)) - s3*(c2*(-g*s1 - 270*qd(1)^2) + s2*(-c1*g + 270*qdd(1)) - (qd(1) + qd(2))*(90*qd(1) + 90*qd(2)))) + s4*(-295*c3*(qdd(1) + qdd(2)) + c3*(c2*(-g*s1 - 270*qd(1)^2) + s2*(-c1*g + 270*qdd(1)) - (qd(1) + qd(2))*(90*qd(1) + 90*qd(2)))) + (-c5*(-qd(3) + qd(4)) - s5*(-c3*s4*(qd(1) + qd(2)) + c4*s3*(qd(1) + qd(2))))*(80*c5*(-qd(3) + qd(4)) + 80*s5*(-c3*s4*(qd(1) + qd(2)) + c4*s3*(qd(1) + qd(2)))) - (c5*(-c3*s4*(qd(1) + qd(2)) + c4*s3*(qd(1) + qd(2))) - s5*(-qd(3) + qd(4)))*(80*c5*(-c3*s4*(qd(1) + qd(2)) + c4*s3*(qd(1) + qd(2))) - 80*s5*(-qd(3) + qd(4))) - (-c6*(-c5*(-qd(3) + qd(4)) - s5*(-c3*s4*(qd(1) + qd(2)) + c4*s3*(qd(1) + qd(2)))) - s6*(c5*(-c3*s4*(qd(1) + qd(2)) + c4*s3*(qd(1) + qd(2))) - s5*(-qd(3) + qd(4))))*(80*c6*(-c5*(-qd(3) + qd(4)) - s5*(-c3*s4*(qd(1) + qd(2)) + c4*s3*(qd(1) + qd(2)))) + 80*s6*(c5*(-c3*s4*(qd(1) + qd(2)) + c4*s3*(qd(1) + qd(2))) - s5*(-qd(3) + qd(4)))) + (c6*(c5*(-c3*s4*(qd(1) + qd(2)) + c4*s3*(qd(1) + qd(2))) - s5*(-qd(3) + qd(4))) - s6*(-c5*(-qd(3) + qd(4)) - s5*(-c3*s4*(qd(1) + qd(2)) + c4*s3*(qd(1) + qd(2)))))*(80*c6*(c5*(-c3*s4*(qd(1) + qd(2)) + c4*s3*(qd(1) + qd(2))) - s5*(-qd(3) + qd(4))) - 80*s6*(-c5*(-qd(3) + qd(4)) - s5*(-c3*s4*(qd(1) + qd(2)) + c4*s3*(qd(1) + qd(2))))))) + m5*(-c4*(295*s3*(qdd(1) + qdd(2)) - s3*(c2*(-g*s1 - 270*qd(1)^2) + s2*(-c1*g + 270*qdd(1)) - (qd(1) + qd(2))*(90*qd(1) + 90*qd(2)))) + 295*c4*(c3*qd(3)*(qd(1) + qd(2)) + s3*(qdd(1) + qdd(2))) + 295*qd(4)*(-c3*c4*(qd(1) + qd(2)) - s3*s4*(qd(1) + qd(2))) - s4*(-295*c3*(qdd(1) + qdd(2)) + c3*(c2*(-g*s1 - 270*qd(1)^2) + s2*(-c1*g + 270*qdd(1)) - (qd(1) + qd(2))*(90*qd(1) + 90*qd(2)))) - 295*s4*(c3*(qdd(1) + qdd(2)) - qd(3)*s3*(qd(1) + qd(2))) + (-qd(3) + qd(4))*(295*c3*c4*(qd(1) + qd(2)) + 295*s3*s4*(qd(1) + qd(2)))) - s4*(c5*m7*(80*c6*(-c5*(-qdd(3) + qdd(4)) - qd(5)*(c5*(-c3*s4*(qd(1) + qd(2)) + c4*s3*(qd(1) + qd(2))) - s5*(-qd(3) + qd(4))) - s5*(c4*(c3*qd(3)*(qd(1) + qd(2)) + s3*(qdd(1) + qdd(2))) + qd(4)*(-c3*c4*(qd(1) + qd(2)) - s3*s4*(qd(1) + qd(2))) - s4*(c3*(qdd(1) + qdd(2)) - qd(3)*s3*(qd(1) + qd(2))))) + c6*(80*c5*(-qdd(3) + qdd(4)) + c5*(c4*(-295*c3*(qdd(1) + qdd(2)) + c3*(c2*(-g*s1 - 270*qd(1)^2) + s2*(-c1*g + 270*qdd(1)) - (qd(1) + qd(2))*(90*qd(1) + 90*qd(2)))) - s4*(295*s3*(qdd(1) + qdd(2)) - s3*(c2*(-g*s1 - 270*qd(1)^2) + s2*(-c1*g + 270*qdd(1)) - (qd(1) + qd(2))*(90*qd(1) + 90*qd(2))))) + 80*qd(5)*(c5*(-c3*s4*(qd(1) + qd(2)) + c4*s3*(qd(1) + qd(2))) - s5*(-qd(3) + qd(4))) + 80*s5*(c4*(c3*qd(3)*(qd(1) + qd(2)) + s3*(qdd(1) + qdd(2))) + qd(4)*(-c3*c4*(qd(1) + qd(2)) - s3*s4*(qd(1) + qd(2))) - s4*(c3*(qdd(1) + qdd(2)) - qd(3)*s3*(qd(1) + qd(2)))) - s5*(-c2*(-c1*g + 270*qdd(1)) - 295*c3^2*(qd(1) + qd(2)) ^2 - 90*qdd(1) - 90*qdd(2) + s2*(-g*s1 - 270*qd(1)^2) - 295*s3^2*(qd(1) + qd(2)) ^2) - (80*c5*(-c3*s4*(qd(1) + qd(2)) + c4*s3*(qd(1) + qd(2))) - 80*s5*(-qd(3) + qd(4)))*(-c3*c4*(qd(1) + qd(2)) + qd(5) - s3*s4*(qd(1) + qd(2)))) + 80*qd(6)*(c6*(c5*(-c3*s4*(qd(1) + qd(2)) + c4*s3*(qd(1) + qd(2))) - s5*(-qd(3) + qd(4))) - s6*(-c5*(-qd(3) + qd(4)) - s5*(-c3*s4*(qd(1) + qd(2)) + c4*s3*(qd(1) + qd(2))))) + 80*s6*(c5*(c4*(c3*qd(3)*(qd(1) + qd(2)) + s3*(qdd(1) + qdd(2))) + qd(4)*(-c3*c4*(qd(1) + qd(2)) - s3*s4*(qd(1) + qd(2))) - s4*(c3*(qdd(1) + qdd(2)) - qd(3)*s3*(qd(1) + qd(2)))) + qd(5)*(-c5*(-qd(3) + qd(4)) - s5*(-c3*s4*(qd(1) + qd(2)) + c4*s3*(qd(1) + qd(2)))) - s5*(-qdd(3) + qdd(4))) - s6*(80*c5*(c4*(c3*qd(3)*(qd(1) + qd(2)) + s3*(qdd(1) + qdd(2))) + qd(4)*(-c3*c4*(qd(1) + qd(2)) - s3*s4*(qd(1) + qd(2))) - s4*(c3*(qdd(1) + qdd(2)) - qd(3)*s3*(qd(1) + qd(2)))) - c5*(-c2*(-c1*g + 270*qdd(1)) - 295*c3^2*(qd(1) + qd(2)) ^2 - 90*qdd(1) - 90*qdd(2) + s2*(-g*s1 - 270*qd(1)^2) - 295*s3^2*(qd(1) + qd(2)) ^2) + 80*qd(5)*(-c5*(-qd(3) + qd(4)) - s5*(-c3*s4*(qd(1) + qd(2)) + c4*s3*(qd(1) + qd(2)))) - 80*s5*(-qdd(3) + qdd(4)) - s5*(c4*(-295*c3*(qdd(1) + qdd(2)) + c3*(c2*(-g*s1 - 270*qd(1)^2) + s2*(-c1*g + 270*qdd(1)) - (qd(1) + qd(2))*(90*qd(1) + 90*qd(2)))) - s4*(295*s3*(qdd(1) + qdd(2)) - s3*(c2*(-g*s1 - 270*qd(1)^2) + s2*(-c1*g + 270*qdd(1)) - (qd(1) + qd(2))*(90*qd(1) + 90*qd(2))))) + (80*c5*(-qd(3) + qd(4)) + 80*s5*(-c3*s4*(qd(1) + qd(2)) + c4*s3*(qd(1) + qd(2))))*(-c3*c4*(qd(1) + qd(2)) + qd(5) - s3*s4*(qd(1) + qd(2)))) - (80*c6*(c5*(-c3*s4*(qd(1) + qd(2)) + c4*s3*(qd(1) + qd(2))) - s5*(-qd(3) + qd(4))) - 80*s6*(-c5*(-qd(3) + qd(4)) - s5*(-c3*s4*(qd(1) + qd(2)) + c4*s3*(qd(1) + qd(2)))))*(c3*c4*(qd(1) + qd(2)) - qd(5) + qd(6) + s3*s4*(qd(1) + qd(2)))) + m6*(c5*(c4*(-295*c3*(qdd(1) + qdd(2)) + c3*(c2*(-g*s1 - 270*qd(1)^2) + s2*(-c1*g + 270*qdd(1)) - (qd(1) + qd(2))*(90*qd(1) + 90*qd(2)))) - s4*(295*s3*(qdd(1) + qdd(2)) - s3*(c2*(-g*s1 - 270*qd(1)^2) + s2*(-c1*g + 270*qdd(1)) - (qd(1) + qd(2))*(90*qd(1) + 90*qd(2))))) - s5*(-c2*(-c1*g + 270*qdd(1)) - 295*c3^2*(qd(1) + qd(2)) ^2 - 90*qdd(1) - 90*qdd(2) + s2*(-g*s1 - 270*qd(1)^2) - 295*s3^2*(qd(1) + qd(2)) ^2)) - m7*s5*(80*c6*(c5*(c4*(c3*qd(3)*(qd(1) + qd(2)) + s3*(qdd(1) + qdd(2))) + qd(4)*(-c3*c4*(qd(1) + qd(2)) - s3*s4*(qd(1) + qd(2))) - s4*(c3*(qdd(1) + qdd(2)) - qd(3)*s3*(qd(1) + qd(2)))) + qd(5)*(-c5*(-qd(3) + qd(4)) - s5*(-c3*s4*(qd(1) + qd(2)) + c4*s3*(qd(1) + qd(2)))) - s5*(-qdd(3) + qdd(4))) - c6*(80*c5*(c4*(c3*qd(3)*(qd(1) + qd(2)) + s3*(qdd(1) + qdd(2))) + qd(4)*(-c3*c4*(qd(1) + qd(2)) - s3*s4*(qd(1) + qd(2))) - s4*(c3*(qdd(1) + qdd(2)) - qd(3)*s3*(qd(1) + qd(2)))) - c5*(-c2*(-c1*g + 270*qdd(1)) - 295*c3^2*(qd(1) + qd(2)) ^2 - 90*qdd(1) - 90*qdd(2) + s2*(-g*s1 - 270*qd(1)^2) - 295*s3^2*(qd(1) + qd(2)) ^2) + 80*qd(5)*(-c5*(-qd(3) + qd(4)) - s5*(-c3*s4*(qd(1) + qd(2)) + c4*s3*(qd(1) + qd(2)))) - 80*s5*(-qdd(3) + qdd(4)) - s5*(c4*(-295*c3*(qdd(1) + qdd(2)) + c3*(c2*(-g*s1 - 270*qd(1)^2) + s2*(-c1*g + 270*qdd(1)) - (qd(1) + qd(2))*(90*qd(1) + 90*qd(2)))) - s4*(295*s3*(qdd(1) + qdd(2)) - s3*(c2*(-g*s1 - 270*qd(1)^2) + s2*(-c1*g + 270*qdd(1)) - (qd(1) + qd(2))*(90*qd(1) + 90*qd(2))))) + (80*c5*(-qd(3) + qd(4)) + 80*s5*(-c3*s4*(qd(1) + qd(2)) + c4*s3*(qd(1) + qd(2))))*(-c3*c4*(qd(1) + qd(2)) + qd(5) - s3*s4*(qd(1) + qd(2)))) + 80*qd(6)*(-c6*(-c5*(-qd(3) + qd(4)) - s5*(-c3*s4*(qd(1) + qd(2)) + c4*s3*(qd(1) + qd(2)))) - s6*(c5*(-c3*s4*(qd(1) + qd(2)) + c4*s3*(qd(1) + qd(2))) - s5*(-qd(3) + qd(4)))) - 80*s6*(-c5*(-qdd(3) + qdd(4)) - qd(5)*(c5*(-c3*s4*(qd(1) + qd(2)) + c4*s3*(qd(1) + qd(2))) - s5*(-qd(3) + qd(4))) - s5*(c4*(c3*qd(3)*(qd(1) + qd(2)) + s3*(qdd(1) + qdd(2))) + qd(4)*(-c3*c4*(qd(1) + qd(2)) - s3*s4*(qd(1) + qd(2))) - s4*(c3*(qdd(1) + qdd(2)) - qd(3)*s3*(qd(1) + qd(2))))) - s6*(80*c5*(-qdd(3) + qdd(4)) + c5*(c4*(-295*c3*(qdd(1) + qdd(2)) + c3*(c2*(-g*s1 - 270*qd(1)^2) + s2*(-c1*g + 270*qdd(1)) - (qd(1) + qd(2))*(90*qd(1) + 90*qd(2)))) - s4*(295*s3*(qdd(1) + qdd(2)) - s3*(c2*(-g*s1 - 270*qd(1)^2) + s2*(-c1*g + 270*qdd(1)) - (qd(1) + qd(2))*(90*qd(1) + 90*qd(2))))) + 80*qd(5)*(c5*(-c3*s4*(qd(1) + qd(2)) + c4*s3*(qd(1) + qd(2))) - s5*(-qd(3) + qd(4))) + 80*s5*(c4*(c3*qd(3)*(qd(1) + qd(2)) + s3*(qdd(1) + qdd(2))) + qd(4)*(-c3*c4*(qd(1) + qd(2)) - s3*s4*(qd(1) + qd(2))) - s4*(c3*(qdd(1) + qdd(2)) - qd(3)*s3*(qd(1) + qd(2)))) - s5*(-c2*(-c1*g + 270*qdd(1)) - 295*c3^2*(qd(1) + qd(2)) ^2 - 90*qdd(1) - 90*qdd(2) + s2*(-g*s1 - 270*qd(1)^2) - 295*s3^2*(qd(1) + qd(2)) ^2) - (80*c5*(-c3*s4*(qd(1) + qd(2)) + c4*s3*(qd(1) + qd(2))) - 80*s5*(-qd(3) + qd(4)))*(-c3*c4*(qd(1) + qd(2)) + qd(5) - s3*s4*(qd(1) + qd(2)))) + (80*c6*(-c5*(-qd(3) + qd(4)) - s5*(-c3*s4*(qd(1) + qd(2)) + c4*s3*(qd(1) + qd(2)))) + 80*s6*(c5*(-c3*s4*(qd(1) + qd(2)) + c4*s3*(qd(1) + qd(2))) - s5*(-qd(3) + qd(4))))*(c3*c4*(qd(1) + qd(2)) - qd(5) + qd(6) + s3*s4*(qd(1) + qd(2))))))) + 335*s2*(c5*m7*(80*c6*(c5*(c4*(c3*qd(3)*(qd(1) + qd(2)) + s3*(qdd(1) + qdd(2))) + qd(4)*(-c3*c4*(qd(1) + qd(2)) - s3*s4*(qd(1) + qd(2))) - s4*(c3*(qdd(1) + qdd(2)) - qd(3)*s3*(qd(1) + qd(2)))) + qd(5)*(-c5*(-qd(3) + qd(4)) - s5*(-c3*s4*(qd(1) + qd(2)) + c4*s3*(qd(1) + qd(2)))) - s5*(-qdd(3) + qdd(4))) - c6*(80*c5*(c4*(c3*qd(3)*(qd(1) + qd(2)) + s3*(qdd(1) + qdd(2))) + qd(4)*(-c3*c4*(qd(1) + qd(2)) - s3*s4*(qd(1) + qd(2))) - s4*(c3*(qdd(1) + qdd(2)) - qd(3)*s3*(qd(1) + qd(2)))) - c5*(-c2*(-c1*g + 270*qdd(1)) - 295*c3^2*(qd(1) + qd(2)) ^2 - 90*qdd(1) - 90*qdd(2) + s2*(-g*s1 - 270*qd(1)^2) - 295*s3^2*(qd(1) + qd(2)) ^2) + 80*qd(5)*(-c5*(-qd(3) + qd(4)) - s5*(-c3*s4*(qd(1) + qd(2)) + c4*s3*(qd(1) + qd(2)))) - 80*s5*(-qdd(3) + qdd(4)) - s5*(c4*(-295*c3*(qdd(1) + qdd(2)) + c3*(c2*(-g*s1 - 270*qd(1)^2) + s2*(-c1*g + 270*qdd(1)) - (qd(1) + qd(2))*(90*qd(1) + 90*qd(2)))) - s4*(295*s3*(qdd(1) + qdd(2)) - s3*(c2*(-g*s1 - 270*qd(1)^2) + s2*(-c1*g + 270*qdd(1)) - (qd(1) + qd(2))*(90*qd(1) + 90*qd(2))))) + (80*c5*(-qd(3) + qd(4)) + 80*s5*(-c3*s4*(qd(1) + qd(2)) + c4*s3*(qd(1) + qd(2))))*(-c3*c4*(qd(1) + qd(2)) + qd(5) - s3*s4*(qd(1) + qd(2)))) + 80*qd(6)*(-c6*(-c5*(-qd(3) + qd(4)) - s5*(-c3*s4*(qd(1) + qd(2)) + c4*s3*(qd(1) + qd(2)))) - s6*(c5*(-c3*s4*(qd(1) + qd(2)) + c4*s3*(qd(1) + qd(2))) - s5*(-qd(3) + qd(4)))) - 80*s6*(-c5*(-qdd(3) + qdd(4)) - qd(5)*(c5*(-c3*s4*(qd(1) + qd(2)) + c4*s3*(qd(1) + qd(2))) - s5*(-qd(3) + qd(4))) - s5*(c4*(c3*qd(3)*(qd(1) + qd(2)) + s3*(qdd(1) + qdd(2))) + qd(4)*(-c3*c4*(qd(1) + qd(2)) - s3*s4*(qd(1) + qd(2))) - s4*(c3*(qdd(1) + qdd(2)) - qd(3)*s3*(qd(1) + qd(2))))) - s6*(80*c5*(-qdd(3) + qdd(4)) + c5*(c4*(-295*c3*(qdd(1) + qdd(2)) + c3*(c2*(-g*s1 - 270*qd(1)^2) + s2*(-c1*g + 270*qdd(1)) - (qd(1) + qd(2))*(90*qd(1) + 90*qd(2)))) - s4*(295*s3*(qdd(1) + qdd(2)) - s3*(c2*(-g*s1 - 270*qd(1)^2) + s2*(-c1*g + 270*qdd(1)) - (qd(1) + qd(2))*(90*qd(1) + 90*qd(2))))) + 80*qd(5)*(c5*(-c3*s4*(qd(1) + qd(2)) + c4*s3*(qd(1) + qd(2))) - s5*(-qd(3) + qd(4))) + 80*s5*(c4*(c3*qd(3)*(qd(1) + qd(2)) + s3*(qdd(1) + qdd(2))) + qd(4)*(-c3*c4*(qd(1) + qd(2)) - s3*s4*(qd(1) + qd(2))) - s4*(c3*(qdd(1) + qdd(2)) - qd(3)*s3*(qd(1) + qd(2)))) - s5*(-c2*(-c1*g + 270*qdd(1)) - 295*c3^2*(qd(1) + qd(2)) ^2 - 90*qdd(1) - 90*qdd(2) + s2*(-g*s1 - 270*qd(1)^2) - 295*s3^2*(qd(1) + qd(2)) ^2) - (80*c5*(-c3*s4*(qd(1) + qd(2)) + c4*s3*(qd(1) + qd(2))) - 80*s5*(-qd(3) + qd(4)))*(-c3*c4*(qd(1) + qd(2)) + qd(5) - s3*s4*(qd(1) + qd(2)))) + (80*c6*(-c5*(-qd(3) + qd(4)) - s5*(-c3*s4*(qd(1) + qd(2)) + c4*s3*(qd(1) + qd(2)))) + 80*s6*(c5*(-c3*s4*(qd(1) + qd(2)) + c4*s3*(qd(1) + qd(2))) - s5*(-qd(3) + qd(4))))*(c3*c4*(qd(1) + qd(2)) - qd(5) + qd(6) + s3*s4*(qd(1) + qd(2)))) + m4*(90*c3*s3*(qd(1) + qd(2)) ^2 + 90*qdd(3) - s3*(c2*(-g*s1 - 270*qd(1)^2) + s2*(-c1*g + 270*qdd(1)) - (qd(1) + qd(2))*(90*qd(1) + 90*qd(2)))) + m5*(-c2*(-c1*g + 270*qdd(1)) - 295*c3^2*(qd(1) + qd(2)) ^2 - 90*qdd(1) - 90*qdd(2) + s2*(-g*s1 - 270*qd(1)^2) - 295*s3^2*(qd(1) + qd(2)) ^2 - (-c3*c4*(qd(1) + qd(2)) - s3*s4*(qd(1) + qd(2)))*(295*c3*c4*(qd(1) + qd(2)) + 295*s3*s4*(qd(1) + qd(2))) + (-295*c3*s4*(qd(1) + qd(2)) + 295*c4*s3*(qd(1) + qd(2)))*(-c3*s4*(qd(1) + qd(2)) + c4*s3*(qd(1) + qd(2)))) - m6*(-c4*(295*s3*(qdd(1) + qdd(2)) - s3*(c2*(-g*s1 - 270*qd(1)^2) + s2*(-c1*g + 270*qdd(1)) - (qd(1) + qd(2))*(90*qd(1) + 90*qd(2)))) - s4*(-295*c3*(qdd(1) + qdd(2)) + c3*(c2*(-g*s1 - 270*qd(1)^2) + s2*(-c1*g + 270*qdd(1)) - (qd(1) + qd(2))*(90*qd(1) + 90*qd(2))))) + m7*s5*(80*c6*(-c5*(-qdd(3) + qdd(4)) - qd(5)*(c5*(-c3*s4*(qd(1) + qd(2)) + c4*s3*(qd(1) + qd(2))) - s5*(-qd(3) + qd(4))) - s5*(c4*(c3*qd(3)*(qd(1) + qd(2)) + s3*(qdd(1) + qdd(2))) + qd(4)*(-c3*c4*(qd(1) + qd(2)) - s3*s4*(qd(1) + qd(2))) - s4*(c3*(qdd(1) + qdd(2)) - qd(3)*s3*(qd(1) + qd(2))))) + c6*(80*c5*(-qdd(3) + qdd(4)) + c5*(c4*(-295*c3*(qdd(1) + qdd(2)) + c3*(c2*(-g*s1 - 270*qd(1)^2) + s2*(-c1*g + 270*qdd(1)) - (qd(1) + qd(2))*(90*qd(1) + 90*qd(2)))) - s4*(295*s3*(qdd(1) + qdd(2)) - s3*(c2*(-g*s1 - 270*qd(1)^2) + s2*(-c1*g + 270*qdd(1)) - (qd(1) + qd(2))*(90*qd(1) + 90*qd(2))))) + 80*qd(5)*(c5*(-c3*s4*(qd(1) + qd(2)) + c4*s3*(qd(1) + qd(2))) - s5*(-qd(3) + qd(4))) + 80*s5*(c4*(c3*qd(3)*(qd(1) + qd(2)) + s3*(qdd(1) + qdd(2))) + qd(4)*(-c3*c4*(qd(1) + qd(2)) - s3*s4*(qd(1) + qd(2))) - s4*(c3*(qdd(1) + qdd(2)) - qd(3)*s3*(qd(1) + qd(2)))) - s5*(-c2*(-c1*g + 270*qdd(1)) - 295*c3^2*(qd(1) + qd(2)) ^2- 90*qdd(1) - 90*qdd(2) + s2*(-g*s1 - 270*qd(1)^2) - 295*s3^2*(qd(1) + qd(2)) ^2) - (80*c5*(-c3*s4*(qd(1) + qd(2)) + c4*s3*(qd(1) + qd(2))) - 80*s5*(-qd(3) + qd(4)))*(-c3*c4*(qd(1) + qd(2)) + qd(5) - s3*s4*(qd(1) + qd(2)))) + 80*qd(6)*(c6*(c5*(-c3*s4*(qd(1) + qd(2)) + c4*s3*(qd(1) + qd(2))) - s5*(-qd(3) + qd(4))) - s6*(-c5*(-qd(3) + qd(4)) - s5*(-c3*s4*(qd(1) + qd(2)) + c4*s3*(qd(1) + qd(2))))) + 80*s6*(c5*(c4*(c3*qd(3)*(qd(1) + qd(2)) + s3*(qdd(1) + qdd(2))) + qd(4)*(-c3*c4*(qd(1) + qd(2)) - s3*s4*(qd(1) + qd(2))) - s4*(c3*(qdd(1) + qdd(2)) - qd(3)*s3*(qd(1) + qd(2)))) + qd(5)*(-c5*(-qd(3) + qd(4)) - s5*(-c3*s4*(qd(1) + qd(2)) + c4*s3*(qd(1) + qd(2)))) - s5*(-qdd(3) + qdd(4))) - s6*(80*c5*(c4*(c3*qd(3)*(qd(1) + qd(2)) + s3*(qdd(1) + qdd(2))) + qd(4)*(-c3*c4*(qd(1) + qd(2)) - s3*s4*(qd(1) + qd(2))) - s4*(c3*(qdd(1) + qdd(2)) - qd(3)*s3*(qd(1) + qd(2)))) - c5*(-c2*(-c1*g + 270*qdd(1)) - 295*c3^2*(qd(1) + qd(2)) ^2 - 90*qdd(1) - 90*qdd(2) + s2*(-g*s1 - 270*qd(1)^2) - 295*s3^2*(qd(1) + qd(2)) ^2) + 80*qd(5)*(-c5*(-qd(3) + qd(4)) - s5*(-c3*s4*(qd(1) + qd(2)) + c4*s3*(qd(1) + qd(2)))) - 80*s5*(-qdd(3) + qdd(4)) - s5*(c4*(-295*c3*(qdd(1) + qdd(2)) + c3*(c2*(-g*s1 - 270*qd(1)^2) + s2*(-c1*g + 270*qdd(1)) - (qd(1) + qd(2))*(90*qd(1) + 90*qd(2)))) - s4*(295*s3*(qdd(1) + qdd(2)) - s3*(c2*(-g*s1 - 270*qd(1)^2) + s2*(-c1*g + 270*qdd(1)) - (qd(1) + qd(2))*(90*qd(1) + 90*qd(2))))) + (80*c5*(-qd(3) + qd(4)) + 80*s5*(-c3*s4*(qd(1) + qd(2)) + c4*s3*(qd(1) + qd(2))))*(-c3*c4*(qd(1) + qd(2)) + qd(5) - s3*s4*(qd(1) + qd(2)))) - (80*c6*(c5*(-c3*s4*(qd(1) + qd(2)) + c4*s3*(qd(1) + qd(2))) - s5*(-qd(3) + qd(4))) - 80*s6*(-c5*(-qd(3) + qd(4)) - s5*(-c3*s4*(qd(1) + qd(2)) + c4*s3*(qd(1) + qd(2)))))*(c3*c4*(qd(1) + qd(2)) - qd(5) + qd(6) + s3*s4*(qd(1) + qd(2))))) + s3*(qd(1) + qd(2))*(0.750399*c3*(qd(1) + qd(2)) - 0.00744338*qd(3) - 0.00947011*s3*(qd(1) + qd(2))) - 0.0247925*s3*(qdd(1) + qdd(2)) + s3*(0.00163355*c4*(c3*(qdd(1) + qdd(2)) - qd(3)*s3*(qd(1) + qd(2))) + 0.00950111*c4*(c3*qd(3)*(qd(1) + qd(2)) + s3*(qdd(1) + qdd(2))) + c4*(0.000409305*c5*(-qdd(3) + qdd(4)) + 0.00151607*c5*(c4*(c3*qd(3)*(qd(1) + qd(2)) + s3*(qdd(1) + qdd(2))) + qd(4)*(-c3*c4*(qd(1) + qd(2)) - s3*s4*(qd(1) + qd(2))) - s4*(c3*(qdd(1) + qdd(2)) - qd(3)*s3*(qd(1) + qd(2)))) + c5*(6.20477e-6*c6*(c5*(c4*(c3*qd(3)*(qd(1) + qd(2)) + s3*(qdd(1) + qdd(2))) + qd(4)*(-c3*c4*(qd(1) + qd(2)) - s3*s4*(qd(1) + qd(2))) - s4*(c3*(qdd(1) + qdd(2)) - qd(3)*s3*(qd(1) + qd(2)))) + qd(5)*(-c5*(-qd(3) + qd(4)) - s5*(-c3*s4*(qd(1) + qd(2)) + c4*s3*(qd(1) + qd(2)))) - s5*(-qdd(3) + qdd(4))) + 6.20477e-6*qd(6)*(-c6*(-c5*(-qd(3) + qd(4)) - s5*(-c3*s4*(qd(1) + qd(2)) + c4*s3*(qd(1) + qd(2)))) - s6*(c5*(-c3*s4*(qd(1) + qd(2)) + c4*s3*(qd(1) + qd(2))) - s5*(-qd(3) + qd(4)))) - 6.20477e-6*s6*(-c5*(-qdd(3) + qdd(4)) - qd(5)*(c5*(-c3*s4*(qd(1) + qd(2)) + c4*s3*(qd(1) + qd(2))) - s5*(-qd(3) + qd(4))) - s5*(c4*(c3*qd(3)*(qd(1) + qd(2)) + s3*(qdd(1) + qdd(2))) + qd(4)*(-c3*c4*(qd(1) + qd(2)) - s3*s4*(qd(1) + qd(2))) - s4*(c3*(qdd(1) + qdd(2)) - qd(3)*s3*(qd(1) + qd(2))))) + (-c6*(-c5*(-qd(3) + qd(4)) - s5*(-c3*s4*(qd(1) + qd(2)) + c4*s3*(qd(1) + qd(2)))) - s6*(c5*(-c3*s4*(qd(1) + qd(2)) + c4*s3*(qd(1) + qd(2))) - s5*(-qd(3) + qd(4))))*(3.29301e-6*c3*c4*(qd(1) + qd(2)) - 3.29301e-6*qd(5) + 3.29301e-6*qd(6) + 3.29301e-6*s3*s4*(qd(1) + qd(2))) - (-3.01352e-6*c6*(-c5*(-qd(3) + qd(4)) - s5*(-c3*s4*(qd(1) + qd(2)) + c4*s3*(qd(1) + qd(2)))) - 3.01352e-6*s6*(c5*(-c3*s4*(qd(1) + qd(2)) + c4*s3*(qd(1) + qd(2))) - s5*(-qd(3) + qd(4))))*(c3*c4*(qd(1) + qd(2)) - qd(5) + qd(6) + s3*s4*(qd(1) + qd(2)))) + 295*m6*(-c5*(-c2*(-c1*g + 270*qdd(1)) - 295*c3^2*(qd(1) + qd(2))^2 - 90*qdd(1) - 90*qdd(2) + s2*(-g*s1 - 270*qd(1)^2) - 295*s3^2*(qd(1) + qd(2)) ^2) - s5*(c4*(-295*c3*(qdd(1) + qdd(2)) + c3*(c2*(-g*s1 - 270*qd(1)^2) + s2*(-c1*g + 270*qdd(1)) - (qd(1) + qd(2))*(90*qd(1) + 90*qd(2)))) - s4*(295*s3*(qdd(1) + qdd(2)) - s3*(c2*(-g*s1 - 270*qd(1)^2) + s2*(-c1*g + 270*qdd(1)) - (qd(1) + qd(2))*(90*qd(1) + 90*qd(2)))))) + 295*m7*(c4*(295*s3*(qdd(1) + qdd(2)) - s3*(c2*(-g*s1 - 270*qd(1)^2) + s2*(-c1*g + 270*qdd(1)) - (qd(1) + qd(2))*(90*qd(1) + 90*qd(2)))) + s4*(-295*c3*(qdd(1) + qdd(2)) + c3*(c2*(-g*s1 - 270*qd(1)^2) + s2*(-c1*g + 270*qdd(1)) - (qd(1) + qd(2))*(90*qd(1) + 90*qd(2)))) + (-c5*(-qd(3) + qd(4)) - s5*(-c3*s4*(qd(1) + qd(2)) + c4*s3*(qd(1) + qd(2))))*(80*c5*(-qd(3) + qd(4)) + 80*s5*(-c3*s4*(qd(1) + qd(2)) + c4*s3*(qd(1) + qd(2)))) - (c5*(-c3*s4*(qd(1) + qd(2)) + c4*s3*(qd(1) + qd(2))) - s5*(-qd(3) + qd(4)))*(80*c5*(-c3*s4*(qd(1) + qd(2)) + c4*s3*(qd(1) + qd(2))) - 80*s5*(-qd(3) + qd(4))) - (-c6*(-c5*(-qd(3) + qd(4)) - s5*(-c3*s4*(qd(1) + qd(2)) + c4*s3*(qd(1) + qd(2)))) - s6*(c5*(-c3*s4*(qd(1) + qd(2)) + c4*s3*(qd(1) + qd(2))) - s5*(-qd(3) + qd(4))))*(80*c6*(-c5*(-qd(3) + qd(4)) - s5*(-c3*s4*(qd(1) + qd(2)) + c4*s3*(qd(1) + qd(2)))) + 80*s6*(c5*(-c3*s4*(qd(1) + qd(2)) + c4*s3*(qd(1) + qd(2))) - s5*(-qd(3) + qd(4)))) + (c6*(c5*(-c3*s4*(qd(1) + qd(2)) + c4*s3*(qd(1) + qd(2))) - s5*(-qd(3) + qd(4))) - s6*(-c5*(-qd(3) + qd(4)) - s5*(-c3*s4*(qd(1) + qd(2)) + c4*s3*(qd(1) + qd(2)))))*(80*c6*(c5*(-c3*s4*(qd(1) + qd(2)) + c4*s3*(qd(1) + qd(2))) - s5*(-qd(3) + qd(4))) - 80*s6*(-c5*(-qd(3) + qd(4)) - s5*(-c3*s4*(qd(1) + qd(2)) + c4*s3*(qd(1) + qd(2)))))) + 0.00151607*qd(5)*(-c5*(-qd(3) + qd(4)) - s5*(-c3*s4*(qd(1) + qd(2)) + c4*s3*(qd(1) + qd(2)))) + 0.000409305*qd(5)*(c5*(-c3*s4*(qd(1) + qd(2)) + c4*s3*(qd(1) + qd(2))) - s5*(-qd(3) + qd(4))) - 0.00151607*s5*(-qdd(3) + qdd(4)) + 0.000409305*s5*(c4*(c3*qd(3)*(qd(1) + qd(2)) + s3*(qdd(1) + qdd(2))) + qd(4)*(-c3*c4*(qd(1) + qd(2)) - s3*s4*(qd(1) + qd(2))) - s4*(c3*(qdd(1) + qdd(2)) - qd(3)*s3*(qd(1) + qd(2)))) - s5*(-3.01352e-6*c6*(-c5*(-qdd(3) + qdd(4)) - qd(5)*(c5*(-c3*s4*(qd(1) + qd(2)) + c4*s3*(qd(1) + qd(2))) - s5*(-qd(3) + qd(4))) - s5*(c4*(c3*qd(3)*(qd(1) + qd(2)) + s3*(qdd(1) + qdd(2))) + qd(4)*(-c3*c4*(qd(1) + qd(2)) - s3*s4*(qd(1) + qd(2))) - s4*(c3*(qdd(1) + qdd(2)) - qd(3)*s3*(qd(1) + qd(2))))) - 3.01352e-6*qd(6)*(c6*(c5*(-c3*s4*(qd(1) + qd(2)) + c4*s3*(qd(1) + qd(2))) - s5*(-qd(3) + qd(4))) - s6*(-c5*(-qd(3) + qd(4)) - s5*(-c3*s4*(qd(1) + qd(2)) + c4*s3*(qd(1) + qd(2))))) - 3.01352e-6*s6*(c5*(c4*(c3*qd(3)*(qd(1) + qd(2)) + s3*(qdd(1) + qdd(2))) + qd(4)*(-c3*c4*(qd(1) + qd(2)) - s3*s4*(qd(1) + qd(2))) - s4*(c3*(qdd(1) + qdd(2)) - qd(3)*s3*(qd(1) + qd(2)))) + qd(5)*(-c5*(-qd(3) + qd(4)) - s5*(-c3*s4*(qd(1) + qd(2)) + c4*s3*(qd(1) + qd(2)))) - s5*(-qdd(3) + qdd(4))) + (6.20477e-6*c6*(c5*(-c3*s4*(qd(1) + qd(2)) + c4*s3*(qd(1) + qd(2))) - s5*(-qd(3) + qd(4))) - 6.20477e-6*s6*(-c5*(-qd(3) + qd(4)) - s5*(-c3*s4*(qd(1) + qd(2)) + c4*s3*(qd(1) + qd(2)))))*(c3*c4*(qd(1) + qd(2)) - qd(5) + qd(6) + s3*s4*(qd(1) + qd(2))) - (c6*(c5*(-c3*s4*(qd(1) + qd(2)) + c4*s3*(qd(1) + qd(2))) - s5*(-qd(3) + qd(4))) - s6*(-c5*(-qd(3) + qd(4)) - s5*(-c3*s4*(qd(1) + qd(2)) + c4*s3*(qd(1) + qd(2)))))*(3.29301e-6*c3*c4*(qd(1) + qd(2)) - 3.29301e-6*qd(5) + 3.29301e-6*qd(6) + 3.29301e-6*s3*s4*(qd(1) + qd(2)))) + (-c5*(-qd(3) + qd(4)) - s5*(-c3*s4*(qd(1) + qd(2)) + c4*s3*(qd(1) + qd(2))))*(-0.00358942*c3*c4*(qd(1) + qd(2)) + 0.00358942*qd(5) - 0.00358942*s3*s4*(qd(1) + qd(2))) - (-c3*c4*(qd(1) + qd(2)) + qd(5) - s3*s4*(qd(1) + qd(2)))*(-0.00355535*c5*(-qd(3) + qd(4)) - 0.000409305*c5*(-c3*s4*(qd(1) + qd(2)) + c4*s3*(qd(1) + qd(2))) + 0.000409305*s5*(-qd(3) + qd(4)) - 0.00355535*s5*(-c3*s4*(qd(1) + qd(2)) + c4*s3*(qd(1) + qd(2))))) + 0.00950111*qd(4)*(-c3*c4*(qd(1) + qd(2)) - s3*s4*(qd(1) + qd(2))) + 0.00163355*qd(4)*(-c3*s4*(qd(1) + qd(2)) + c4*s3*(qd(1) + qd(2))) + 8.41256e-6*qdd(3) - 8.41256e-6*qdd(4) - 0.00950111*s4*(c3*(qdd(1) + qdd(2)) - qd(3)*s3*(qd(1) + qd(2))) + 0.00163355*s4*(c3*qd(3)*(qd(1) + qd(2)) + s3*(qdd(1) + qdd(2))) - s4*(3.29301e-6*c4*(c3*(qdd(1) + qdd(2)) - qd(3)*s3*(qd(1) + qd(2))) - 295*c5*m7*(80*c6*(-c5*(-qdd(3) + qdd(4)) - qd(5)*(c5*(-c3*s4*(qd(1) + qd(2)) + c4*s3*(qd(1) + qd(2))) - s5*(-qd(3) + qd(4))) - s5*(c4*(c3*qd(3)*(qd(1) + qd(2)) + s3*(qdd(1) + qdd(2))) + qd(4)*(-c3*c4*(qd(1) + qd(2)) - s3*s4*(qd(1) + qd(2))) - s4*(c3*(qdd(1) + qdd(2)) - qd(3)*s3*(qd(1) + qd(2))))) + c6*(80*c5*(-qdd(3) + qdd(4)) + c5*(c4*(-295*c3*(qdd(1) + qdd(2)) + c3*(c2*(-g*s1 - 270*qd(1)^2) + s2*(-c1*g + 270*qdd(1)) - (qd(1) + qd(2))*(90*qd(1) + 90*qd(2)))) - s4*(295*s3*(qdd(1) + qdd(2)) - s3*(c2*(-g*s1 - 270*qd(1)^2) + s2*(-c1*g + 270*qdd(1)) - (qd(1) + qd(2))*(90*qd(1) + 90*qd(2))))) + 80*qd(5)*(c5*(-c3*s4*(qd(1) + qd(2)) + c4*s3*(qd(1) + qd(2))) - s5*(-qd(3) + qd(4))) + 80*s5*(c4*(c3*qd(3)*(qd(1) + qd(2)) + s3*(qdd(1) + qdd(2))) + qd(4)*(-c3*c4*(qd(1) + qd(2)) - s3*s4*(qd(1) + qd(2))) - s4*(c3*(qdd(1) + qdd(2)) - qd(3)*s3*(qd(1) + qd(2)))) - s5*(-c2*(-c1*g + 270*qdd(1)) - 295*c3^2*(qd(1) + qd(2)) ^2 - 90*qdd(1) - 90*qdd(2) + s2*(-g*s1 - 270*qd(1)^2) - 295*s3^2*(qd(1) + qd(2)) ^2) - (80*c5*(-c3*s4*(qd(1) + qd(2)) + c4*s3*(qd(1) + qd(2))) - 80*s5*(-qd(3) + qd(4)))*(-c3*c4*(qd(1) + qd(2)) + qd(5) - s3*s4*(qd(1) + qd(2)))) + 80*qd(6)*(c6*(c5*(-c3*s4*(qd(1) + qd(2)) + c4*s3*(qd(1) + qd(2))) - s5*(-qd(3) + qd(4))) - s6*(-c5*(-qd(3) + qd(4)) - s5*(-c3*s4*(qd(1) + qd(2)) + c4*s3*(qd(1) + qd(2))))) + 80*s6*(c5*(c4*(c3*qd(3)*(qd(1) + qd(2)) + s3*(qdd(1) + qdd(2))) + qd(4)*(-c3*c4*(qd(1) + qd(2)) - s3*s4*(qd(1) + qd(2))) - s4*(c3*(qdd(1) + qdd(2)) - qd(3)*s3*(qd(1) + qd(2)))) + qd(5)*(-c5*(-qd(3) + qd(4)) - s5*(-c3*s4*(qd(1) + qd(2)) + c4*s3*(qd(1) + qd(2)))) - s5*(-qdd(3) + qdd(4))) - s6*(80*c5*(c4*(c3*qd(3)*(qd(1) + qd(2)) + s3*(qdd(1) + qdd(2))) + qd(4)*(-c3*c4*(qd(1) + qd(2)) - s3*s4*(qd(1) + qd(2))) - s4*(c3*(qdd(1) + qdd(2)) - qd(3)*s3*(qd(1) + qd(2)))) - c5*(-c2*(-c1*g + 270*qdd(1)) - 295*c3^2*(qd(1) + qd(2)) ^2 - 90*qdd(1) - 90*qdd(2) + s2*(-g*s1 - 270*qd(1)^2) - 295*s3^2*(qd(1) + qd(2)) ^2) + 80*qd(5)*(-c5*(-qd(3) + qd(4)) - s5*(-c3*s4*(qd(1) + qd(2)) + c4*s3*(qd(1) + qd(2)))) - 80*s5*(-qdd(3) + qdd(4)) - s5*(c4*(-295*c3*(qdd(1) + qdd(2)) + c3*(c2*(-g*s1 - 270*qd(1)^2) + s2*(-c1*g + 270*qdd(1)) - (qd(1) + qd(2))*(90*qd(1) + 90*qd(2)))) - s4*(295*s3*(qdd(1) + qdd(2)) - s3*(c2*(-g*s1 - 270*qd(1)^2) + s2*(-c1*g + 270*qdd(1)) - (qd(1) + qd(2))*(90*qd(1) + 90*qd(2))))) + (80*c5*(-qd(3) + qd(4)) + 80*s5*(-c3*s4*(qd(1) + qd(2)) + c4*s3*(qd(1) + qd(2))))*(-c3*c4*(qd(1) + qd(2)) + qd(5) - s3*s4*(qd(1) + qd(2)))) - (80*c6*(c5*(-c3*s4*(qd(1) + qd(2)) + c4*s3*(qd(1) + qd(2))) - s5*(-qd(3) + qd(4))) - 80*s6*(-c5*(-qd(3) + qd(4)) - s5*(-c3*s4*(qd(1) + qd(2)) + c4*s3*(qd(1) + qd(2)))))*(c3*c4*(qd(1) + qd(2)) - qd(5) + qd(6) + s3*s4*(qd(1) + qd(2)))) - 0.00355535*c5*(-qdd(3) + qdd(4)) - 0.000409305*c5*(c4*(c3*qd(3)*(qd(1) + qd(2)) + s3*(qdd(1) + qdd(2))) + qd(4)*(-c3*c4*(qd(1) + qd(2)) - s3*s4*(qd(1) + qd(2))) - s4*(c3*(qdd(1) + qdd(2)) - qd(3)*s3*(qd(1) + qd(2)))) - 295*m6*(c5*(c4*(-295*c3*(qdd(1) + qdd(2)) + c3*(c2*(-g*s1 - 270*qd(1)^2) + s2*(-c1*g + 270*qdd(1)) - (qd(1) + qd(2))*(90*qd(1) + 90*qd(2)))) - s4*(295*s3*(qdd(1) + qdd(2)) - s3*(c2*(-g*s1 - 270*qd(1)^2) + s2*(-c1*g + 270*qdd(1)) - (qd(1) + qd(2))*(90*qd(1) + 90*qd(2))))) - s5*(-c2*(-c1*g + 270*qdd(1)) - 295*c3^2*(qd(1) + qd(2)) ^2 - 90*qdd(1) - 90*qdd(2) + s2*(-g*s1 - 270*qd(1)^2) - 295*s3^2*(qd(1) + qd(2)) ^2)) + 295*m7*s5*(80*c6*(c5*(c4*(c3*qd(3)*(qd(1) + qd(2)) + s3*(qdd(1) + qdd(2))) + qd(4)*(-c3*c4*(qd(1) + qd(2)) - s3*s4*(qd(1) + qd(2))) - s4*(c3*(qdd(1) + qdd(2)) - qd(3)*s3*(qd(1) + qd(2)))) + qd(5)*(-c5*(-qd(3) + qd(4)) - s5*(-c3*s4*(qd(1) + qd(2)) + c4*s3*(qd(1) + qd(2)))) - s5*(-qdd(3) + qdd(4))) - c6*(80*c5*(c4*(c3*qd(3)*(qd(1) + qd(2)) + s3*(qdd(1) + qdd(2))) + qd(4)*(-c3*c4*(qd(1) + qd(2)) - s3*s4*(qd(1) + qd(2))) - s4*(c3*(qdd(1) + qdd(2)) - qd(3)*s3*(qd(1) + qd(2)))) - c5*(-c2*(-c1*g + 270*qdd(1)) - 295*c3^2*(qd(1) + qd(2)) ^2 - 90*qdd(1) - 90*qdd(2) + s2*(-g*s1 - 270*qd(1)^2) - 295*s3^2*(qd(1) + qd(2)) ^2) + 80*qd(5)*(-c5*(-qd(3) + qd(4)) - s5*(-c3*s4*(qd(1) + qd(2)) + c4*s3*(qd(1) + qd(2)))) - 80*s5*(-qdd(3) + qdd(4)) - s5*(c4*(-295*c3*(qdd(1) + qdd(2)) + c3*(c2*(-g*s1 - 270*qd(1)^2) + s2*(-c1*g + 270*qdd(1)) - (qd(1) + qd(2))*(90*qd(1) + 90*qd(2)))) - s4*(295*s3*(qdd(1) + qdd(2)) - s3*(c2*(-g*s1 - 270*qd(1)^2) + s2*(-c1*g + 270*qdd(1)) - (qd(1) + qd(2))*(90*qd(1) + 90*qd(2))))) + (80*c5*(-qd(3) + qd(4)) + 80*s5*(-c3*s4*(qd(1) + qd(2)) + c4*s3*(qd(1) + qd(2))))*(-c3*c4*(qd(1) + qd(2)) + qd(5) - s3*s4*(qd(1) + qd(2)))) + 80*qd(6)*(-c6*(-c5*(-qd(3) + qd(4)) - s5*(-c3*s4*(qd(1) + qd(2)) + c4*s3*(qd(1) + qd(2)))) - s6*(c5*(-c3*s4*(qd(1) + qd(2)) + c4*s3*(qd(1) + qd(2))) - s5*(-qd(3) + qd(4)))) - 80*s6*(-c5*(-qdd(3) + qdd(4)) - qd(5)*(c5*(-c3*s4*(qd(1) + qd(2)) + c4*s3*(qd(1) + qd(2))) - s5*(-qd(3) + qd(4))) - s5*(c4*(c3*qd(3)*(qd(1) + qd(2)) + s3*(qdd(1) + qdd(2))) + qd(4)*(-c3*c4*(qd(1) + qd(2)) - s3*s4*(qd(1) + qd(2))) - s4*(c3*(qdd(1) + qdd(2)) - qd(3)*s3*(qd(1) + qd(2))))) - s6*(80*c5*(-qdd(3) + qdd(4)) + c5*(c4*(-295*c3*(qdd(1) + qdd(2)) + c3*(c2*(-g*s1 - 270*qd(1)^2) + s2*(-c1*g + 270*qdd(1)) - (qd(1) + qd(2))*(90*qd(1) + 90*qd(2)))) - s4*(295*s3*(qdd(1) + qdd(2)) - s3*(c2*(-g*s1 - 270*qd(1)^2) + s2*(-c1*g + 270*qdd(1)) - (qd(1) + qd(2))*(90*qd(1) + 90*qd(2))))) + 80*qd(5)*(c5*(-c3*s4*(qd(1) + qd(2)) + c4*s3*(qd(1) + qd(2))) - s5*(-qd(3) + qd(4))) + 80*s5*(c4*(c3*qd(3)*(qd(1) + qd(2)) + s3*(qdd(1) + qdd(2))) + qd(4)*(-c3*c4*(qd(1) + qd(2)) - s3*s4*(qd(1) + qd(2))) - s4*(c3*(qdd(1) + qdd(2)) - qd(3)*s3*(qd(1) + qd(2)))) - s5*(-c2*(-c1*g + 270*qdd(1)) - 295*c3^2*(qd(1) + qd(2)) ^2 - 90*qdd(1) - 90*qdd(2) + s2*(-g*s1 - 270*qd(1)^2) - 295*s3^2*(qd(1) + qd(2)) ^2) - (80*c5*(-c3*s4*(qd(1) + qd(2)) + c4*s3*(qd(1) + qd(2))) - 80*s5*(-qd(3) + qd(4)))*(-c3*c4*(qd(1) + qd(2)) + qd(5) - s3*s4*(qd(1) + qd(2)))) + (80*c6*(-c5*(-qd(3) + qd(4)) - s5*(-c3*s4*(qd(1) + qd(2)) + c4*s3*(qd(1) + qd(2)))) + 80*s6*(c5*(-c3*s4*(qd(1) + qd(2)) + c4*s3*(qd(1) + qd(2))) - s5*(-qd(3) + qd(4))))*(c3*c4*(qd(1) + qd(2)) - qd(5) + qd(6) + s3*s4*(qd(1) + qd(2)))) + 3.29301e-6*qd(4)*(-c3*s4*(qd(1) + qd(2)) + c4*s3*(qd(1) + qd(2))) - 0.000409305*qd(5)*(-c5*(-qd(3) + qd(4)) - s5*(-c3*s4*(qd(1) + qd(2)) + c4*s3*(qd(1) + qd(2)))) - 0.00355535*qd(5)*(c5*(-c3*s4*(qd(1) + qd(2)) + c4*s3*(qd(1) + qd(2))) - s5*(-qd(3) + qd(4))) - 3.29301e-6*qdd(5) + 3.29301e-6*qdd(6) + 3.29301e-6*s4*(c3*qd(3)*(qd(1) + qd(2)) + s3*(qdd(1) + qdd(2))) + 0.000409305*s5*(-qdd(3) + qdd(4)) - 0.00355535*s5*(c4*(c3*qd(3)*(qd(1) + qd(2)) + s3*(qdd(1) + qdd(2))) + qd(4)*(-c3*c4*(qd(1) + qd(2)) - s3*s4*(qd(1) + qd(2))) - s4*(c3*(qdd(1) + qdd(2)) - qd(3)*s3*(qd(1) + qd(2)))) - (c5*(-c3*s4*(qd(1) + qd(2)) + c4*s3*(qd(1) + qd(2))) - s5*(-qd(3) + qd(4)))*(-0.00358942*c3*c4*(qd(1) + qd(2)) + 0.00358942*qd(5) - 0.00358942*s3*s4*(qd(1) + qd(2))) - (-c6*(-c5*(-qd(3) + qd(4)) - s5*(-c3*s4*(qd(1) + qd(2)) + c4*s3*(qd(1) + qd(2)))) - s6*(c5*(-c3*s4*(qd(1) + qd(2)) + c4*s3*(qd(1) + qd(2))) - s5*(-qd(3) + qd(4))))*(6.20477e-6*c6*(c5*(-c3*s4*(qd(1) + qd(2)) + c4*s3*(qd(1) + qd(2))) - s5*(-qd(3) + qd(4))) - 6.20477e-6*s6*(-c5*(-qd(3) + qd(4)) - s5*(-c3*s4*(qd(1) + qd(2)) + c4*s3*(qd(1) + qd(2))))) + (-3.01352e-6*c6*(-c5*(-qd(3) + qd(4)) - s5*(-c3*s4*(qd(1) + qd(2)) + c4*s3*(qd(1) + qd(2)))) - 3.01352e-6*s6*(c5*(-c3*s4*(qd(1) + qd(2)) + c4*s3*(qd(1) + qd(2))) - s5*(-qd(3) + qd(4))))*(c6*(c5*(-c3*s4*(qd(1) + qd(2)) + c4*s3*(qd(1) + qd(2))) - s5*(-qd(3) + qd(4))) - s6*(-c5*(-qd(3) + qd(4)) - s5*(-c3*s4*(qd(1) + qd(2)) + c4*s3*(qd(1) + qd(2))))) + (-c3*c4*(qd(1) + qd(2)) + qd(5) - s3*s4*(qd(1) + qd(2)))*(0.000409305*c5*(-qd(3) + qd(4)) + 0.00151607*c5*(-c3*s4*(qd(1) + qd(2)) + c4*s3*(qd(1) + qd(2))) - 0.00151607*s5*(-qd(3) + qd(4)) + 0.000409305*s5*(-c3*s4*(qd(1) + qd(2)) + c4*s3*(qd(1) + qd(2))))) - (-qd(3) + qd(4))*(-0.020170031*c3*c4*(qd(1) + qd(2)) + 0.00163355*c3*s4*(qd(1) + qd(2)) - 0.00163355*c4*s3*(qd(1) + qd(2)) + 2.69102e-6*qd(3) - 2.69102e-6*qd(4) - 0.020170031*s3*s4*(qd(1) + qd(2))) + (-c3*c4*(qd(1) + qd(2)) - s3*s4*(qd(1) + qd(2)))*(2.69102e-6*c3*c4*(qd(1) + qd(2)) + 8.41256e-6*c3*s4*(qd(1) + qd(2)) - 8.41256e-6*c4*s3*(qd(1) + qd(2)) - 0.024130024*qd(3) + 0.024130024*qd(4) + 2.69102e-6*s3*s4*(qd(1) + qd(2)))));
%  
% tau2 = -0.0247925*c3*qd(3)*(qd(1) + qd(2)) - c3*(qd(1) + qd(2))*(-0.00947011*c3*(qd(1) + qd(2)) - 0.0247925*qd(3) + 0.775113*s3*(qd(1) + qd(2))) - 0.00744338*c3*(qdd(1) + qdd(2)) + c3*(-0.020170031*c4*(c3*(qdd(1) + qdd(2)) - qd(3)*s3*(qd(1) + qd(2))) - 0.00163355*c4*(c3*qd(3)*(qd(1) + qd(2)) + s3*(qdd(1) + qdd(2))) - c4*(3.29301e-6*c4*(c3*(qdd(1) + qdd(2)) - qd(3)*s3*(qd(1) + qd(2))) - 295*c5*m7*(80*c6*(-c5*(-qdd(3) + qdd(4)) - qd(5)*(c5*(-c3*s4*(qd(1) + qd(2)) + c4*s3*(qd(1) + qd(2))) - s5*(-qd(3) + qd(4))) - s5*(c4*(c3*qd(3)*(qd(1) + qd(2)) + s3*(qdd(1) + qdd(2))) + qd(4)*(-c3*c4*(qd(1) + qd(2)) - s3*s4*(qd(1) + qd(2))) - s4*(c3*(qdd(1) + qdd(2)) - qd(3)*s3*(qd(1) + qd(2))))) + c6*(80*c5*(-qdd(3) + qdd(4)) + c5*(c4*(-295*c3*(qdd(1) + qdd(2)) + c3*(c2*(-g*s1 - 270*qd(1)^2) + s2*(-c1*g + 270*qdd(1)) - (qd(1) + qd(2))*(90*qd(1) + 90*qd(2)))) - s4*(295*s3*(qdd(1) + qdd(2)) - s3*(c2*(-g*s1 - 270*qd(1)^2) + s2*(-c1*g + 270*qdd(1)) - (qd(1) + qd(2))*(90*qd(1) + 90*qd(2))))) + 80*qd(5)*(c5*(-c3*s4*(qd(1) + qd(2)) + c4*s3*(qd(1) + qd(2))) - s5*(-qd(3) + qd(4))) + 80*s5*(c4*(c3*qd(3)*(qd(1) + qd(2)) + s3*(qdd(1) + qdd(2))) + qd(4)*(-c3*c4*(qd(1) + qd(2)) - s3*s4*(qd(1) + qd(2))) - s4*(c3*(qdd(1) + qdd(2)) - qd(3)*s3*(qd(1) + qd(2)))) - s5*(-c2*(-c1*g + 270*qdd(1)) - 295*c3^2*(qd(1) + qd(2)) ^2 - 90*qdd(1) - 90*qdd(2) + s2*(-g*s1 - 270*qd(1)^2) - 295*s3^2*(qd(1) + qd(2)) ^2) - (80*c5*(-c3*s4*(qd(1) + qd(2)) + c4*s3*(qd(1) + qd(2))) - 80*s5*(-qd(3) + qd(4)))*(-c3*c4*(qd(1) + qd(2)) + qd(5) - s3*s4*(qd(1) + qd(2)))) + 80*qd(6)*(c6*(c5*(-c3*s4*(qd(1) + qd(2)) + c4*s3*(qd(1) + qd(2))) - s5*(-qd(3) + qd(4))) - s6*(-c5*(-qd(3) + qd(4)) - s5*(-c3*s4*(qd(1) + qd(2)) + c4*s3*(qd(1) + qd(2))))) + 80*s6*(c5*(c4*(c3*qd(3)*(qd(1) + qd(2)) + s3*(qdd(1) + qdd(2))) + qd(4)*(-c3*c4*(qd(1) + qd(2)) - s3*s4*(qd(1) + qd(2))) - s4*(c3*(qdd(1) + qdd(2)) - qd(3)*s3*(qd(1) + qd(2)))) + qd(5)*(-c5*(-qd(3) + qd(4)) - s5*(-c3*s4*(qd(1) + qd(2)) + c4*s3*(qd(1) + qd(2)))) - s5*(-qdd(3) + qdd(4))) - s6*(80*c5*(c4*(c3*qd(3)*(qd(1) + qd(2)) + s3*(qdd(1) + qdd(2))) + qd(4)*(-c3*c4*(qd(1) + qd(2)) - s3*s4*(qd(1) + qd(2))) - s4*(c3*(qdd(1) + qdd(2)) - qd(3)*s3*(qd(1) + qd(2)))) - c5*(-c2*(-c1*g + 270*qdd(1)) - 295*c3^2*(qd(1) + qd(2)) ^2 - 90*qdd(1) - 90*qdd(2) + s2*(-g*s1 - 270*qd(1)^2) - 295*s3^2*(qd(1) + qd(2)) ^2) + 80*qd(5)*(-c5*(-qd(3) + qd(4)) - s5*(-c3*s4*(qd(1) + qd(2)) + c4*s3*(qd(1) + qd(2)))) - 80*s5*(-qdd(3) + qdd(4)) - s5*(c4*(-295*c3*(qdd(1) + qdd(2)) + c3*(c2*(-g*s1 - 270*qd(1)^2) + s2*(-c1*g + 270*qdd(1)) - (qd(1) + qd(2))*(90*qd(1) + 90*qd(2)))) - s4*(295*s3*(qdd(1) + qdd(2)) - s3*(c2*(-g*s1 - 270*qd(1)^2) + s2*(-c1*g + 270*qdd(1)) - (qd(1) + qd(2))*(90*qd(1) + 90*qd(2))))) + (80*c5*(-qd(3) + qd(4)) + 80*s5*(-c3*s4*(qd(1) + qd(2)) + c4*s3*(qd(1) + qd(2))))*(-c3*c4*(qd(1) + qd(2)) + qd(5) - s3*s4*(qd(1) + qd(2)))) - (80*c6*(c5*(-c3*s4*(qd(1) + qd(2)) + c4*s3*(qd(1) + qd(2))) - s5*(-qd(3) + qd(4))) - 80*s6*(-c5*(-qd(3) + qd(4)) - s5*(-c3*s4*(qd(1) + qd(2)) + c4*s3*(qd(1) + qd(2)))))*(c3*c4*(qd(1) + qd(2)) - qd(5) + qd(6) + s3*s4*(qd(1) + qd(2)))) - 0.00355535*c5*(-qdd(3) + qdd(4)) - 0.000409305*c5*(c4*(c3*qd(3)*(qd(1) + qd(2)) + s3*(qdd(1) + qdd(2))) + qd(4)*(-c3*c4*(qd(1) + qd(2)) - s3*s4*(qd(1) + qd(2))) - s4*(c3*(qdd(1) + qdd(2)) - qd(3)*s3*(qd(1) + qd(2)))) - 295*m6*(c5*(c4*(-295*c3*(qdd(1) + qdd(2)) + c3*(c2*(-g*s1 - 270*qd(1)^2) + s2*(-c1*g + 270*qdd(1)) - (qd(1) + qd(2))*(90*qd(1) + 90*qd(2)))) - s4*(295*s3*(qdd(1) + qdd(2)) - s3*(c2*(-g*s1 - 270*qd(1)^2) + s2*(-c1*g + 270*qdd(1)) - (qd(1) + qd(2))*(90*qd(1) + 90*qd(2))))) - s5*(-c2*(-c1*g + 270*qdd(1)) - 295*c3^2*(qd(1) + qd(2)) ^2 - 90*qdd(1) - 90*qdd(2) + s2*(-g*s1 - 270*qd(1)^2) - 295*s3^2*(qd(1) + qd(2)^2)) + 295*m7*s5*(80*c6*(c5*(c4*(c3*qd(3)*(qd(1) + qd(2)) + s3*(qdd(1) + qdd(2))) + qd(4)*(-c3*c4*(qd(1) + qd(2)) - s3*s4*(qd(1) + qd(2))) - s4*(c3*(qdd(1) + qdd(2)) - qd(3)*s3*(qd(1) + qd(2)))) + qd(5)*(-c5*(-qd(3) + qd(4)) - s5*(-c3*s4*(qd(1) + qd(2)) + c4*s3*(qd(1) + qd(2)))) - s5*(-qdd(3) + qdd(4))) - c6*(80*c5*(c4*(c3*qd(3)*(qd(1) + qd(2)) + s3*(qdd(1) + qdd(2))) + qd(4)*(-c3*c4*(qd(1) + qd(2)) - s3*s4*(qd(1) + qd(2))) - s4*(c3*(qdd(1) + qdd(2)) - qd(3)*s3*(qd(1) + qd(2)))) - c5*(-c2*(-c1*g + 270*qdd(1)) - 295*c3^2*(qd(1) + qd(2)) ^2 - 90*qdd(1) - 90*qdd(2) + s2*(-g*s1 - 270*qd(1)^2) - 295*s3^2*(qd(1) + qd(2)) ^2) + 80*qd(5)*(-c5*(-qd(3) + qd(4)) - s5*(-c3*s4*(qd(1) + qd(2)) + c4*s3*(qd(1) + qd(2)))) - 80*s5*(-qdd(3) + qdd(4)) - s5*(c4*(-295*c3*(qdd(1) + qdd(2)) + c3*(c2*(-g*s1 - 270*qd(1)^2) + s2*(-c1*g + 270*qdd(1)) - (qd(1) + qd(2))*(90*qd(1) + 90*qd(2)))) - s4*(295*s3*(qdd(1) + qdd(2)) - s3*(c2*(-g*s1 - 270*qd(1)^2) + s2*(-c1*g + 270*qdd(1)) - (qd(1) + qd(2))*(90*qd(1) + 90*qd(2))))) + (80*c5*(-qd(3) + qd(4)) + 80*s5*(-c3*s4*(qd(1) + qd(2)) + c4*s3*(qd(1) + qd(2))))*(-c3*c4*(qd(1) + qd(2)) + qd(5) - s3*s4*(qd(1) + qd(2)))) + 80*qd(6)*(-c6*(-c5*(-qd(3) + qd(4)) - s5*(-c3*s4*(qd(1) + qd(2)) + c4*s3*(qd(1) + qd(2)))) - s6*(c5*(-c3*s4*(qd(1) + qd(2)) + c4*s3*(qd(1) + qd(2))) - s5*(-qd(3) + qd(4)))) - 80*s6*(-c5*(-qdd(3) + qdd(4)) - qd(5)*(c5*(-c3*s4*(qd(1) + qd(2)) + c4*s3*(qd(1) + qd(2))) - s5*(-qd(3) + qd(4))) - s5*(c4*(c3*qd(3)*(qd(1) + qd(2)) + s3*(qdd(1) + qdd(2))) + qd(4)*(-c3*c4*(qd(1) + qd(2)) - s3*s4*(qd(1) + qd(2))) - s4*(c3*(qdd(1) + qdd(2)) - qd(3)*s3*(qd(1) + qd(2))))) - s6*(80*c5*(-qdd(3) + qdd(4)) + c5*(c4*(-295*c3*(qdd(1) + qdd(2)) + c3*(c2*(-g*s1 - 270*qd(1)^2) + s2*(-c1*g + 270*qdd(1)) - (qd(1) + qd(2))*(90*qd(1) + 90*qd(2)))) - s4*(295*s3*(qdd(1) + qdd(2)) - s3*(c2*(-g*s1 - 270*qd(1)^2) + s2*(-c1*g + 270*qdd(1)) - (qd(1) + qd(2))*(90*qd(1) + 90*qd(2))))) + 80*qd(5)*(c5*(-c3*s4*(qd(1) + qd(2)) + c4*s3*(qd(1) + qd(2))) - s5*(-qd(3) + qd(4))) + 80*s5*(c4*(c3*qd(3)*(qd(1) + qd(2)) + s3*(qdd(1) + qdd(2))) + qd(4)*(-c3*c4*(qd(1) + qd(2)) - s3*s4*(qd(1) + qd(2))) - s4*(c3*(qdd(1) + qdd(2)) - qd(3)*s3*(qd(1) + qd(2)))) - s5*(-c2*(-c1*g + 270*qdd(1)) - 295*c3^2*(qd(1) + qd(2)) ^2 - 90*qdd(1) - 90*qdd(2) + s2*(-g*s1 - 270*qd(1)^2) - 295*s3^2*(qd(1) + qd(2)) ^2) - (80*c5*(-c3*s4*(qd(1) + qd(2)) + c4*s3*(qd(1) + qd(2))) - 80*s5*(-qd(3) + qd(4)))*(-c3*c4*(qd(1) + qd(2)) + qd(5) - s3*s4*(qd(1) + qd(2)))) + (80*c6*(-c5*(-qd(3) + qd(4)) - s5*(-c3*s4*(qd(1) + qd(2)) + c4*s3*(qd(1) + qd(2)))) + 80*s6*(c5*(-c3*s4*(qd(1) + qd(2)) + c4*s3*(qd(1) + qd(2))) - s5*(-qd(3) + qd(4))))*(c3*c4*(qd(1) + qd(2)) - qd(5) + qd(6) + s3*s4*(qd(1) + qd(2)))) + 3.29301e-6*qd(4)*(-c3*s4*(qd(1) + qd(2)) + c4*s3*(qd(1) + qd(2))) - 0.000409305*qd(5)*(-c5*(-qd(3) + qd(4)) - s5*(-c3*s4*(qd(1) + qd(2)) + c4*s3*(qd(1) + qd(2)))) - 0.00355535*qd(5)*(c5*(-c3*s4*(qd(1) + qd(2)) + c4*s3*(qd(1) + qd(2))) - s5*(-qd(3) + qd(4))) - 3.29301e-6*qdd(5) + 3.29301e-6*qdd(6) + 3.29301e-6*s4*(c3*qd(3)*(qd(1) + qd(2)) + s3*(qdd(1) + qdd(2))) + 0.000409305*s5*(-qdd(3) + qdd(4)) - 0.00355535*s5*(c4*(c3*qd(3)*(qd(1) + qd(2)) + s3*(qdd(1) + qdd(2))) + qd(4)*(-c3*c4*(qd(1) + qd(2)) - s3*s4*(qd(1) + qd(2))) - s4*(c3*(qdd(1) + qdd(2)) - qd(3)*s3*(qd(1) + qd(2)))) - (c5*(-c3*s4*(qd(1) + qd(2)) + c4*s3*(qd(1) + qd(2))) - s5*(-qd(3) + qd(4)))*(-0.00358942*c3*c4*(qd(1) + qd(2)) + 0.00358942*qd(5) - 0.00358942*s3*s4*(qd(1) + qd(2))) - (-c6*(-c5*(-qd(3) + qd(4)) - s5*(-c3*s4*(qd(1) + qd(2)) + c4*s3*(qd(1) + qd(2)))) - s6*(c5*(-c3*s4*(qd(1) + qd(2)) + c4*s3*(qd(1) + qd(2))) - s5*(-qd(3) + qd(4))))*(6.20477e-6*c6*(c5*(-c3*s4*(qd(1) + qd(2)) + c4*s3*(qd(1) + qd(2))) - s5*(-qd(3) + qd(4))) - 6.20477e-6*s6*(-c5*(-qd(3) + qd(4)) - s5*(-c3*s4*(qd(1) + qd(2)) + c4*s3*(qd(1) + qd(2))))) + (-3.01352e-6*c6*(-c5*(-qd(3) + qd(4)) - s5*(-c3*s4*(qd(1) + qd(2)) + c4*s3*(qd(1) + qd(2)))) - 3.01352e-6*s6*(c5*(-c3*s4*(qd(1) + qd(2)) + c4*s3*(qd(1) + qd(2))) - s5*(-qd(3) + qd(4))))*(c6*(c5*(-c3*s4*(qd(1) + qd(2)) + c4*s3*(qd(1) + qd(2))) - s5*(-qd(3) + qd(4))) - s6*(-c5*(-qd(3) + qd(4)) - s5*(-c3*s4*(qd(1) + qd(2)) + c4*s3*(qd(1) + qd(2))))) + (-c3*c4*(qd(1) + qd(2)) + qd(5) - s3*s4*(qd(1) + qd(2)))*(0.000409305*c5*(-qd(3) + qd(4)) + 0.00151607*c5*(-c3*s4*(qd(1) + qd(2)) + c4*s3*(qd(1) + qd(2))) - 0.00151607*s5*(-qd(3) + qd(4)) + 0.000409305*s5*(-c3*s4*(qd(1) + qd(2)) + c4*s3*(qd(1) + qd(2))))) - 90*c5*m7*(80*c6*(c5*(c4*(c3*qd(3)*(qd(1) + qd(2)) + s3*(qdd(1) + qdd(2))) + qd(4)*(-c3*c4*(qd(1) + qd(2)) - s3*s4*(qd(1) + qd(2))) - s4*(c3*(qdd(1) + qdd(2)) - qd(3)*s3*(qd(1) + qd(2)))) + qd(5)*(-c5*(-qd(3) + qd(4)) - s5*(-c3*s4*(qd(1) + qd(2)) + c4*s3*(qd(1) + qd(2)))) - s5*(-qdd(3) + qdd(4))) - c6*(80*c5*(c4*(c3*qd(3)*(qd(1) + qd(2)) + s3*(qdd(1) + qdd(2))) + qd(4)*(-c3*c4*(qd(1) + qd(2)) - s3*s4*(qd(1) + qd(2))) - s4*(c3*(qdd(1) + qdd(2)) - qd(3)*s3*(qd(1) + qd(2)))) - c5*(-c2*(-c1*g + 270*qdd(1)) - 295*c3^2*(qd(1) + qd(2)) ^2 - 90*qdd(1) - 90*qdd(2) + s2*(-g*s1 - 270*qd(1)^2) - 295*s3^2*(qd(1) + qd(2)) ^2) + 80*qd(5)*(-c5*(-qd(3) + qd(4)) - s5*(-c3*s4*(qd(1) + qd(2)) + c4*s3*(qd(1) + qd(2)))) - 80*s5*(-qdd(3) + qdd(4)) - s5*(c4*(-295*c3*(qdd(1) + qdd(2)) + c3*(c2*(-g*s1 - 270*qd(1)^2) + s2*(-c1*g + 270*qdd(1)) - (qd(1) + qd(2))*(90*qd(1) + 90*qd(2)))) - s4*(295*s3*(qdd(1) + qdd(2)) - s3*(c2*(-g*s1 - 270*qd(1)^2) + s2*(-c1*g + 270*qdd(1)) - (qd(1) + qd(2))*(90*qd(1) + 90*qd(2))))) + (80*c5*(-qd(3) + qd(4)) + 80*s5*(-c3*s4*(qd(1) + qd(2)) + c4*s3*(qd(1) + qd(2))))*(-c3*c4*(qd(1) + qd(2)) + qd(5) - s3*s4*(qd(1) + qd(2)))) + 80*qd(6)*(-c6*(-c5*(-qd(3) + qd(4)) - s5*(-c3*s4*(qd(1) + qd(2)) + c4*s3*(qd(1) + qd(2)))) - s6*(c5*(-c3*s4*(qd(1) + qd(2)) + c4*s3*(qd(1) + qd(2))) - s5*(-qd(3) + qd(4)))) - 80*s6*(-c5*(-qdd(3) + qdd(4)) - qd(5)*(c5*(-c3*s4*(qd(1) + qd(2)) + c4*s3*(qd(1) + qd(2))) - s5*(-qd(3) + qd(4))) - s5*(c4*(c3*qd(3)*(qd(1) + qd(2)) + s3*(qdd(1) + qdd(2))) + qd(4)*(-c3*c4*(qd(1) + qd(2)) - s3*s4*(qd(1) + qd(2))) - s4*(c3*(qdd(1) + qdd(2)) - qd(3)*s3*(qd(1) + qd(2))))) - s6*(80*c5*(-qdd(3) + qdd(4)) + c5*(c4*(-295*c3*(qdd(1) + qdd(2)) + c3*(c2*(-g*s1 - 270*qd(1)^2) + s2*(-c1*g + 270*qdd(1)) - (qd(1) + qd(2))*(90*qd(1) + 90*qd(2)))) - s4*(295*s3*(qdd(1) + qdd(2)) - s3*(c2*(-g*s1 - 270*qd(1)^2) + s2*(-c1*g + 270*qdd(1)) - (qd(1) + qd(2))*(90*qd(1) + 90*qd(2))))) + 80*qd(5)*(c5*(-c3*s4*(qd(1) + qd(2)) + c4*s3*(qd(1) + qd(2))) - s5*(-qd(3) + qd(4))) + 80*s5*(c4*(c3*qd(3)*(qd(1) + qd(2)) + s3*(qdd(1) + qdd(2))) + qd(4)*(-c3*c4*(qd(1) + qd(2)) - s3*s4*(qd(1) + qd(2))) - s4*(c3*(qdd(1) + qdd(2)) - qd(3)*s3*(qd(1) + qd(2)))) - s5*(-c2*(-c1*g + 270*qdd(1)) - 295*c3^2*(qd(1) + qd(2)) ^2 - 90*qdd(1) - 90*qdd(2) + s2*(-g*s1 - 270*qd(1)^2) - 295*s3^2*(qd(1) + qd(2)) ^2) - (80*c5*(-c3*s4*(qd(1) + qd(2)) + c4*s3*(qd(1) + qd(2))) - 80*s5*(-qd(3) + qd(4)))*(-c3*c4*(qd(1) + qd(2)) + qd(5) - s3*s4*(qd(1) + qd(2)))) + (80*c6*(-c5*(-qd(3) + qd(4)) - s5*(-c3*s4*(qd(1) + qd(2)) + c4*s3*(qd(1) + qd(2)))) + 80*s6*(c5*(-c3*s4*(qd(1) + qd(2)) + c4*s3*(qd(1) + qd(2))) - s5*(-qd(3) + qd(4))))*(c3*c4*(qd(1) + qd(2)) - qd(5) + qd(6) + s3*s4*(qd(1) + qd(2)))) - 90*m5*(-c2*(-c1*g + 270*qdd(1)) - 295*c3^2*(qd(1) + qd(2)) ^2 - 90*qdd(1) - 90*qdd(2) + s2*(-g*s1 - 270*qd(1)^2) - 295*s3^2*(qd(1) + qd(2)) ^2 - (-c3*c4*(qd(1) + qd(2)) - s3*s4*(qd(1) + qd(2)))*(295*c3*c4*(qd(1) + qd(2)) + 295*s3*s4*(qd(1) + qd(2))) + (-295*c3*s4*(qd(1) + qd(2)) + 295*c4*s3*(qd(1) + qd(2)))*(-c3*s4*(qd(1) + qd(2)) + c4*s3*(qd(1) + qd(2)))) + 90*m6*(-c4*(295*s3*(qdd(1) + qdd(2)) - s3*(c2*(-g*s1 - 270*qd(1)^2) + s2*(-c1*g + 270*qdd(1)) - (qd(1) + qd(2))*(90*qd(1) + 90*qd(2)))) - s4*(-295*c3*(qdd(1) + qdd(2)) + c3*(c2*(-g*s1 - 270*qd(1)^2) + s2*(-c1*g + 270*qdd(1)) - (qd(1) + qd(2))*(90*qd(1) + 90*qd(2))))) - 90*m7*s5*(80*c6*(-c5*(-qdd(3) + qdd(4)) - qd(5)*(c5*(-c3*s4*(qd(1) + qd(2)) + c4*s3*(qd(1) + qd(2))) - s5*(-qd(3) + qd(4))) - s5*(c4*(c3*qd(3)*(qd(1) + qd(2)) + s3*(qdd(1) + qdd(2))) + qd(4)*(-c3*c4*(qd(1) + qd(2)) - s3*s4*(qd(1) + qd(2))) - s4*(c3*(qdd(1) + qdd(2)) - qd(3)*s3*(qd(1) + qd(2))))) + c6*(80*c5*(-qdd(3) + qdd(4)) + c5*(c4*(-295*c3*(qdd(1) + qdd(2)) + c3*(c2*(-g*s1 - 270*qd(1)^2) + s2*(-c1*g + 270*qdd(1)) - (qd(1) + qd(2))*(90*qd(1) + 90*qd(2)))) - s4*(295*s3*(qdd(1) + qdd(2)) - s3*(c2*(-g*s1 - 270*qd(1)^2) + s2*(-c1*g + 270*qdd(1)) - (qd(1) + qd(2))*(90*qd(1) + 90*qd(2))))) + 80*qd(5)*(c5*(-c3*s4*(qd(1) + qd(2)) + c4*s3*(qd(1) + qd(2))) - s5*(-qd(3) + qd(4))) + 80*s5*(c4*(c3*qd(3)*(qd(1) + qd(2)) + s3*(qdd(1) + qdd(2))) + qd(4)*(-c3*c4*(qd(1) + qd(2)) - s3*s4*(qd(1) + qd(2))) - s4*(c3*(qdd(1) + qdd(2)) - qd(3)*s3*(qd(1) + qd(2)))) - s5*(-c2*(-c1*g + 270*qdd(1)) - 295*c3^2*(qd(1) + qd(2)) ^2 - 90*qdd(1) - 90*qdd(2) + s2*(-g*s1 - 270*qd(1)^2) - 295*s3^2*(qd(1) + qd(2)) ^2) - (80*c5*(-c3*s4*(qd(1) + qd(2)) + c4*s3*(qd(1) + qd(2))) - 80*s5*(-qd(3) + qd(4)))*(-c3*c4*(qd(1) + qd(2)) + qd(5) - s3*s4*(qd(1) + qd(2)))) + 80*qd(6)*(c6*(c5*(-c3*s4*(qd(1) + qd(2)) + c4*s3*(qd(1) + qd(2))) - s5*(-qd(3) + qd(4))) - s6*(-c5*(-qd(3) + qd(4)) - s5*(-c3*s4*(qd(1) + qd(2)) + c4*s3*(qd(1) + qd(2))))) + 80*s6*(c5*(c4*(c3*qd(3)*(qd(1) + qd(2)) + s3*(qdd(1) + qdd(2))) + qd(4)*(-c3*c4*(qd(1) + qd(2)) - s3*s4*(qd(1) + qd(2))) - s4*(c3*(qdd(1) + qdd(2)) - qd(3)*s3*(qd(1) + qd(2)))) + qd(5)*(-c5*(-qd(3) + qd(4)) - s5*(-c3*s4*(qd(1) + qd(2)) + c4*s3*(qd(1) + qd(2)))) - s5*(-qdd(3) + qdd(4))) - s6*(80*c5*(c4*(c3*qd(3)*(qd(1) + qd(2)) + s3*(qdd(1) + qdd(2))) + qd(4)*(-c3*c4*(qd(1) + qd(2)) - s3*s4*(qd(1) + qd(2))) - s4*(c3*(qdd(1) + qdd(2)) - qd(3)*s3*(qd(1) + qd(2)))) - c5*(-c2*(-c1*g + 270*qdd(1)) - 295*c3^2*(qd(1) + qd(2)) ^2 - 90*qdd(1) - 90*qdd(2) + s2*(-g*s1 - 270*qd(1)^2) - 295*s3^2*(qd(1) + qd(2)) ^2) + 80*qd(5)*(-c5*(-qd(3) + qd(4)) - s5*(-c3*s4*(qd(1) + qd(2)) + c4*s3*(qd(1) + qd(2)))) - 80*s5*(-qdd(3) + qdd(4)) - s5*(c4*(-295*c3*(qdd(1) + qdd(2)) + c3*(c2*(-g*s1 - 270*qd(1)^2) + s2*(-c1*g + 270*qdd(1)) - (qd(1) + qd(2))*(90*qd(1) + 90*qd(2)))) - s4*(295*s3*(qdd(1) + qdd(2)) - s3*(c2*(-g*s1 - 270*qd(1)^2) + s2*(-c1*g + 270*qdd(1)) - (qd(1) + qd(2))*(90*qd(1) + 90*qd(2))))) + (80*c5*(-qd(3) + qd(4)) + 80*s5*(-c3*s4*(qd(1) + qd(2)) + c4*s3*(qd(1) + qd(2))))*(-c3*c4*(qd(1) + qd(2)) + qd(5) - s3*s4*(qd(1) + qd(2)))) - (80*c6*(c5*(-c3*s4*(qd(1) + qd(2)) + c4*s3*(qd(1) + qd(2))) - s5*(-qd(3) + qd(4))) - 80*s6*(-c5*(-qd(3) + qd(4)) - s5*(-c3*s4*(qd(1) + qd(2)) + c4*s3*(qd(1) + qd(2)))))*(c3*c4*(qd(1) + qd(2)) - qd(5) + qd(6) + s3*s4*(qd(1) + qd(2)))) - 0.00163355*qd(4)*(-c3*c4*(qd(1) + qd(2)) - s3*s4*(qd(1) + qd(2))) - 0.020170031*qd(4)*(-c3*s4*(qd(1) + qd(2)) + c4*s3*(qd(1) + qd(2))) + 2.69102e-6*qdd(3) - 2.69102e-6*qdd(4) + 0.00163355*s4*(c3*(qdd(1) + qdd(2)) - qd(3)*s3*(qd(1) + qd(2))) - 0.020170031*s4*(c3*qd(3)*(qd(1) + qd(2)) + s3*(qdd(1) + qdd(2))) - s4*(0.000409305*c5*(-qdd(3) + qdd(4)) + 0.00151607*c5*(c4*(c3*qd(3)*(qd(1) + qd(2)) + s3*(qdd(1) + qdd(2))) + qd(4)*(-c3*c4*(qd(1) + qd(2)) - s3*s4*(qd(1) + qd(2))) - s4*(c3*(qdd(1) + qdd(2)) - qd(3)*s3*(qd(1) + qd(2)))) + c5*(6.20477e-6*c6*(c5*(c4*(c3*qd(3)*(qd(1) + qd(2)) + s3*(qdd(1) + qdd(2))) + qd(4)*(-c3*c4*(qd(1) + qd(2)) - s3*s4*(qd(1) + qd(2))) - s4*(c3*(qdd(1) + qdd(2)) - qd(3)*s3*(qd(1) + qd(2)))) + qd(5)*(-c5*(-qd(3) + qd(4)) - s5*(-c3*s4*(qd(1) + qd(2)) + c4*s3*(qd(1) + qd(2)))) - s5*(-qdd(3) + qdd(4))) + 6.20477e-6*qd(6)*(-c6*(-c5*(-qd(3) + qd(4)) - s5*(-c3*s4*(qd(1) + qd(2)) + c4*s3*(qd(1) + qd(2)))) - s6*(c5*(-c3*s4*(qd(1) + qd(2)) + c4*s3*(qd(1) + qd(2))) - s5*(-qd(3) + qd(4)))) - 6.20477e-6*s6*(-c5*(-qdd(3) + qdd(4)) - qd(5)*(c5*(-c3*s4*(qd(1) + qd(2)) + c4*s3*(qd(1) + qd(2))) - s5*(-qd(3) + qd(4))) - s5*(c4*(c3*qd(3)*(qd(1) + qd(2)) + s3*(qdd(1) + qdd(2))) + qd(4)*(-c3*c4*(qd(1) + qd(2)) - s3*s4*(qd(1) + qd(2))) - s4*(c3*(qdd(1) + qdd(2)) - qd(3)*s3*(qd(1) + qd(2))))) + (-c6*(-c5*(-qd(3) + qd(4)) - s5*(-c3*s4*(qd(1) + qd(2)) + c4*s3*(qd(1) + qd(2)))) - s6*(c5*(-c3*s4*(qd(1) + qd(2)) + c4*s3*(qd(1) + qd(2))) - s5*(-qd(3) + qd(4))))*(3.29301e-6*c3*c4*(qd(1) + qd(2)) - 3.29301e-6*qd(5) + 3.29301e-6*qd(6) + 3.29301e-6*s3*s4*(qd(1) + qd(2))) - (-3.01352e-6*c6*(-c5*(-qd(3) + qd(4)) - s5*(-c3*s4*(qd(1) + qd(2)) + c4*s3*(qd(1) + qd(2)))) - 3.01352e-6*s6*(c5*(-c3*s4*(qd(1) + qd(2)) + c4*s3*(qd(1) + qd(2))) - s5*(-qd(3) + qd(4))))*(c3*c4*(qd(1) + qd(2)) - qd(5) + qd(6) + s3*s4*(qd(1) + qd(2)))) + 295*m6*(-c5*(-c2*(-c1*g + 270*qdd(1)) - 295*c3^2*(qd(1) + qd(2)) ^2 - 90*qdd(1) - 90*qdd(2) + s2*(-g*s1 - 270*qd(1)^2) - 295*s3^2*(qd(1) + qd(2)) ^2) - s5*(c4*(-295*c3*(qdd(1) + qdd(2)) + c3*(c2*(-g*s1 - 270*qd(1)^2) + s2*(-c1*g + 270*qdd(1)) - (qd(1) + qd(2))*(90*qd(1) + 90*qd(2)))) - s4*(295*s3*(qdd(1) + qdd(2)) - s3*(c2*(-g*s1 - 270*qd(1)^2) + s2*(-c1*g + 270*qdd(1)) - (qd(1) + qd(2))*(90*qd(1) + 90*qd(2)))))) + 295*m7*(c4*(295*s3*(qdd(1) + qdd(2)) - s3*(c2*(-g*s1 - 270*qd(1)^2) + s2*(-c1*g + 270*qdd(1)) - (qd(1) + qd(2))*(90*qd(1) + 90*qd(2)))) + s4*(-295*c3*(qdd(1) + qdd(2)) + c3*(c2*(-g*s1 - 270*qd(1)^2) + s2*(-c1*g + 270*qdd(1)) - (qd(1) + qd(2))*(90*qd(1) + 90*qd(2)))) + (-c5*(-qd(3) + qd(4)) - s5*(-c3*s4*(qd(1) + qd(2)) + c4*s3*(qd(1) + qd(2))))*(80*c5*(-qd(3) + qd(4)) + 80*s5*(-c3*s4*(qd(1) + qd(2)) + c4*s3*(qd(1) + qd(2)))) - (c5*(-c3*s4*(qd(1) + qd(2)) + c4*s3*(qd(1) + qd(2))) - s5*(-qd(3) + qd(4)))*(80*c5*(-c3*s4*(qd(1) + qd(2)) + c4*s3*(qd(1) + qd(2))) - 80*s5*(-qd(3) + qd(4))) - (-c6*(-c5*(-qd(3) + qd(4)) - s5*(-c3*s4*(qd(1) + qd(2)) + c4*s3*(qd(1) + qd(2)))) - s6*(c5*(-c3*s4*(qd(1) + qd(2)) + c4*s3*(qd(1) + qd(2))) - s5*(-qd(3) + qd(4))))*(80*c6*(-c5*(-qd(3) + qd(4)) - s5*(-c3*s4*(qd(1) + qd(2)) + c4*s3*(qd(1) + qd(2)))) + 80*s6*(c5*(-c3*s4*(qd(1) + qd(2)) + c4*s3*(qd(1) + qd(2))) - s5*(-qd(3) + qd(4)))) + (c6*(c5*(-c3*s4*(qd(1) + qd(2)) + c4*s3*(qd(1) + qd(2))) - s5*(-qd(3) + qd(4))) - s6*(-c5*(-qd(3) + qd(4)) - s5*(-c3*s4*(qd(1) + qd(2)) + c4*s3*(qd(1) + qd(2)))))*(80*c6*(c5*(-c3*s4*(qd(1) + qd(2)) + c4*s3*(qd(1) + qd(2))) - s5*(-qd(3) + qd(4))) - 80*s6*(-c5*(-qd(3) + qd(4)) - s5*(-c3*s4*(qd(1) + qd(2)) + c4*s3*(qd(1) + qd(2)))))) + 0.00151607*qd(5)*(-c5*(-qd(3) + qd(4)) - s5*(-c3*s4*(qd(1) + qd(2)) + c4*s3*(qd(1) + qd(2)))) + 0.000409305*qd(5)*(c5*(-c3*s4*(qd(1) + qd(2)) + c4*s3*(qd(1) + qd(2))) - s5*(-qd(3) + qd(4))) - 0.00151607*s5*(-qdd(3) + qdd(4)) + 0.000409305*s5*(c4*(c3*qd(3)*(qd(1) + qd(2)) + s3*(qdd(1) + qdd(2))) + qd(4)*(-c3*c4*(qd(1) + qd(2)) - s3*s4*(qd(1) + qd(2))) - s4*(c3*(qdd(1) + qdd(2)) - qd(3)*s3*(qd(1) + qd(2)))) - s5*(-3.01352e-6*c6*(-c5*(-qdd(3) + qdd(4)) - qd(5)*(c5*(-c3*s4*(qd(1) + qd(2)) + c4*s3*(qd(1) + qd(2))) - s5*(-qd(3) + qd(4))) - s5*(c4*(c3*qd(3)*(qd(1) + qd(2)) + s3*(qdd(1) + qdd(2))) + qd(4)*(-c3*c4*(qd(1) + qd(2)) - s3*s4*(qd(1) + qd(2))) - s4*(c3*(qdd(1) + qdd(2)) - qd(3)*s3*(qd(1) + qd(2))))) - 3.01352e-6*qd(6)*(c6*(c5*(-c3*s4*(qd(1) + qd(2)) + c4*s3*(qd(1) + qd(2))) - s5*(-qd(3) + qd(4))) - s6*(-c5*(-qd(3) + qd(4)) - s5*(-c3*s4*(qd(1) + qd(2)) + c4*s3*(qd(1) + qd(2))))) - 3.01352e-6*s6*(c5*(c4*(c3*qd(3)*(qd(1) + qd(2)) + s3*(qdd(1) + qdd(2))) + qd(4)*(-c3*c4*(qd(1) + qd(2)) - s3*s4*(qd(1) + qd(2))) - s4*(c3*(qdd(1) + qdd(2)) - qd(3)*s3*(qd(1) + qd(2)))) + qd(5)*(-c5*(-qd(3) + qd(4)) - s5*(-c3*s4*(qd(1) + qd(2)) + c4*s3*(qd(1) + qd(2)))) - s5*(-qdd(3) + qdd(4))) + (6.20477e-6*c6*(c5*(-c3*s4*(qd(1) + qd(2)) + c4*s3*(qd(1) + qd(2))) - s5*(-qd(3) + qd(4))) - 6.20477e-6*s6*(-c5*(-qd(3) + qd(4)) - s5*(-c3*s4*(qd(1) + qd(2)) + c4*s3*(qd(1) + qd(2)))))*(c3*c4*(qd(1) + qd(2)) - qd(5) + qd(6) + s3*s4*(qd(1) + qd(2))) - (c6*(c5*(-c3*s4*(qd(1) + qd(2)) + c4*s3*(qd(1) + qd(2))) - s5*(-qd(3) + qd(4))) - s6*(-c5*(-qd(3) + qd(4)) - s5*(-c3*s4*(qd(1) + qd(2)) + c4*s3*(qd(1) + qd(2)))))*(3.29301e-6*c3*c4*(qd(1) + qd(2)) - 3.29301e-6*qd(5) + 3.29301e-6*qd(6) + 3.29301e-6*s3*s4*(qd(1) + qd(2)))) + (-c5*(-qd(3) + qd(4)) - s5*(-c3*s4*(qd(1) + qd(2)) + c4*s3*(qd(1) + qd(2))))*(-0.00358942*c3*c4*(qd(1) + qd(2)) + 0.00358942*qd(5) - 0.00358942*s3*s4*(qd(1) + qd(2))) - (-c3*c4*(qd(1) + qd(2)) + qd(5) - s3*s4*(qd(1) + qd(2)))*(-0.00355535*c5*(-qd(3) + qd(4)) - 0.000409305*c5*(-c3*s4*(qd(1) + qd(2)) + c4*s3*(qd(1) + qd(2))) + 0.000409305*s5*(-qd(3) + qd(4)) - 0.00355535*s5*(-c3*s4*(qd(1) + qd(2)) + c4*s3*(qd(1) + qd(2))))) + (-qd(3) + qd(4))*(0.00163355*c3*c4*(qd(1) + qd(2)) - 0.00950111*c3*s4*(qd(1) + qd(2)) + 0.00950111*c4*s3*(qd(1) + qd(2)) + 8.41256e-6*qd(3) - 8.41256e-6*qd(4) + 0.00163355*s3*s4*(qd(1) + qd(2))) - (-c3*s4*(qd(1) + qd(2)) + c4*s3*(qd(1) + qd(2)))*(2.69102e-6*c3*c4*(qd(1) + qd(2)) + 8.41256e-6*c3*s4*(qd(1) + qd(2)) - 8.41256e-6*c4*s3*(qd(1) + qd(2)) - 0.024130024*qd(3) + 0.024130024*qd(4) + 2.69102e-6*s3*s4*(qd(1) + qd(2)))) + 270*c5*m7*(80*c6*(c5*(c4*(c3*qd(3)*(qd(1) + qd(2)) + s3*(qdd(1) + qdd(2))) + qd(4)*(-c3*c4*(qd(1) + qd(2)) - s3*s4*(qd(1) + qd(2))) - s4*(c3*(qdd(1) + qdd(2)) - qd(3)*s3*(qd(1) + qd(2)))) + qd(5)*(-c5*(-qd(3) + qd(4)) - s5*(-c3*s4*(qd(1) + qd(2)) + c4*s3*(qd(1) + qd(2)))) - s5*(-qdd(3) + qdd(4))) - c6*(80*c5*(c4*(c3*qd(3)*(qd(1) + qd(2)) + s3*(qdd(1) + qdd(2))) + qd(4)*(-c3*c4*(qd(1) + qd(2)) - s3*s4*(qd(1) + qd(2))) - s4*(c3*(qdd(1) + qdd(2)) - qd(3)*s3*(qd(1) + qd(2)))) - c5*(-c2*(-c1*g + 270*qdd(1)) - 295*c3^2*(qd(1) + qd(2)) ^2 - 90*qdd(1) - 90*qdd(2) + s2*(-g*s1 - 270*qd(1)^2) - 295*s3^2*(qd(1) + qd(2)) ^2) + 80*qd(5)*(-c5*(-qd(3) + qd(4)) - s5*(-c3*s4*(qd(1) + qd(2)) + c4*s3*(qd(1) + qd(2)))) - 80*s5*(-qdd(3) + qdd(4)) - s5*(c4*(-295*c3*(qdd(1) + qdd(2)) + c3*(c2*(-g*s1 - 270*qd(1)^2) + s2*(-c1*g + 270*qdd(1)) - (qd(1) + qd(2))*(90*qd(1) + 90*qd(2)))) - s4*(295*s3*(qdd(1) + qdd(2)) - s3*(c2*(-g*s1 - 270*qd(1)^2) + s2*(-c1*g + 270*qdd(1)) - (qd(1) + qd(2))*(90*qd(1) + 90*qd(2))))) + (80*c5*(-qd(3) + qd(4)) + 80*s5*(-c3*s4*(qd(1) + qd(2)) + c4*s3*(qd(1) + qd(2))))*(-c3*c4*(qd(1) + qd(2)) + qd(5) - s3*s4*(qd(1) + qd(2)))) + 80*qd(6)*(-c6*(-c5*(-qd(3) + qd(4)) - s5*(-c3*s4*(qd(1) + qd(2)) + c4*s3*(qd(1) + qd(2)))) - s6*(c5*(-c3*s4*(qd(1) + qd(2)) + c4*s3*(qd(1) + qd(2))) - s5*(-qd(3) + qd(4)))) - 80*s6*(-c5*(-qdd(3) + qdd(4)) - qd(5)*(c5*(-c3*s4*(qd(1) + qd(2)) + c4*s3*(qd(1) + qd(2))) - s5*(-qd(3) + qd(4))) - s5*(c4*(c3*qd(3)*(qd(1) + qd(2)) + s3*(qdd(1) + qdd(2))) + qd(4)*(-c3*c4*(qd(1) + qd(2)) - s3*s4*(qd(1) + qd(2))) - s4*(c3*(qdd(1) + qdd(2)) - qd(3)*s3*(qd(1) + qd(2))))) - s6*(80*c5*(-qdd(3) + qdd(4)) + c5*(c4*(-295*c3*(qdd(1) + qdd(2)) + c3*(c2*(-g*s1 - 270*qd(1)^2) + s2*(-c1*g + 270*qdd(1)) - (qd(1) + qd(2))*(90*qd(1) + 90*qd(2)))) - s4*(295*s3*(qdd(1) + qdd(2)) - s3*(c2*(-g*s1 - 270*qd(1)^2) + s2*(-c1*g + 270*qdd(1)) - (qd(1) + qd(2))*(90*qd(1) + 90*qd(2))))) + 80*qd(5)*(c5*(-c3*s4*(qd(1) + qd(2)) + c4*s3*(qd(1) + qd(2))) - s5*(-qd(3) + qd(4))) + 80*s5*(c4*(c3*qd(3)*(qd(1) + qd(2)) + s3*(qdd(1) + qdd(2))) + qd(4)*(-c3*c4*(qd(1) + qd(2)) - s3*s4*(qd(1) + qd(2))) - s4*(c3*(qdd(1) + qdd(2)) - qd(3)*s3*(qd(1) + qd(2)))) - s5*(-c2*(-c1*g + 270*qdd(1)) - 295*c3^2*(qd(1) + qd(2)) ^2 - 90*qdd(1) - 90*qdd(2) + s2*(-g*s1 - 270*qd(1)^2) - 295*s3^2*(qd(1) + qd(2)) ^2) - (80*c5*(-c3*s4*(qd(1) + qd(2)) + c4*s3*(qd(1) + qd(2))) - 80*s5*(-qd(3) + qd(4)))*(-c3*c4*(qd(1) + qd(2)) + qd(5) - s3*s4*(qd(1) + qd(2)))) + (80*c6*(-c5*(-qd(3) + qd(4)) - s5*(-c3*s4*(qd(1) + qd(2)) + c4*s3*(qd(1) + qd(2)))) + 80*s6*(c5*(-c3*s4*(qd(1) + qd(2)) + c4*s3*(qd(1) + qd(2))) - s5*(-qd(3) + qd(4))))*(c3*c4*(qd(1) + qd(2)) - qd(5) + qd(6) + s3*s4*(qd(1) + qd(2)))) + 270*m4*(90*c3*s3*(qd(1) + qd(2)) ^2 + 90*qdd(3) - s3*(c2*(-g*s1 - 270*qd(1)^2) + s2*(-c1*g + 270*qdd(1)) - (qd(1) + qd(2))*(90*qd(1) + 90*qd(2)))) + 270*m5*(-c2*(-c1*g + 270*qdd(1)) - 295*c3^2*(qd(1) + qd(2)) ^2 - 90*qdd(1) - 90*qdd(2) + s2*(-g*s1 - 270*qd(1)^2) - 295*s3^2*(qd(1) + qd(2)) ^2 - (-c3*c4*(qd(1) + qd(2)) - s3*s4*(qd(1) + qd(2)))*(295*c3*c4*(qd(1) + qd(2)) + 295*s3*s4*(qd(1) + qd(2))) + (-295*c3*s4*(qd(1) + qd(2)) + 295*c4*s3*(qd(1) + qd(2)))*(-c3*s4*(qd(1) + qd(2)) + c4*s3*(qd(1) + qd(2)))) - 270*m6*(-c4*(295*s3*(qdd(1) + qdd(2)) - s3*(c2*(-g*s1 - 270*qd(1)^2) + s2*(-c1*g + 270*qdd(1)) - (qd(1) + qd(2))*(90*qd(1) + 90*qd(2)))) - s4*(-295*c3*(qdd(1) + qdd(2)) + c3*(c2*(-g*s1 - 270*qd(1)^2) + s2*(-c1*g + 270*qdd(1)) - (qd(1) + qd(2))*(90*qd(1) + 90*qd(2))))) + 270*m7*s5*(80*c6*(-c5*(-qdd(3) + qdd(4)) - qd(5)*(c5*(-c3*s4*(qd(1) + qd(2)) + c4*s3*(qd(1) + qd(2))) - s5*(-qd(3) + qd(4))) - s5*(c4*(c3*qd(3)*(qd(1) + qd(2)) + s3*(qdd(1) + qdd(2))) + qd(4)*(-c3*c4*(qd(1) + qd(2)) - s3*s4*(qd(1) + qd(2))) - s4*(c3*(qdd(1) + qdd(2)) - qd(3)*s3*(qd(1) + qd(2))))) + c6*(80*c5*(-qdd(3) + qdd(4)) + c5*(c4*(-295*c3*(qdd(1) + qdd(2)) + c3*(c2*(-g*s1 - 270*qd(1)^2) + s2*(-c1*g + 270*qdd(1)) - (qd(1) + qd(2))*(90*qd(1) + 90*qd(2)))) - s4*(295*s3*(qdd(1) + qdd(2)) - s3*(c2*(-g*s1 - 270*qd(1)^2) + s2*(-c1*g + 270*qdd(1)) - (qd(1) + qd(2))*(90*qd(1) + 90*qd(2))))) + 80*qd(5)*(c5*(-c3*s4*(qd(1) + qd(2)) + c4*s3*(qd(1) + qd(2))) - s5*(-qd(3) + qd(4))) + 80*s5*(c4*(c3*qd(3)*(qd(1) + qd(2)) + s3*(qdd(1) + qdd(2))) + qd(4)*(-c3*c4*(qd(1) + qd(2)) - s3*s4*(qd(1) + qd(2))) - s4*(c3*(qdd(1) + qdd(2)) - qd(3)*s3*(qd(1) + qd(2)))) - s5*(-c2*(-c1*g + 270*qdd(1)) - 295*c3^2*(qd(1) + qd(2)) ^2 - 90*qdd(1) - 90*qdd(2) + s2*(-g*s1 - 270*qd(1)^2) - 295*s3^2*(qd(1) + qd(2)) ^2) - (80*c5*(-c3*s4*(qd(1) + qd(2)) + c4*s3*(qd(1) + qd(2))) - 80*s5*(-qd(3) + qd(4)))*(-c3*c4*(qd(1) + qd(2)) + qd(5) - s3*s4*(qd(1) + qd(2)))) + 80*qd(6)*(c6*(c5*(-c3*s4*(qd(1) + qd(2)) + c4*s3*(qd(1) + qd(2))) - s5*(-qd(3) + qd(4))) - s6*(-c5*(-qd(3) + qd(4)) - s5*(-c3*s4*(qd(1) + qd(2)) + c4*s3*(qd(1) + qd(2))))) + 80*s6*(c5*(c4*(c3*qd(3)*(qd(1) + qd(2)) + s3*(qdd(1) + qdd(2))) + qd(4)*(-c3*c4*(qd(1) + qd(2)) - s3*s4*(qd(1) + qd(2))) - s4*(c3*(qdd(1) + qdd(2)) - qd(3)*s3*(qd(1) + qd(2)))) + qd(5)*(-c5*(-qd(3) + qd(4)) - s5*(-c3*s4*(qd(1) + qd(2)) + c4*s3*(qd(1) + qd(2)))) - s5*(-qdd(3) + qdd(4))) - s6*(80*c5*(c4*(c3*qd(3)*(qd(1) + qd(2)) + s3*(qdd(1) + qdd(2))) + qd(4)*(-c3*c4*(qd(1) + qd(2)) - s3*s4*(qd(1) + qd(2))) - s4*(c3*(qdd(1) + qdd(2)) - qd(3)*s3*(qd(1) + qd(2)))) - c5*(-c2*(-c1*g + 270*qdd(1)) - 295*c3^2*(qd(1) + qd(2)) ^2 - 90*qdd(1) - 90*qdd(2) + s2*(-g*s1 - 270*qd(1)^2) - 295*s3^2*(qd(1) + qd(2)) ^2) + 80*qd(5)*(-c5*(-qd(3) + qd(4)) - s5*(-c3*s4*(qd(1) + qd(2)) + c4*s3*(qd(1) + qd(2)))) - 80*s5*(-qdd(3) + qdd(4)) - s5*(c4*(-295*c3*(qdd(1) + qdd(2)) + c3*(c2*(-g*s1 - 270*qd(1)^2) + s2*(-c1*g + 270*qdd(1)) - (qd(1) + qd(2))*(90*qd(1) + 90*qd(2)))) - s4*(295*s3*(qdd(1) + qdd(2)) - s3*(c2*(-g*s1 - 270*qd(1)^2) + s2*(-c1*g + 270*qdd(1)) - (qd(1) + qd(2))*(90*qd(1) + 90*qd(2))))) + (80*c5*(-qd(3) + qd(4)) + 80*s5*(-c3*s4*(qd(1) + qd(2)) + c4*s3*(qd(1) + qd(2))))*(-c3*c4*(qd(1) + qd(2)) + qd(5) - s3*s4*(qd(1) + qd(2)))) - (80*c6*(c5*(-c3*s4*(qd(1) + qd(2)) + c4*s3*(qd(1) + qd(2))) - s5*(-qd(3) + qd(4))) - 80*s6*(-c5*(-qd(3) + qd(4)) - s5*(-c3*s4*(qd(1) + qd(2)) + c4*s3*(qd(1) + qd(2)))))*(c3*c4*(qd(1) + qd(2)) - qd(5) + qd(6) + s3*s4*(qd(1) + qd(2)))) + 0.00744338*qd(3)*s3*(qd(1) + qd(2)) + 0.207558*qdd(3) + s3*(qd(1) + qd(2))*(0.750399*c3*(qd(1) + qd(2)) - 0.00744338*qd(3) - 0.00947011*s3*(qd(1) + qd(2))) - 0.0247925*s3*(qdd(1) + qdd(2)) + s3*(0.00163355*c4*(c3*(qdd(1) + qdd(2)) - qd(3)*s3*(qd(1) + qd(2))) + 0.00950111*c4*(c3*qd(3)*(qd(1) + qd(2)) + s3*(qdd(1) + qdd(2))) + c4*(0.000409305*c5*(-qdd(3) + qdd(4)) + 0.00151607*c5*(c4*(c3*qd(3)*(qd(1) + qd(2)) + s3*(qdd(1) + qdd(2))) + qd(4)*(-c3*c4*(qd(1) + qd(2)) - s3*s4*(qd(1) + qd(2))) - s4*(c3*(qdd(1) + qdd(2)) - qd(3)*s3*(qd(1) + qd(2)))) + c5*(6.20477e-6*c6*(c5*(c4*(c3*qd(3)*(qd(1) + qd(2)) + s3*(qdd(1) + qdd(2))) + qd(4)*(-c3*c4*(qd(1) + qd(2)) - s3*s4*(qd(1) + qd(2))) - s4*(c3*(qdd(1) + qdd(2)) - qd(3)*s3*(qd(1) + qd(2)))) + qd(5)*(-c5*(-qd(3) + qd(4)) - s5*(-c3*s4*(qd(1) + qd(2)) + c4*s3*(qd(1) + qd(2)))) - s5*(-qdd(3) + qdd(4))) + 6.20477e-6*qd(6)*(-c6*(-c5*(-qd(3) + qd(4)) - s5*(-c3*s4*(qd(1) + qd(2)) + c4*s3*(qd(1) + qd(2)))) - s6*(c5*(-c3*s4*(qd(1) + qd(2)) + c4*s3*(qd(1) + qd(2))) - s5*(-qd(3) + qd(4)))) - 6.20477e-6*s6*(-c5*(-qdd(3) + qdd(4)) - qd(5)*(c5*(-c3*s4*(qd(1) + qd(2)) + c4*s3*(qd(1) + qd(2))) - s5*(-qd(3) + qd(4))) - s5*(c4*(c3*qd(3)*(qd(1) + qd(2)) + s3*(qdd(1) + qdd(2))) + qd(4)*(-c3*c4*(qd(1) + qd(2)) - s3*s4*(qd(1) + qd(2))) - s4*(c3*(qdd(1) + qdd(2)) - qd(3)*s3*(qd(1) + qd(2))))) + (-c6*(-c5*(-qd(3) + qd(4)) - s5*(-c3*s4*(qd(1) + qd(2)) + c4*s3*(qd(1) + qd(2)))) - s6*(c5*(-c3*s4*(qd(1) + qd(2)) + c4*s3*(qd(1) + qd(2))) - s5*(-qd(3) + qd(4))))*(3.29301e-6*c3*c4*(qd(1) + qd(2)) - 3.29301e-6*qd(5) + 3.29301e-6*qd(6) + 3.29301e-6*s3*s4*(qd(1) + qd(2))) - (-3.01352e-6*c6*(-c5*(-qd(3) + qd(4)) - s5*(-c3*s4*(qd(1) + qd(2)) + c4*s3*(qd(1) + qd(2)))) - 3.01352e-6*s6*(c5*(-c3*s4*(qd(1) + qd(2)) + c4*s3*(qd(1) + qd(2))) - s5*(-qd(3) + qd(4))))*(c3*c4*(qd(1) + qd(2)) - qd(5) + qd(6) + s3*s4*(qd(1) + qd(2)))) + 295*m6*(-c5*(-c2*(-c1*g + 270*qdd(1)) - 295*c3^2*(qd(1) + qd(2)) ^2 - 90*qdd(1) - 90*qdd(2) + s2*(-g*s1 - 270*qd(1)^2) - 295*s3^2*(qd(1) + qd(2)) ^2) - s5*(c4*(-295*c3*(qdd(1) + qdd(2)) + c3*(c2*(-g*s1 - 270*qd(1)^2) + s2*(-c1*g + 270*qdd(1)) - (qd(1) + qd(2))*(90*qd(1) + 90*qd(2)))) - s4*(295*s3*(qdd(1) + qdd(2)) - s3*(c2*(-g*s1 - 270*qd(1)^2) + s2*(-c1*g + 270*qdd(1)) - (qd(1) + qd(2))*(90*qd(1) + 90*qd(2)))))) + 295*m7*(c4*(295*s3*(qdd(1) + qdd(2)) - s3*(c2*(-g*s1 - 270*qd(1)^2) + s2*(-c1*g + 270*qdd(1)) - (qd(1) + qd(2))*(90*qd(1) + 90*qd(2)))) + s4*(-295*c3*(qdd(1) + qdd(2)) + c3*(c2*(-g*s1 - 270*qd(1)^2) + s2*(-c1*g + 270*qdd(1)) - (qd(1) + qd(2))*(90*qd(1) + 90*qd(2)))) + (-c5*(-qd(3) + qd(4)) - s5*(-c3*s4*(qd(1) + qd(2)) + c4*s3*(qd(1) + qd(2))))*(80*c5*(-qd(3) + qd(4)) + 80*s5*(-c3*s4*(qd(1) + qd(2)) + c4*s3*(qd(1) + qd(2)))) - (c5*(-c3*s4*(qd(1) + qd(2)) + c4*s3*(qd(1) + qd(2))) - s5*(-qd(3) + qd(4)))*(80*c5*(-c3*s4*(qd(1) + qd(2)) + c4*s3*(qd(1) + qd(2))) - 80*s5*(-qd(3) + qd(4))) - (-c6*(-c5*(-qd(3) + qd(4)) - s5*(-c3*s4*(qd(1) + qd(2)) + c4*s3*(qd(1) + qd(2)))) - s6*(c5*(-c3*s4*(qd(1) + qd(2)) + c4*s3*(qd(1) + qd(2))) - s5*(-qd(3) + qd(4))))*(80*c6*(-c5*(-qd(3) + qd(4)) - s5*(-c3*s4*(qd(1) + qd(2)) + c4*s3*(qd(1) + qd(2)))) + 80*s6*(c5*(-c3*s4*(qd(1) + qd(2)) + c4*s3*(qd(1) + qd(2))) - s5*(-qd(3) + qd(4)))) + (c6*(c5*(-c3*s4*(qd(1) + qd(2)) + c4*s3*(qd(1) + qd(2))) - s5*(-qd(3) + qd(4))) - s6*(-c5*(-qd(3) + qd(4)) - s5*(-c3*s4*(qd(1) + qd(2)) + c4*s3*(qd(1) + qd(2)))))*(80*c6*(c5*(-c3*s4*(qd(1) + qd(2)) + c4*s3*(qd(1) + qd(2))) - s5*(-qd(3) + qd(4))) - 80*s6*(-c5*(-qd(3) + qd(4)) - s5*(-c3*s4*(qd(1) + qd(2)) + c4*s3*(qd(1) + qd(2)))))) + 0.00151607*qd(5)*(-c5*(-qd(3) + qd(4)) - s5*(-c3*s4*(qd(1) + qd(2)) + c4*s3*(qd(1) + qd(2)))) + 0.000409305*qd(5)*(c5*(-c3*s4*(qd(1) + qd(2)) + c4*s3*(qd(1) + qd(2))) - s5*(-qd(3) + qd(4))) - 0.00151607*s5*(-qdd(3) + qdd(4)) + 0.000409305*s5*(c4*(c3*qd(3)*(qd(1) + qd(2)) + s3*(qdd(1) + qdd(2))) + qd(4)*(-c3*c4*(qd(1) + qd(2)) - s3*s4*(qd(1) + qd(2))) - s4*(c3*(qdd(1) + qdd(2)) - qd(3)*s3*(qd(1) + qd(2)))) - s5*(-3.01352e-6*c6*(-c5*(-qdd(3) + qdd(4)) - qd(5)*(c5*(-c3*s4*(qd(1) + qd(2)) + c4*s3*(qd(1) + qd(2))) - s5*(-qd(3) + qd(4))) - s5*(c4*(c3*qd(3)*(qd(1) + qd(2)) + s3*(qdd(1) + qdd(2))) + qd(4)*(-c3*c4*(qd(1) + qd(2)) - s3*s4*(qd(1) + qd(2))) - s4*(c3*(qdd(1) + qdd(2)) - qd(3)*s3*(qd(1) + qd(2))))) - 3.01352e-6*qd(6)*(c6*(c5*(-c3*s4*(qd(1) + qd(2)) + c4*s3*(qd(1) + qd(2))) - s5*(-qd(3) + qd(4))) - s6*(-c5*(-qd(3) + qd(4)) - s5*(-c3*s4*(qd(1) + qd(2)) + c4*s3*(qd(1) + qd(2))))) - 3.01352e-6*s6*(c5*(c4*(c3*qd(3)*(qd(1) + qd(2)) + s3*(qdd(1) + qdd(2))) + qd(4)*(-c3*c4*(qd(1) + qd(2)) - s3*s4*(qd(1) + qd(2))) - s4*(c3*(qdd(1) + qdd(2)) - qd(3)*s3*(qd(1) + qd(2)))) + qd(5)*(-c5*(-qd(3) + qd(4)) - s5*(-c3*s4*(qd(1) + qd(2)) + c4*s3*(qd(1) + qd(2)))) - s5*(-qdd(3) + qdd(4))) + (6.20477e-6*c6*(c5*(-c3*s4*(qd(1) + qd(2)) + c4*s3*(qd(1) + qd(2))) - s5*(-qd(3) + qd(4))) - 6.20477e-6*s6*(-c5*(-qd(3) + qd(4)) - s5*(-c3*s4*(qd(1) + qd(2)) + c4*s3*(qd(1) + qd(2)))))*(c3*c4*(qd(1) + qd(2)) - qd(5) + qd(6) + s3*s4*(qd(1) + qd(2))) - (c6*(c5*(-c3*s4*(qd(1) + qd(2)) + c4*s3*(qd(1) + qd(2))) - s5*(-qd(3) + qd(4))) - s6*(-c5*(-qd(3) + qd(4)) - s5*(-c3*s4*(qd(1) + qd(2)) + c4*s3*(qd(1) + qd(2)))))*(3.29301e-6*c3*c4*(qd(1) + qd(2)) - 3.29301e-6*qd(5) + 3.29301e-6*qd(6) + 3.29301e-6*s3*s4*(qd(1) + qd(2)))) + (-c5*(-qd(3) + qd(4)) - s5*(-c3*s4*(qd(1) + qd(2)) + c4*s3*(qd(1) + qd(2))))*(-0.00358942*c3*c4*(qd(1) + qd(2)) + 0.00358942*qd(5) - 0.00358942*s3*s4*(qd(1) + qd(2))) - (-c3*c4*(qd(1) + qd(2)) + qd(5) - s3*s4*(qd(1) + qd(2)))*(-0.00355535*c5*(-qd(3) + qd(4)) - 0.000409305*c5*(-c3*s4*(qd(1) + qd(2)) + c4*s3*(qd(1) + qd(2))) + 0.000409305*s5*(-qd(3) + qd(4)) - 0.00355535*s5*(-c3*s4*(qd(1) + qd(2)) + c4*s3*(qd(1) + qd(2))))) + 0.00950111*qd(4)*(-c3*c4*(qd(1) + qd(2)) - s3*s4*(qd(1) + qd(2))) + 0.00163355*qd(4)*(-c3*s4*(qd(1) + qd(2)) + c4*s3*(qd(1) + qd(2))) + 8.41256e-6*qdd(3) - 8.41256e-6*qdd(4) - 0.00950111*s4*(c3*(qdd(1) + qdd(2)) - qd(3)*s3*(qd(1) + qd(2))) + 0.00163355*s4*(c3*qd(3)*(qd(1) + qd(2)) + s3*(qdd(1) + qdd(2))) - s4*(3.29301e-6*c4*(c3*(qdd(1) + qdd(2)) - qd(3)*s3*(qd(1) + qd(2))) - 295*c5*m7*(80*c6*(-c5*(-qdd(3) + qdd(4)) - qd(5)*(c5*(-c3*s4*(qd(1) + qd(2)) + c4*s3*(qd(1) + qd(2))) - s5*(-qd(3) + qd(4))) - s5*(c4*(c3*qd(3)*(qd(1) + qd(2)) + s3*(qdd(1) + qdd(2))) + qd(4)*(-c3*c4*(qd(1) + qd(2)) - s3*s4*(qd(1) + qd(2))) - s4*(c3*(qdd(1) + qdd(2)) - qd(3)*s3*(qd(1) + qd(2))))) + c6*(80*c5*(-qdd(3) + qdd(4)) + c5*(c4*(-295*c3*(qdd(1) + qdd(2)) + c3*(c2*(-g*s1 - 270*qd(1)^2) + s2*(-c1*g + 270*qdd(1)) - (qd(1) + qd(2))*(90*qd(1) + 90*qd(2)))) - s4*(295*s3*(qdd(1) + qdd(2)) - s3*(c2*(-g*s1 - 270*qd(1)^2) + s2*(-c1*g + 270*qdd(1)) - (qd(1) + qd(2))*(90*qd(1) + 90*qd(2))))) + 80*qd(5)*(c5*(-c3*s4*(qd(1) + qd(2)) + c4*s3*(qd(1) + qd(2))) - s5*(-qd(3) + qd(4))) + 80*s5*(c4*(c3*qd(3)*(qd(1) + qd(2)) + s3*(qdd(1) + qdd(2))) + qd(4)*(-c3*c4*(qd(1) + qd(2)) - s3*s4*(qd(1) + qd(2))) - s4*(c3*(qdd(1) + qdd(2)) - qd(3)*s3*(qd(1) + qd(2)))) - s5*(-c2*(-c1*g + 270*qdd(1)) - 295*c3^2*(qd(1) + qd(2)) ^2 - 90*qdd(1) - 90*qdd(2) + s2*(-g*s1 - 270*qd(1)^2) - 295*s3^2*(qd(1) + qd(2)) ^2) - (80*c5*(-c3*s4*(qd(1) + qd(2)) + c4*s3*(qd(1) + qd(2))) - 80*s5*(-qd(3) + qd(4)))*(-c3*c4*(qd(1) + qd(2)) + qd(5) - s3*s4*(qd(1) + qd(2)))) + 80*qd(6)*(c6*(c5*(-c3*s4*(qd(1) + qd(2)) + c4*s3*(qd(1) + qd(2))) - s5*(-qd(3) + qd(4))) - s6*(-c5*(-qd(3) + qd(4)) - s5*(-c3*s4*(qd(1) + qd(2)) + c4*s3*(qd(1) + qd(2))))) + 80*s6*(c5*(c4*(c3*qd(3)*(qd(1) + qd(2)) + s3*(qdd(1) + qdd(2))) + qd(4)*(-c3*c4*(qd(1) + qd(2)) - s3*s4*(qd(1) + qd(2))) - s4*(c3*(qdd(1) + qdd(2)) - qd(3)*s3*(qd(1) + qd(2)))) + qd(5)*(-c5*(-qd(3) + qd(4)) - s5*(-c3*s4*(qd(1) + qd(2)) + c4*s3*(qd(1) + qd(2)))) - s5*(-qdd(3) + qdd(4))) - s6*(80*c5*(c4*(c3*qd(3)*(qd(1) + qd(2)) + s3*(qdd(1) + qdd(2))) + qd(4)*(-c3*c4*(qd(1) + qd(2)) - s3*s4*(qd(1) + qd(2))) - s4*(c3*(qdd(1) + qdd(2)) - qd(3)*s3*(qd(1) + qd(2)))) - c5*(-c2*(-c1*g + 270*qdd(1)) - 295*c3^2*(qd(1) + qd(2)) ^2 - 90*qdd(1) - 90*qdd(2) + s2*(-g*s1 - 270*qd(1)^2) - 295*s3^2*(qd(1) + qd(2)) ^2) + 80*qd(5)*(-c5*(-qd(3) + qd(4)) - s5*(-c3*s4*(qd(1) + qd(2)) + c4*s3*(qd(1) + qd(2)))) - 80*s5*(-qdd(3) + qdd(4)) - s5*(c4*(-295*c3*(qdd(1) + qdd(2)) + c3*(c2*(-g*s1 - 270*qd(1)^2) + s2*(-c1*g + 270*qdd(1)) - (qd(1) + qd(2))*(90*qd(1) + 90*qd(2)))) - s4*(295*s3*(qdd(1) + qdd(2)) - s3*(c2*(-g*s1 - 270*qd(1)^2+ s2*(-c1*g + 270*qdd(1)) - (qd(1) + qd(2))*(90*qd(1) + 90*qd(2))))) + (80*c5*(-qd(3) + qd(4)) + 80*s5*(-c3*s4*(qd(1) + qd(2)) + c4*s3*(qd(1) + qd(2))))*(-c3*c4*(qd(1) + qd(2)) + qd(5) - s3*s4*(qd(1) + qd(2)))) - (80*c6*(c5*(-c3*s4*(qd(1) + qd(2)) + c4*s3*(qd(1) + qd(2))) - s5*(-qd(3) + qd(4))) - 80*s6*(-c5*(-qd(3) + qd(4)) - s5*(-c3*s4*(qd(1) + qd(2)) + c4*s3*(qd(1) + qd(2)))))*(c3*c4*(qd(1) + qd(2)) - qd(5) + qd(6) + s3*s4*(qd(1) + qd(2)))) - 0.00355535*c5*(-qdd(3) + qdd(4)) - 0.000409305*c5*(c4*(c3*qd(3)*(qd(1) + qd(2)) + s3*(qdd(1) + qdd(2))) + qd(4)*(-c3*c4*(qd(1) + qd(2)) - s3*s4*(qd(1) + qd(2))) - s4*(c3*(qdd(1) + qdd(2)) - qd(3)*s3*(qd(1) + qd(2)))) - 295*m6*(c5*(c4*(-295*c3*(qdd(1) + qdd(2)) + c3*(c2*(-g*s1 - 270*qd(1)^2) + s2*(-c1*g + 270*qdd(1)) - (qd(1) + qd(2))*(90*qd(1) + 90*qd(2)))) - s4*(295*s3*(qdd(1) + qdd(2)) - s3*(c2*(-g*s1 - 270*qd(1)^2) + s2*(-c1*g + 270*qdd(1)) - (qd(1) + qd(2))*(90*qd(1) + 90*qd(2))))) - s5*(-c2*(-c1*g + 270*qdd(1)) - 295*c3^2*(qd(1) + qd(2)) ^2- 90*qdd(1) - 90*qdd(2) + s2*(-g*s1 - 270*qd(1)^2) - 295*s3^2*(qd(1) + qd(2)) ^2)) + 295*m7*s5*(80*c6*(c5*(c4*(c3*qd(3)*(qd(1) + qd(2)) + s3*(qdd(1) + qdd(2))) + qd(4)*(-c3*c4*(qd(1) + qd(2)) - s3*s4*(qd(1) + qd(2))) - s4*(c3*(qdd(1) + qdd(2)) - qd(3)*s3*(qd(1) + qd(2)))) + qd(5)*(-c5*(-qd(3) + qd(4)) - s5*(-c3*s4*(qd(1) + qd(2)) + c4*s3*(qd(1) + qd(2)))) - s5*(-qdd(3) + qdd(4))) - c6*(80*c5*(c4*(c3*qd(3)*(qd(1) + qd(2)) + s3*(qdd(1) + qdd(2))) + qd(4)*(-c3*c4*(qd(1) + qd(2)) - s3*s4*(qd(1) + qd(2))) - s4*(c3*(qdd(1) + qdd(2)) - qd(3)*s3*(qd(1) + qd(2)))) - c5*(-c2*(-c1*g + 270*qdd(1)) - 295*c3^2*(qd(1) + qd(2)) ^2 - 90*qdd(1) - 90*qdd(2) + s2*(-g*s1 - 270*qd(1)^2) - 295*s3^2*(qd(1) + qd(2)) ^2) + 80*qd(5)*(-c5*(-qd(3) + qd(4)) - s5*(-c3*s4*(qd(1) + qd(2)) + c4*s3*(qd(1) + qd(2)))) - 80*s5*(-qdd(3) + qdd(4)) - s5*(c4*(-295*c3*(qdd(1) + qdd(2)) + c3*(c2*(-g*s1 - 270*qd(1)^2) + s2*(-c1*g + 270*qdd(1)) - (qd(1) + qd(2))*(90*qd(1) + 90*qd(2)))) - s4*(295*s3*(qdd(1) + qdd(2)) - s3*(c2*(-g*s1 - 270*qd(1)^2) + s2*(-c1*g + 270*qdd(1)) - (qd(1) + qd(2))*(90*qd(1) + 90*qd(2))))) + (80*c5*(-qd(3) + qd(4)) + 80*s5*(-c3*s4*(qd(1) + qd(2)) + c4*s3*(qd(1) + qd(2))))*(-c3*c4*(qd(1) + qd(2)) + qd(5) - s3*s4*(qd(1) + qd(2)))) + 80*qd(6)*(-c6*(-c5*(-qd(3) + qd(4)) - s5*(-c3*s4*(qd(1) + qd(2)) + c4*s3*(qd(1) + qd(2)))) - s6*(c5*(-c3*s4*(qd(1) + qd(2)) + c4*s3*(qd(1) + qd(2))) - s5*(-qd(3) + qd(4)))) - 80*s6*(-c5*(-qdd(3) + qdd(4)) - qd(5)*(c5*(-c3*s4*(qd(1) + qd(2)) + c4*s3*(qd(1) + qd(2))) - s5*(-qd(3) + qd(4))) - s5*(c4*(c3*qd(3)*(qd(1) + qd(2)) + s3*(qdd(1) + qdd(2))) + qd(4)*(-c3*c4*(qd(1) + qd(2)) - s3*s4*(qd(1) + qd(2))) - s4*(c3*(qdd(1) + qdd(2)) - qd(3)*s3*(qd(1) + qd(2))))) - s6*(80*c5*(-qdd(3) + qdd(4)) + c5*(c4*(-295*c3*(qdd(1) + qdd(2)) + c3*(c2*(-g*s1 - 270*qd(1)^2) + s2*(-c1*g + 270*qdd(1)) - (qd(1) + qd(2))*(90*qd(1) + 90*qd(2)))) - s4*(295*s3*(qdd(1) + qdd(2)) - s3*(c2*(-g*s1 - 270*qd(1)^2) + s2*(-c1*g + 270*qdd(1)) - (qd(1) + qd(2))*(90*qd(1) + 90*qd(2))))) + 80*qd(5)*(c5*(-c3*s4*(qd(1) + qd(2)) + c4*s3*(qd(1) + qd(2))) - s5*(-qd(3) + qd(4))) + 80*s5*(c4*(c3*qd(3)*(qd(1) + qd(2)) + s3*(qdd(1) + qdd(2))) + qd(4)*(-c3*c4*(qd(1) + qd(2)) - s3*s4*(qd(1) + qd(2))) - s4*(c3*(qdd(1) + qdd(2)) - qd(3)*s3*(qd(1) + qd(2)))) - s5*(-c2*(-c1*g + 270*qdd(1)) - 295*c3^2*(qd(1) + qd(2)) ^2 - 90*qdd(1) - 90*qdd(2) + s2*(-g*s1 - 270*qd(1)^2) - 295*s3^2*(qd(1) + qd(2)) ^2) - (80*c5*(-c3*s4*(qd(1) + qd(2)) + c4*s3*(qd(1) + qd(2))) - 80*s5*(-qd(3) + qd(4)))*(-c3*c4*(qd(1) + qd(2)) + qd(5) - s3*s4*(qd(1) + qd(2)))) + (80*c6*(-c5*(-qd(3) + qd(4)) - s5*(-c3*s4*(qd(1) + qd(2)) + c4*s3*(qd(1) + qd(2)))) + 80*s6*(c5*(-c3*s4*(qd(1) + qd(2)) + c4*s3*(qd(1) + qd(2))) - s5*(-qd(3) + qd(4))))*(c3*c4*(qd(1) + qd(2)) - qd(5) + qd(6) + s3*s4*(qd(1) + qd(2)))) + 3.29301e-6*qd(4)*(-c3*s4*(qd(1) + qd(2)) + c4*s3*(qd(1) + qd(2))) - 0.000409305*qd(5)*(-c5*(-qd(3) + qd(4)) - s5*(-c3*s4*(qd(1) + qd(2)) + c4*s3*(qd(1) + qd(2)))) - 0.00355535*qd(5)*(c5*(-c3*s4*(qd(1) + qd(2)) + c4*s3*(qd(1) + qd(2))) - s5*(-qd(3) + qd(4))) - 3.29301e-6*qdd(5) + 3.29301e-6*qdd(6) + 3.29301e-6*s4*(c3*qd(3)*(qd(1) + qd(2)) + s3*(qdd(1) + qdd(2))) + 0.000409305*s5*(-qdd(3) + qdd(4)) - 0.00355535*s5*(c4*(c3*qd(3)*(qd(1) + qd(2)) + s3*(qdd(1) + qdd(2))) + qd(4)*(-c3*c4*(qd(1) + qd(2)) - s3*s4*(qd(1) + qd(2))) - s4*(c3*(qdd(1) + qdd(2)) - qd(3)*s3*(qd(1) + qd(2)))) - (c5*(-c3*s4*(qd(1) + qd(2)) + c4*s3*(qd(1) + qd(2))) - s5*(-qd(3) + qd(4)))*(-0.00358942*c3*c4*(qd(1) + qd(2)) + 0.00358942*qd(5) - 0.00358942*s3*s4*(qd(1) + qd(2))) - (-c6*(-c5*(-qd(3) + qd(4)) - s5*(-c3*s4*(qd(1) + qd(2)) + c4*s3*(qd(1) + qd(2)))) - s6*(c5*(-c3*s4*(qd(1) + qd(2)) + c4*s3*(qd(1) + qd(2))) - s5*(-qd(3) + qd(4))))*(6.20477e-6*c6*(c5*(-c3*s4*(qd(1) + qd(2)) + c4*s3*(qd(1) + qd(2))) - s5*(-qd(3) + qd(4))) - 6.20477e-6*s6*(-c5*(-qd(3) + qd(4)) - s5*(-c3*s4*(qd(1) + qd(2)) + c4*s3*(qd(1) + qd(2))))) + (-3.01352e-6*c6*(-c5*(-qd(3) + qd(4)) - s5*(-c3*s4*(qd(1) + qd(2)) + c4*s3*(qd(1) + qd(2)))) - 3.01352e-6*s6*(c5*(-c3*s4*(qd(1) + qd(2)) + c4*s3*(qd(1) + qd(2))) - s5*(-qd(3) + qd(4))))*(c6*(c5*(-c3*s4*(qd(1) + qd(2)) + c4*s3*(qd(1) + qd(2))) - s5*(-qd(3) + qd(4))) - s6*(-c5*(-qd(3) + qd(4)) - s5*(-c3*s4*(qd(1) + qd(2)) + c4*s3*(qd(1) + qd(2))))) + (-c3*c4*(qd(1) + qd(2)) + qd(5) - s3*s4*(qd(1) + qd(2)))*(0.000409305*c5*(-qd(3) + qd(4)) + 0.00151607*c5*(-c3*s4*(qd(1) + qd(2)) + c4*s3*(qd(1) + qd(2))) - 0.00151607*s5*(-qd(3) + qd(4)) + 0.000409305*s5*(-c3*s4*(qd(1) + qd(2)) + c4*s3*(qd(1) + qd(2))))) - (-qd(3) + qd(4))*(-0.020170031*c3*c4*(qd(1) + qd(2)) + 0.00163355*c3*s4*(qd(1) + qd(2)) - 0.00163355*c4*s3*(qd(1) + qd(2)) + 2.69102e-6*qd(3) - 2.69102e-6*qd(4) - 0.020170031*s3*s4*(qd(1) + qd(2))) + (-c3*c4*(qd(1) + qd(2)) - s3*s4*(qd(1) + qd(2)))*(2.69102e-6*c3*c4*(qd(1) + qd(2)) + 8.41256e-6*c3*s4*(qd(1) + qd(2)) - 8.41256e-6*c4*s3*(qd(1) + qd(2)) - 0.024130024*qd(3) + 0.024130024*qd(4) + 2.69102e-6*s3*s4*(qd(1) + qd(2))))));
%  
% tau3 = 0.00359211102*c4*(c3*(qdd(1) + qdd(2)) - qd(3)*s3*(qd(1) + qd(2))) - 90*c4*(m6*(-c5*(-c2*(-c1*g + 270*qdd(1)) - 295*c3^2*(qd(1) + qd(2)) ^2 - 90*qdd(1) - 90*qdd(2) + s2*(-g*s1 - 270*qd(1)^2) - 295*s3^2*(qd(1) + qd(2)) ^2) - s5*(c4*(-295*c3*(qdd(1) + qdd(2)) + c3*(c2*(-g*s1 - 270*qd(1)^2) + s2*(-c1*g + 270*qdd(1)) - (qd(1) + qd(2))*(90*qd(1) + 90*qd(2)))) - s4*(295*s3*(qdd(1) + qdd(2)) - s3*(c2*(-g*s1 - 270*qd(1)^2) + s2*(-c1*g + 270*qdd(1)) - (qd(1) + qd(2))*(90*qd(1) + 90*qd(2)))))) + m7*(c4*(295*s3*(qdd(1) + qdd(2)) - s3*(c2*(-g*s1 - 270*qd(1)^2) + s2*(-c1*g + 270*qdd(1)) - (qd(1) + qd(2))*(90*qd(1) + 90*qd(2)))) + s4*(-295*c3*(qdd(1) + qdd(2)) + c3*(c2*(-g*s1 - 270*qd(1)^2) + s2*(-c1*g + 270*qdd(1)) - (qd(1) + qd(2))*(90*qd(1) + 90*qd(2)))) + (-c5*(-qd(3) + qd(4)) - s5*(-c3*s4*(qd(1) + qd(2)) + c4*s3*(qd(1) + qd(2))))*(80*c5*(-qd(3) + qd(4)) + 80*s5*(-c3*s4*(qd(1) + qd(2)) + c4*s3*(qd(1) + qd(2)))) - (c5*(-c3*s4*(qd(1) + qd(2)) + c4*s3*(qd(1) + qd(2))) - s5*(-qd(3) + qd(4)))*(80*c5*(-c3*s4*(qd(1) + qd(2)) + c4*s3*(qd(1) + qd(2))) - 80*s5*(-qd(3) + qd(4))) - (-c6*(-c5*(-qd(3) + qd(4)) - s5*(-c3*s4*(qd(1) + qd(2)) + c4*s3*(qd(1) + qd(2)))) - s6*(c5*(-c3*s4*(qd(1) + qd(2)) + c4*s3*(qd(1) + qd(2))) - s5*(-qd(3) + qd(4))))*(80*c6*(-c5*(-qd(3) + qd(4)) - s5*(-c3*s4*(qd(1) + qd(2)) + c4*s3*(qd(1) + qd(2)))) + 80*s6*(c5*(-c3*s4*(qd(1) + qd(2)) + c4*s3*(qd(1) + qd(2))) - s5*(-qd(3) + qd(4)))) + (c6*(c5*(-c3*s4*(qd(1) + qd(2)) + c4*s3*(qd(1) + qd(2))) - s5*(-qd(3) + qd(4))) - s6*(-c5*(-qd(3) + qd(4)) - s5*(-c3*s4*(qd(1) + qd(2)) + c4*s3*(qd(1) + qd(2)))))*(80*c6*(c5*(-c3*s4*(qd(1) + qd(2)) + c4*s3*(qd(1) + qd(2))) - s5*(-qd(3) + qd(4))) - 80*s6*(-c5*(-qd(3) + qd(4)) - s5*(-c3*s4*(qd(1) + qd(2)) + c4*s3*(qd(1) + qd(2))))))) - 8.41256e-6*c4*(c3*qd(3)*(qd(1) + qd(2)) + s3*(qdd(1) + qdd(2))) + c5*(-3.01352e-6*c6*(-c5*(-qdd(3) + qdd(4)) - qd(5)*(c5*(-c3*s4*(qd(1) + qd(2)) + c4*s3*(qd(1) + qd(2))) - s5*(-qd(3) + qd(4))) - s5*(c4*(c3*qd(3)*(qd(1) + qd(2)) + s3*(qdd(1) + qdd(2))) + qd(4)*(-c3*c4*(qd(1) + qd(2)) - s3*s4*(qd(1) + qd(2))) - s4*(c3*(qdd(1) + qdd(2)) - qd(3)*s3*(qd(1) + qd(2))))) - 3.01352e-6*qd(6)*(c6*(c5*(-c3*s4*(qd(1) + qd(2)) + c4*s3*(qd(1) + qd(2))) - s5*(-qd(3) + qd(4))) - s6*(-c5*(-qd(3) + qd(4)) - s5*(-c3*s4*(qd(1) + qd(2)) + c4*s3*(qd(1) + qd(2))))) - 3.01352e-6*s6*(c5*(c4*(c3*qd(3)*(qd(1) + qd(2)) + s3*(qdd(1) + qdd(2))) + qd(4)*(-c3*c4*(qd(1) + qd(2)) - s3*s4*(qd(1) + qd(2))) - s4*(c3*(qdd(1) + qdd(2)) - qd(3)*s3*(qd(1) + qd(2)))) + qd(5)*(-c5*(-qd(3) + qd(4)) - s5*(-c3*s4*(qd(1) + qd(2)) + c4*s3*(qd(1) + qd(2)))) - s5*(-qdd(3) + qdd(4))) + (6.20477e-6*c6*(c5*(-c3*s4*(qd(1) + qd(2)) + c4*s3*(qd(1) + qd(2))) - s5*(-qd(3) + qd(4))) - 6.20477e-6*s6*(-c5*(-qd(3) + qd(4)) - s5*(-c3*s4*(qd(1) + qd(2)) + c4*s3*(qd(1) + qd(2)))))*(c3*c4*(qd(1) + qd(2)) - qd(5) + qd(6) + s3*s4*(qd(1) + qd(2))) - (c6*(c5*(-c3*s4*(qd(1) + qd(2)) + c4*s3*(qd(1) + qd(2))) - s5*(-qd(3) + qd(4))) - s6*(-c5*(-qd(3) + qd(4)) - s5*(-c3*s4*(qd(1) + qd(2)) + c4*s3*(qd(1) + qd(2)))))*(3.29301e-6*c3*c4*(qd(1) + qd(2)) - 3.29301e-6*qd(5) + 3.29301e-6*qd(6) + 3.29301e-6*s3*s4*(qd(1) + qd(2)))) + 90*m5*(-c4*(295*s3*(qdd(1) + qdd(2)) - s3*(c2*(-g*s1 - 270*qd(1)^2) + s2*(-c1*g + 270*qdd(1)) - (qd(1) + qd(2))*(90*qd(1) + 90*qd(2)))) + 295*c4*(c3*qd(3)*(qd(1) + qd(2)) + s3*(qdd(1) + qdd(2))) + 295*qd(4)*(-c3*c4*(qd(1) + qd(2)) - s3*s4*(qd(1) + qd(2))) - s4*(-295*c3*(qdd(1) + qdd(2)) + c3*(c2*(-g*s1 - 270*qd(1)^2) + s2*(-c1*g + 270*qdd(1)) - (qd(1) + qd(2))*(90*qd(1) + 90*qd(2)))) - 295*s4*(c3*(qdd(1) + qdd(2)) - qd(3)*s3*(qd(1) + qd(2))) + (-qd(3) + qd(4))*(295*c3*c4*(qd(1) + qd(2)) + 295*s3*s4*(qd(1) + qd(2)))) - 8.41256e-6*qd(4)*(-c3*c4*(qd(1) + qd(2)) - s3*s4*(qd(1) + qd(2))) + 0.00359211102*qd(4)*(-c3*s4*(qd(1) + qd(2)) + c4*s3*(qd(1) + qd(2))) - 0.024130024*qdd(3) + 0.024130024*qdd(4) - 0.00358942*qdd(5) + 8.41256e-6*s4*(c3*(qdd(1) + qdd(2)) - qd(3)*s3*(qd(1) + qd(2))) + 0.00359211102*s4*(c3*qd(3)*(qd(1) + qd(2)) + s3*(qdd(1) + qdd(2))) - 90*s4*(c5*m7*(80*c6*(-c5*(-qdd(3) + qdd(4)) - qd(5)*(c5*(-c3*s4*(qd(1) + qd(2)) + c4*s3*(qd(1) + qd(2))) - s5*(-qd(3) + qd(4))) - s5*(c4*(c3*qd(3)*(qd(1) + qd(2)) + s3*(qdd(1) + qdd(2))) + qd(4)*(-c3*c4*(qd(1) + qd(2)) - s3*s4*(qd(1) + qd(2))) - s4*(c3*(qdd(1) + qdd(2)) - qd(3)*s3*(qd(1) + qd(2))))) + c6*(80*c5*(-qdd(3) + qdd(4)) + c5*(c4*(-295*c3*(qdd(1) + qdd(2)) + c3*(c2*(-g*s1 - 270*qd(1)^2) + s2*(-c1*g + 270*qdd(1)) - (qd(1) + qd(2))*(90*qd(1) + 90*qd(2)))) - s4*(295*s3*(qdd(1) + qdd(2)) - s3*(c2*(-g*s1 - 270*qd(1)^2) + s2*(-c1*g + 270*qdd(1)) - (qd(1) + qd(2))*(90*qd(1) + 90*qd(2))))) + 80*qd(5)*(c5*(-c3*s4*(qd(1) + qd(2)) + c4*s3*(qd(1) + qd(2))) - s5*(-qd(3) + qd(4))) + 80*s5*(c4*(c3*qd(3)*(qd(1) + qd(2)) + s3*(qdd(1) + qdd(2))) + qd(4)*(-c3*c4*(qd(1) + qd(2)) - s3*s4*(qd(1) + qd(2))) - s4*(c3*(qdd(1) + qdd(2)) - qd(3)*s3*(qd(1) + qd(2)))) - s5*(-c2*(-c1*g + 270*qdd(1)) - 295*c3^2*(qd(1) + qd(2)) ^2 - 90*qdd(1) - 90*qdd(2) + s2*(-g*s1 - 270*qd(1)^2) - 295*s3^2*(qd(1) + qd(2)) ^2) - (80*c5*(-c3*s4*(qd(1) + qd(2)) + c4*s3*(qd(1) + qd(2))) - 80*s5*(-qd(3) + qd(4)))*(-c3*c4*(qd(1) + qd(2)) + qd(5) - s3*s4*(qd(1) + qd(2)))) + 80*qd(6)*(c6*(c5*(-c3*s4*(qd(1) + qd(2)) + c4*s3*(qd(1) + qd(2))) - s5*(-qd(3) + qd(4))) - s6*(-c5*(-qd(3) + qd(4)) - s5*(-c3*s4*(qd(1) + qd(2)) + c4*s3*(qd(1) + qd(2))))) + 80*s6*(c5*(c4*(c3*qd(3)*(qd(1) + qd(2)) + s3*(qdd(1) + qdd(2))) + qd(4)*(-c3*c4*(qd(1) + qd(2)) - s3*s4*(qd(1) + qd(2))) - s4*(c3*(qdd(1) + qdd(2)) - qd(3)*s3*(qd(1) + qd(2)))) + qd(5)*(-c5*(-qd(3) + qd(4)) - s5*(-c3*s4*(qd(1) + qd(2)) + c4*s3*(qd(1) + qd(2)))) - s5*(-qdd(3) + qdd(4))) - s6*(80*c5*(c4*(c3*qd(3)*(qd(1) + qd(2)) + s3*(qdd(1) + qdd(2))) + qd(4)*(-c3*c4*(qd(1) + qd(2)) - s3*s4*(qd(1) + qd(2))) - s4*(c3*(qdd(1) + qdd(2)) - qd(3)*s3*(qd(1) + qd(2)))) - c5*(-c2*(-c1*g + 270*qdd(1)) - 295*c3^2*(qd(1) + qd(2)) ^2 - 90*qdd(1) - 90*qdd(2) + s2*(-g*s1 - 270*qd(1)^2) - 295*s3^2*(qd(1) + qd(2)) ^2) + 80*qd(5)*(-c5*(-qd(3) + qd(4)) - s5*(-c3*s4*(qd(1) + qd(2)) + c4*s3*(qd(1) + qd(2)))) - 80*s5*(-qdd(3) + qdd(4)) - s5*(c4*(-295*c3*(qdd(1) + qdd(2)) + c3*(c2*(-g*s1 - 270*qd(1)^2) + s2*(-c1*g + 270*qdd(1)) - (qd(1) + qd(2))*(90*qd(1) + 90*qd(2)))) - s4*(295*s3*(qdd(1) + qdd(2)) - s3*(c2*(-g*s1 - 270*qd(1)^2) + s2*(-c1*g + 270*qdd(1)) - (qd(1) + qd(2))*(90*qd(1) + 90*qd(2))))) + (80*c5*(-qd(3) + qd(4)) + 80*s5*(-c3*s4*(qd(1) + qd(2)) + c4*s3*(qd(1) + qd(2))))*(-c3*c4*(qd(1) + qd(2)) + qd(5) - s3*s4*(qd(1) + qd(2)))) - (80*c6*(c5*(-c3*s4*(qd(1) + qd(2)) + c4*s3*(qd(1) + qd(2))) - s5*(-qd(3) + qd(4))) - 80*s6*(-c5*(-qd(3) + qd(4)) - s5*(-c3*s4*(qd(1) + qd(2)) + c4*s3*(qd(1) + qd(2)))))*(c3*c4*(qd(1) + qd(2)) - qd(5) + qd(6) + s3*s4*(qd(1) + qd(2)))) + m6*(c5*(c4*(-295*c3*(qdd(1) + qdd(2)) + c3*(c2*(-g*s1 - 270*qd(1)^2) + s2*(-c1*g + 270*qdd(1)) - (qd(1) + qd(2))*(90*qd(1) + 90*qd(2)))) - s4*(295*s3*(qdd(1) + qdd(2)) - s3*(c2*(-g*s1 - 270*qd(1)^2) + s2*(-c1*g + 270*qdd(1)) - (qd(1) + qd(2))*(90*qd(1) + 90*qd(2))))) - s5*(-c2*(-c1*g + 270*qdd(1)) - 295*c3^2*(qd(1) + qd(2)) ^2 - 90*qdd(1) - 90*qdd(2) + s2*(-g*s1 - 270*qd(1)^2) - 295*s3^2*(qd(1) + qd(2)) ^2)) - m7*s5*(80*c6*(c5*(c4*(c3*qd(3)*(qd(1) + qd(2)) + s3*(qdd(1) + qdd(2))) + qd(4)*(-c3*c4*(qd(1) + qd(2)) - s3*s4*(qd(1) + qd(2))) - s4*(c3*(qdd(1) + qdd(2)) - qd(3)*s3*(qd(1) + qd(2)))) + qd(5)*(-c5*(-qd(3) + qd(4)) - s5*(-c3*s4*(qd(1) + qd(2)) + c4*s3*(qd(1) + qd(2)))) - s5*(-qdd(3) + qdd(4))) - c6*(80*c5*(c4*(c3*qd(3)*(qd(1) + qd(2)) + s3*(qdd(1) + qdd(2))) + qd(4)*(-c3*c4*(qd(1) + qd(2)) - s3*s4*(qd(1) + qd(2))) - s4*(c3*(qdd(1) + qdd(2)) - qd(3)*s3*(qd(1) + qd(2)))) - c5*(-c2*(-c1*g + 270*qdd(1)) - 295*c3^2*(qd(1) + qd(2)) ^2 - 90*qdd(1) - 90*qdd(2) + s2*(-g*s1 - 270*qd(1)^2) - 295*s3^2*(qd(1) + qd(2)) ^2) + 80*qd(5)*(-c5*(-qd(3) + qd(4)) - s5*(-c3*s4*(qd(1) + qd(2)) + c4*s3*(qd(1) + qd(2)))) - 80*s5*(-qdd(3) + qdd(4)) - s5*(c4*(-295*c3*(qdd(1) + qdd(2)) + c3*(c2*(-g*s1 - 270*qd(1)^2) + s2*(-c1*g + 270*qdd(1)) - (qd(1) + qd(2))*(90*qd(1) + 90*qd(2)))) - s4*(295*s3*(qdd(1) + qdd(2)) - s3*(c2*(-g*s1 - 270*qd(1)^2) + s2*(-c1*g + 270*qdd(1)) - (qd(1) + qd(2))*(90*qd(1) + 90*qd(2))))) + (80*c5*(-qd(3) + qd(4)) + 80*s5*(-c3*s4*(qd(1) + qd(2)) + c4*s3*(qd(1) + qd(2))))*(-c3*c4*(qd(1) + qd(2)) + qd(5) - s3*s4*(qd(1) + qd(2)))) + 80*qd(6)*(-c6*(-c5*(-qd(3) + qd(4)) - s5*(-c3*s4*(qd(1) + qd(2)) + c4*s3*(qd(1) + qd(2)))) - s6*(c5*(-c3*s4*(qd(1) + qd(2)) + c4*s3*(qd(1) + qd(2))) - s5*(-qd(3) + qd(4)))) - 80*s6*(-c5*(-qdd(3) + qdd(4)) - qd(5)*(c5*(-c3*s4*(qd(1) + qd(2)) + c4*s3*(qd(1) + qd(2))) - s5*(-qd(3) + qd(4))) - s5*(c4*(c3*qd(3)*(qd(1) + qd(2)) + s3*(qdd(1) + qdd(2))) + qd(4)*(-c3*c4*(qd(1) + qd(2)) - s3*s4*(qd(1) + qd(2))) - s4*(c3*(qdd(1) + qdd(2)) - qd(3)*s3*(qd(1) + qd(2))))) - s6*(80*c5*(-qdd(3) + qdd(4)) + c5*(c4*(-295*c3*(qdd(1) + qdd(2)) + c3*(c2*(-g*s1 - 270*qd(1)^2) + s2*(-c1*g + 270*qdd(1)) - (qd(1) + qd(2))*(90*qd(1) + 90*qd(2)))) - s4*(295*s3*(qdd(1) + qdd(2)) - s3*(c2*(-g*s1 - 270*qd(1)^2) + s2*(-c1*g + 270*qdd(1)) - (qd(1) + qd(2))*(90*qd(1) + 90*qd(2))))) + 80*qd(5)*(c5*(-c3*s4*(qd(1) + qd(2)) + c4*s3*(qd(1) + qd(2))) - s5*(-qd(3) + qd(4))) + 80*s5*(c4*(c3*qd(3)*(qd(1) + qd(2)) + s3*(qdd(1) + qdd(2))) + qd(4)*(-c3*c4*(qd(1) + qd(2)) - s3*s4*(qd(1) + qd(2))) - s4*(c3*(qdd(1) + qdd(2)) - qd(3)*s3*(qd(1) + qd(2)))) - s5*(-c2*(-c1*g + 270*qdd(1)) - 295*c3^2*(qd(1) + qd(2)) ^2 - 90*qdd(1) - 90*qdd(2) + s2*(-g*s1 - 270*qd(1)^2) - 295*s3^2*(qd(1) + qd(2)) ^2) - (80*c5*(-c3*s4*(qd(1) + qd(2)) + c4*s3*(qd(1) + qd(2))) - 80*s5*(-qd(3) + qd(4)))*(-c3*c4*(qd(1) + qd(2)) + qd(5) - s3*s4*(qd(1) + qd(2)))) + (80*c6*(-c5*(-qd(3) + qd(4)) - s5*(-c3*s4*(qd(1) + qd(2)) + c4*s3*(qd(1) + qd(2)))) + 80*s6*(c5*(-c3*s4*(qd(1) + qd(2)) + c4*s3*(qd(1) + qd(2))) - s5*(-qd(3) + qd(4))))*(c3*c4*(qd(1) + qd(2)) - qd(5) + qd(6) + s3*s4*(qd(1) + qd(2))))) + s5*(6.20477e-6*c6*(c5*(c4*(c3*qd(3)*(qd(1) + qd(2)) + s3*(qdd(1) + qdd(2))) + qd(4)*(-c3*c4*(qd(1) + qd(2)) - s3*s4*(qd(1) + qd(2))) - s4*(c3*(qdd(1) + qdd(2)) - qd(3)*s3*(qd(1) + qd(2)))) + qd(5)*(-c5*(-qd(3) + qd(4)) - s5*(-c3*s4*(qd(1) + qd(2)) + c4*s3*(qd(1) + qd(2)))) - s5*(-qdd(3) + qdd(4))) + 6.20477e-6*qd(6)*(-c6*(-c5*(-qd(3) + qd(4)) - s5*(-c3*s4*(qd(1) + qd(2)) + c4*s3*(qd(1) + qd(2)))) - s6*(c5*(-c3*s4*(qd(1) + qd(2)) + c4*s3*(qd(1) + qd(2))) - s5*(-qd(3) + qd(4)))) - 6.20477e-6*s6*(-c5*(-qdd(3) + qdd(4)) - qd(5)*(c5*(-c3*s4*(qd(1) + qd(2)) + c4*s3*(qd(1) + qd(2))) - s5*(-qd(3) + qd(4))) - s5*(c4*(c3*qd(3)*(qd(1) + qd(2)) + s3*(qdd(1) + qdd(2))) + qd(4)*(-c3*c4*(qd(1) + qd(2)) - s3*s4*(qd(1) + qd(2))) - s4*(c3*(qdd(1) + qdd(2)) - qd(3)*s3*(qd(1) + qd(2))))) + (-c6*(-c5*(-qd(3) + qd(4)) - s5*(-c3*s4*(qd(1) + qd(2)) + c4*s3*(qd(1) + qd(2)))) - s6*(c5*(-c3*s4*(qd(1) + qd(2)) + c4*s3*(qd(1) + qd(2))) - s5*(-qd(3) + qd(4))))*(3.29301e-6*c3*c4*(qd(1) + qd(2)) - 3.29301e-6*qd(5) + 3.29301e-6*qd(6) + 3.29301e-6*s3*s4*(qd(1) + qd(2))) - (-3.01352e-6*c6*(-c5*(-qd(3) + qd(4)) - s5*(-c3*s4*(qd(1) + qd(2)) + c4*s3*(qd(1) + qd(2)))) - 3.01352e-6*s6*(c5*(-c3*s4*(qd(1) + qd(2)) + c4*s3*(qd(1) + qd(2))) - s5*(-qd(3) + qd(4))))*(c3*c4*(qd(1) + qd(2)) - qd(5) + qd(6) + s3*s4*(qd(1) + qd(2)))) + (-c5*(-qd(3) + qd(4)) - s5*(-c3*s4*(qd(1) + qd(2)) + c4*s3*(qd(1) + qd(2))))*(0.000409305*c5*(-qd(3) + qd(4)) + 0.00151607*c5*(-c3*s4*(qd(1) + qd(2)) + c4*s3*(qd(1) + qd(2))) - 0.00151607*s5*(-qd(3) + qd(4)) + 0.000409305*s5*(-c3*s4*(qd(1) + qd(2)) + c4*s3*(qd(1) + qd(2)))) - (c5*(-c3*s4*(qd(1) + qd(2)) + c4*s3*(qd(1) + qd(2))) - s5*(-qd(3) + qd(4)))*(-0.00355535*c5*(-qd(3) + qd(4)) - 0.000409305*c5*(-c3*s4*(qd(1) + qd(2)) + c4*s3*(qd(1) + qd(2))) + 0.000409305*s5*(-qd(3) + qd(4)) - 0.00355535*s5*(-c3*s4*(qd(1) + qd(2)) + c4*s3*(qd(1) + qd(2)))) - (-c3*c4*(qd(1) + qd(2)) - s3*s4*(qd(1) + qd(2)))*(0.00163355*c3*c4*(qd(1) + qd(2)) - 0.00950111*c3*s4*(qd(1) + qd(2)) + 0.00950111*c4*s3*(qd(1) + qd(2)) + 8.41256e-6*qd(3) - 8.41256e-6*qd(4) + 0.00163355*s3*s4*(qd(1) + qd(2))) + (-c3*s4*(qd(1) + qd(2)) + c4*s3*(qd(1) + qd(2)))*(-0.020170031*c3*c4*(qd(1) + qd(2)) + 0.00163355*c3*s4*(qd(1) + qd(2)) - 0.00163355*c4*s3*(qd(1) + qd(2)) + 2.69102e-6*qd(3) - 2.69102e-6*qd(4) - 0.020170031*s3*s4*(qd(1) + qd(2)));
%  
